simulink model "SwarmSystem"  (R2022b)
(part 2 of 4)

  Record : Record  RecordToWorkspace=on  FileSettingsInternal="{\"entries\":[{\"content\":{\"excelSettings\":{\"content\":{},\"type\":\"Streamout.ExcelSettings\"}},\"type\":\"Streamout.FileSettingStorage\",\"uuid\":\"ecd064a0-1818-44c3-a92e-bae1736691b7\"}],\"packageUris\":[\"http://schema.mathworks.com/mf0/streamout_blocks/R2020a\"],\"version\":\"1.0\"}"  SignalsInternal="{\"entries\":[{\"content\":{\"signals\":[{\"content\":{\"blockPath\":[\"SwarmSystem/Record\"],\"channel\":[],\"dimensions\":[54,1],\"domain\":\"SwarmSystem/Record\",\"hasChildren\":true,\"lineColor\":\"#fe330a\",\"plots\":[],\"port\":1,\"sid\":[\"\"],\"signalID\":5288,\"signalName\":\"z\"},\"type\":\"RecordBlkView.Signal\",\"uuid\":\"1048f33c-cd0c-4b1c-99d7-4ac97ea90ab0\"},{\"content\":{\"blockPath\":[\"SwarmSystem/Record\"],\"channel\":[1,1],\"dimensions\":[54,1],\"domain\":\"SwarmSystem/Record\",\"lineColor\":\"#7e2f8e\",\"parentID\":5288,\"plots\":[1],\"port\":1,\"sid\":[\"\"],\"signalID\":5289,\"signalName\":\"z\"},\"type\":\"RecordBlkView.Signal\",\"uuid\":\"d4620c93-bf21-47de-89ed-4dbaaf8b8520\"},{\"content\":{\"blockPath\":[\"SwarmSystem/Record\"],\"channel\":[],\"dimensions\":[36,1],\"domain\":\"SwarmSystem/Record\",\"hasChildren\":true,\"lineColor\":\"#0072bd\",\"plots\":[],\"port\":2,\"sid\":[\"\"],\"signalID\":5293,\"signalName\":\"z_d\"},\"type\":\"RecordBlkView.Signal\",\"uuid\":\"b35ab5d5-7ee7-45a1-a41b-38fccb067dc1\"},{\"content\":{\"blockPath\":[\"SwarmSystem/Record\"],\"channel\":[1,1],\"dimensions\":[36,1],\"domain\":\"SwarmSystem/Record\",\"lineColor\":\"#77ac30\",\"parentID\":5293,\"plots\":[1],\"port\":2,\"sid\":[\"\"],\"signalID\":5294,\"signalName\":\"z_d\"},\"type\":\"RecordBlkView.Signal\",\"uuid\":\"879ab91b-c74b-4204-85a0-6ebafe84b3f1\"},{\"content\":{\"blockPath\":[\"SwarmSystem/Record\"],\"channel\":[],\"dimensions\":[9,1],\"domain\":\"SwarmSystem/Record\",\"hasChildren\":true,\"lineColor\":\"#edb120\",\"plots\":[],\"port\":3,\"sid\":[\"\"],\"signalID\":5298,\"signalName\":\"Z_esp\"},\"type\":\"RecordBlkView.Signal\",\"uuid\":\"96b793c3-32b0-46bc-a925-f10905e3ac7d\"},{\"content\":{\"blockPath\":[\"SwarmSystem/Record\"],\"channel\":[1,1],\"dimensions\":[9,1],\"domain\":\"SwarmSystem/Record\",\"lineColor\":\"#64d413\",\"parentID\":5298,\"plots\":[1],\"port\":3,\"sid\":[\"\"],\"signalID\":5299,\"signalName\":\"Z_esp\"},\"type\":\"RecordBlkView.Signal\",\"uuid\":\"46fa4c9b-8c9c-4ead-9f2c-4953bb52642d\"},{\"content\":{\"blockPath\":[\"SwarmSystem/Record\"],\"channel\":[],\"dimensions\":[1],\"domain\":\"SwarmSystem/Record\",\"lineColor\":\"#ff6929\",\"plots\":[1],\"port\":4,\"sid\":[\"\"],\"signalID\":5303,\"signalName\":\"increment\"},\"type\":\"RecordBlkView.Signal\",\"uuid\":\"5359e2d5-ef0a-482c-b34d-73c89588b715\"},{\"content\":{\"blockPath\":[\"SwarmSystem/Record\"],\"channel\":[],\"dimensions\":[9,4],\"domain\":\"SwarmSystem/Record\",\"hasChildren\":true,\"lineColor\":\"#4dbeee\",\"plots\":[],\"port\":5,\"sid\":[\"\"],\"signalID\":5307,\"signalName\":\"bounds\"},\"type\":\"RecordBlkView.Signal\",\"uuid\":\"1b31fc5b-037d-49c7-bff4-18edc4567836\"},{\"content\":{\"blockPath\":[\"SwarmSystem/Record\"],\"channel\":[1,1],\"dimensions\":[9,4],\"domain\":\"SwarmSystem/Record\",\"lineColor\":\"#22b573\",\"parentID\":5307,\"plots\":[1],\"port\":5,\"sid\":[\"\"],\"signalID\":5308,\"signalName\":\"bounds\"},\"type\":\"RecordBlkView.Signal\",\"uuid\":\"eb4c524e-ff5c-4dd1-a222-fb6ffedcee01\"},{\"content\":{\"blockPath\":[\"SwarmSystem/Record\"],\"channel\":[],\"dimensions\":[1],\"domain\":\"SwarmSystem/Record\",\"lineColor\":\"#64d413\",\"plots\":[1],\"port\":6,\"sid\":[\"\"],\"signalID\":5312,\"signalName\":\"time\"},\"type\":\"RecordBlkView.Signal\",\"uuid\":\"72dfbc7d-692b-40af-bae7-eb77a350f7e6\"},{\"content\":{\"blockPath\":[\"SwarmSystem/Record\"],\"channel\":[],\"dimensions\":[9,27],\"domain\":\"SwarmSystem/Record\",\"hasChildren\":true,\"lineColor\":\"#ff6929\",\"plots\":[],\"port\":7,\"sid\":[\"\"],\"signalID\":5316,\"signalName\":\"raw\"},\"type\":\"RecordBlkView.Signal\",\"uuid\":\"f96d5ccb-5004-4439-9612-791f3ef51b61\"},{\"content\":{\"blockPath\":[\"SwarmSystem/Record\"],\"channel\":[1,1],\"dimensions\":[9,27],\"domain\":\"SwarmSystem/Record\",\"lineColor\":\"#edb120\",\"parentID\":5316,\"plots\":[1],\"port\":7,\"sid\":[\"\"],\"signalID\":5317,\"signalName\":\"raw\"},\"type\":\"RecordBlkView.Signal\",\"uuid\":\"bfe1e9cf-bb17-4b73-b5c0-09a8e8591fff\"},{\"content\":{\"blockPath\":[\"SwarmSystem/Record\"],\"channel\":[],\"dimensions\":[9,1],\"domain\":\"SwarmSystem/Record\",\"hasChildren\":true,\"lineColor\":\"#64d413\",\"plots\":[],\"port\":8,\"sid\":[\"\"],\"signalID\":5321,\"signalName\":\"sat_order\"},\"type\":\"RecordBlkView.Signal\",\"uuid\":\"3c0b71d5-5553-4668-91be-6a5fb8ab4b43\"},{\"content\":{\"blockPath\":[\"SwarmSystem/Record\"],\"channel\":[1,1],\"dimensions\":[9,1],\"domain\":\"SwarmSystem/Record\",\"lineColor\":\"#77ac30\",\"parentID\":5321,\"plots\":[1],\"port\":8,\"sid\":[\"\"],\"signalID\":5322,\"signalName\":\"sat_order\"},\"type\":\"RecordBlkView.Signal\",\"uuid\":\"ccf7dce6-4af8-4663-9d88-9176ee7af16e\"},{\"content\":{\"blockPath\":[\"SwarmSystem/Record\"],\"channel\":[],\"dimensions\":[9,9,3],\"domain\":\"SwarmSystem/Record\",\"hasChildren\":true,\"lineColor\":\"#fe330a\",\"plots\":[],\"port\":9,\"sid\":[\"\"],\"signalID\":5326,\"signalName\":\"packed_tw\"},\"type\":\"RecordBlkView.Signal\",\"uuid\":\"04cd0336-9984-42b6-950b-aadca579e03d\"},{\"content\":{\"blockPath\":[\"SwarmSystem/Record\"],\"channel\":[1,1,1],\"dimensions\":[9,9,3],\"domain\":\"SwarmSystem/Record\",\"lineColor\":\"#a2142f\",\"parentID\":5326,\"plots\":[1],\"port\":9,\"sid\":[\"\"],\"signalID\":5327,\"signalName\":\"packed_tw\"},\"type\":\"RecordBlkView.Signal\",\"uuid\":\"538a1e68-288b-4ad8-b1d1-6395bf7ee774\"},{\"content\":{\"blockPath\":[\"SwarmSystem/Record\"],\"channel\":[],\"dimensions\":[9,9,3,3],\"domain\":\"SwarmSystem/Record\",\"hasChildren\":true,\"lineColor\":\"#0072bd\",\"plots\":[],\"port\":10,\"sid\":[\"\"],\"signalID\":5331,\"signalName\":\"packed_intersections\"},\"type\":\"RecordBlkView.Signal\",\"uuid\":\"144e32b6-4e64-4aac-921a-80a3c9570e69\"},{\"content\":{\"blockPath\":[\"SwarmSystem/Record\"],\"channel\":[1,1,1,1],\"dimensions\":[9,9,3,3],\"domain\":\"SwarmSystem/Record\",\"lineColor\":\"#139fff\",\"parentID\":5331,\"plots\":[1],\"port\":10,\"sid\":[\"\"],\"signalID\":5332,\"signalName\":\"packed_intersections\"},\"type\":\"RecordBlkView.Signal\",\"uuid\":\"e33d14f4-2dcf-4038-900f-7b110429d0f7\"},{\"content\":{\"blockPath\":[\"SwarmSystem/Record\"],\"channel\":[2,1],\"dimensions\":[54,1],\"domain\":\"SwarmSystem/Record\",\"lineColor\":\"#64d413\",\"parentID\":5288,\"plots\":[1],\"port\":1,\"sid\":[\"\"],\"signalID\":5337,\"signalName\":\"z\"},\"type\":\"RecordBlkView.Signal\",\"uuid\":\"94ff7854-8769-4ec7-b8e0-c41f290a7d05\"},{\"content\":{\"blockPath\":[\"SwarmSystem/Record\"],\"channel\":[3,1],\"dimensions\":[54,1],\"domain\":\"SwarmSystem/Record\",\"lineColor\":\"#ff13a6\",\"parentID\":5288,\"plots\":[1],\"port\":1,\"sid\":[\"\"],\"signalID\":5338,\"signalName\":\"z\"},\"type\":\"RecordBlkView.Signal\",\"uuid\":\"55582deb-032f-45c7-978e-d388079c41d4\"},{\"content\":{\"blockPath\":[\"SwarmSystem/Record\"],\"channel\":[4,1],\"dimensions\":[54,1],\"domain\":\"SwarmSystem/Record\",\"lineColor\":\"#fe330a\",\"parentID\":5288,\"plots\":[1],\"port\":1,\"sid\":[\"\"],\"signalID\":5339,\"signalName\":\"z\"},\"type\":\"RecordBlkView.Signal\",\"uuid\":\"c5e6b669-41d4-4e1e-a17b-50be0138714a\"},{\"content\":{\"blockPath\":[\"SwarmSystem/Record\"],\"channel\":[5,1],\"dimensions\":[54,1],\"domain\":\"SwarmSystem/Record\",\"lineColor\":\"#22b573\",\"parentID\":5288,\"plots\":[],\"port\":1,\"sid\":[\"\"],\"signalID\":5340,\"signalName\":\"z\"},\"type\":\"RecordBlkView.Signal\",\"uuid\":\"b4ce17a2-064b-424c-b87d-5e710a343d57\"},{\"content\":{\"blockPath\":[\"SwarmSystem/Record\"],\"channel\":[6,1],\"dimensions\":[54,1],\"domain\":\"SwarmSystem/Record\",\"lineColor\":\"#0072bd\",\"parentID\":5288,\"plots\":[],\"port\":1,\"sid\":[\"\"],\"signalID\":5341,\"signalName\":\"z\"},\"type\":\"RecordBlkView.Signal\",\"uuid\":\"f998aeda-c207-47e4-835e-c5bd924f8b22\"},{\"content\":{\"blockPath\":[\"SwarmSystem/Record\"],\"channel\":[7,1],\"dimensions\":[54,1],\"domain\":\"SwarmSystem/Record\",\"lineColor\":\"#d95319\",\"parentID\":5288,\"plots\":[],\"port\":1,\"sid\":[\"\"],\"signalID\":5342,\"signalName\":\"z\"},\"type\":\"RecordBlkView.Signal\",\"uuid\":\"33bed8e9-bcc4-478e-8b0a-051153d0a6e0\"},{\"content\":{\"blockPath\":[\"SwarmSystem/Record\"],\"channel\":[8,1],\"dimensions\":[54,1],\"domain\":\"SwarmSystem/Record\",\"lineColor\":\"#edb120\",\"parentID\":5288,\"plots\":[],\"port\":1,\"sid\":[\"\"],\"signalID\":5343,\"signalName\":\"z\"},\"type\":\"RecordBlkView.Signal\",\"uuid\":\"23367080-42e0-4bda-822e-26e9880913c3\"},{\"content\":{\"blockPath\":[\"SwarmSystem/Record\"],\"channel\":[9,1],\"dimensions\":[54,1],\"domain\":\"SwarmSystem/Record\",\"lineColor\":\"#7e2f8e\",\"parentID\":5288,\"plots\":[],\"port\":1,\"sid\":[\"\"],\"signalID\":5344,\"signalName\":\"z\"},\"type\":\"RecordBlkView.Signal\",\"uuid\":\"666db174-2bf7-46d0-8a11-19612ed523fd\"},{\"content\":{\"blockPath\":[\"SwarmSystem/Record\"],\"channel\":[10,1],\"dimensions\":[54,1],\"domain\":\"SwarmSystem/Record\",\"lineColor\":\"#77ac30\",\"parentID\":5288,\"plots\":[],\"port\":1,\"sid\":[\"\"],\"signalID\":5345,\"signalName\":\"z\"},\"type\":\"RecordBlkView.Signal\",\"uuid\":\"d56b95aa-f617-4b7e-b38c-c508357e2a07\"},{\"content\":{\"blockPath\":[\"SwarmSystem/Record\"],\"channel\":[11,1],\"dimensions\":[54,1],\"domain\":\"SwarmSystem/Record\",\"lineColor\":\"#4dbeee\",\"parentID\":5288,\"plots\":[],\"port\":1,\"sid\":[\"\"],\"signalID\":5346,\"signalName\":\"z\"},\"type\":\"RecordBlkView.Signal\",\"uuid\":\"3c739fc7-8c37-4b5e-bb88-9d6524bd94ac\"},{\"content\":{\"blockPath\":[\"SwarmSystem/Record\"],\"channel\":[12,1],\"dimensions\":[54,1],\"domain\":\"SwarmSystem/Record\",\"lineColor\":\"#a2142f\",\"parentID\":5288,\"plots\":[],\"port\":1,\"sid\":[\"\"],\"signalID\":5347,\"signalName\":\"z\"},\"type\":\"RecordBlkView.Signal\",\"uuid\":\"2aa2a071-04ed-43fe-bed0-8f31fcee10da\"},{\"content\":{\"blockPath\":[\"SwarmSystem/Record\"],\"channel\":[13,1],\"dimensions\":[54,1],\"domain\":\"SwarmSystem/Record\",\"lineColor\":\"#139fff\",\"parentID\":5288,\"plots\":[],\"port\":1,\"sid\":[\"\"],\"signalID\":5348,\"signalName\":\"z\"},\"type\":\"RecordBlkView.Signal\",\"uuid\":\"af55a24b-ba08-4c59-88b6-de72df1b84e0\"},{\"content\":{\"blockPath\":[\"SwarmSystem/Record\"],\"channel\":[14,1],\"dimensions\":[54,1],\"domain\":\"SwarmSystem/Record\",\"lineColor\":\"#ff6929\",\"parentID\":5288,\"plots\":[],\"port\":1,\"sid\":[\"\"],\"signalID\":5349,\"signalName\":\"z\"},\"type\":\"RecordBlkView.Signal\",\"uuid\":\"1a6bf3ba-172b-41ef-a20a-2928397536b8\"},{\"content\":{\"blockPath\":[\"SwarmSystem/Record\"],\"channel\":[15,1],\"dimensions\":[54,1],\"domain\":\"SwarmSystem/Record\",\"lineColor\":\"#b746ff\",\"parentID\":5288,\"plots\":[],\"port\":1,\"sid\":[\"\"],\"signalID\":5350,\"signalName\":\"z\"},\"type\":\"RecordBlkView.Signal\",\"uuid\":\"cbf6ef62-eef2-4671-ba0b-33c28c49ded4\"},{\"content\":{\"blockPath\":[\"SwarmSystem/Record\"],\"channel\":[16,1],\"dimensions\":[54,1],\"domain\":\"SwarmSystem/Record\",\"lineColor\":\"#64d413\",\"parentID\":5288,\"plots\":[],\"port\":1,\"sid\":[\"\"],\"signalID\":5351,\"signalName\":\"z\"},\"type\":\"RecordBlkView.Signal\",\"uuid\":\"60424ef6-59ac-4762-8308-f2e8899aee2f\"},{\"content\":{\"blockPath\":[\"SwarmSystem/Record\"],\"channel\":[17,1],\"dimensions\":[54,1],\"domain\":\"SwarmSystem/Record\",\"lineColor\":\"#ff13a6\",\"parentID\":5288,\"plots\":[],\"port\":1,\"sid\":[\"\"],\"signalID\":5352,\"signalName\":\"z\"},\"type\":\"RecordBlkView.Signal\",\"uuid\":\"693ba6bc-14a8-4cd8-ab9b-fb1a45bae915\"},{\"content\":{\"blockPath\":[\"SwarmSystem/Record\"],\"channel\":[18,1],\"dimensions\":[54,1],\"domain\":\"SwarmSystem/Record\",\"lineColor\":\"#fe330a\",\"parentID\":5288,\"plots\":[],\"port\":1,\"sid\":[\"\"],\"signalID\":5353,\"signalName\":\"z\"},\"type\":\"RecordBlkView.Signal\",\"uuid\":\"85c5cfdb-b89a-4d6f-846d-6d1b25df3ce5\"},{\"content\":{\"blockPath\":[\"SwarmSystem/Record\"],\"channel\":[19,1],\"dimensions\":[54,1],\"domain\":\"SwarmSystem/Record\",\"lineColor\":\"#22b573\",\"parentID\":5288,\"plots\":[],\"port\":1,\"sid\":[\"\"],\"signalID\":5354,\"signalName\":\"z\"},\"type\":\"RecordBlkView.Signal\",\"uuid\":\"a606537b-4093-4b5b-8ba0-a895a02fc9ad\"},{\"content\":{\"blockPath\":[\"SwarmSystem/Record\"],\"channel\":[20,1],\"dimensions\":[54,1],\"domain\":\"SwarmSystem/Record\",\"lineColor\":\"#0072bd\",\"parentID\":5288,\"plots\":[],\"port\":1,\"sid\":[\"\"],\"signalID\":5355,\"signalName\":\"z\"},\"type\":\"RecordBlkView.Signal\",\"uuid\":\"d92b94f0-0096-476a-8397-e0938e33775d\"},{\"content\":{\"blockPath\":[\"SwarmSystem/Record\"],\"channel\":[21,1],\"dimensions\":[54,1],\"domain\":\"SwarmSystem/Record\",\"lineColor\":\"#d95319\",\"parentID\":5288,\"plots\":[],\"port\":1,\"sid\":[\"\"],\"signalID\":5356,\"signalName\":\"z\"},\"type\":\"RecordBlkView.Signal\",\"uuid\":\"53771d3f-3b29-417b-8dfe-8d61cc1d6a74\"},{\"content\":{\"blockPath\":[\"SwarmSystem/Record\"],\"channel\":[22,1],\"dimensions\":[54,1],\"domain\":\"SwarmSystem/Record\",\"lineColor\":\"#edb120\",\"parentID\":5288,\"plots\":[],\"port\":1,\"sid\":[\"\"],\"signalID\":5357,\"signalName\":\"z\"},\"type\":\"RecordBlkView.Signal\",\"uuid\":\"77a86afe-249a-40e4-933a-6b90270a3c5f\"},{\"content\":{\"blockPath\":[\"SwarmSystem/Record\"],\"channel\":[23,1],\"dimensions\":[54,1],\"domain\":\"SwarmSystem/Record\",\"lineColor\":\"#7e2f8e\",\"parentID\":5288,\"plots\":[],\"port\":1,\"sid\":[\"\"],\"signalID\":5358,\"signalName\":\"z\"},\"type\":\"RecordBlkView.Signal\",\"uuid\":\"71145ac7-7da5-4009-917a-f802b7d56a90\"},{\"content\":{\"blockPath\":[\"SwarmSystem/Record\"],\"channel\":[24,1],\"dimensions\":[54,1],\"domain\":\"SwarmSystem/Record\",\"lineColor\":\"#77ac30\",\"parentID\":5288,\"plots\":[],\"port\":1,\"sid\":[\"\"],\"signalID\":5359,\"signalName\":\"z\"},\"type\":\"RecordBlkView.Signal\",\"uuid\":\"a1777b40-0222-4109-b320-ffa96848db97\"},{\"content\":{\"blockPath\":[\"SwarmSystem/Record\"],\"channel\":[25,1],\"dimensions\":[54,1],\"domain\":\"SwarmSystem/Record\",\"lineColor\":\"#4dbeee\",\"parentID\":5288,\"plots\":[],\"port\":1,\"sid\":[\"\"],\"signalID\":5360,\"signalName\":\"z\"},\"type\":\"RecordBlkView.Signal\",\"uuid\":\"f0aa7a69-251b-47b1-b73c-85a4efe9d20c\"},{\"content\":{\"blockPath\":[\"SwarmSystem/Record\"],\"channel\":[26,1],\"dimensions\":[54,1],\"domain\":\"SwarmSystem/Record\",\"lineColor\":\"#a2142f\",\"parentID\":5288,\"plots\":[],\"port\":1,\"sid\":[\"\"],\"signalID\":5361,\"signalName\":\"z\"},\"type\":\"RecordBlkView.Signal\",\"uuid\":\"651f1bdc-b6dc-49af-bcc7-1437cdcaa17a\"},{\"content\":{\"blockPath\":[\"SwarmSystem/Record\"],\"channel\":[27,1],\"dimensions\":[54,1],\"domain\":\"SwarmSystem/Record\",\"lineColor\":\"#139fff\",\"parentID\":5288,\"plots\":[],\"port\":1,\"sid\":[\"\"],\"signalID\":5362,\"signalName\":\"z\"},\"type\":\"RecordBlkView.Signal\",\"uuid\":\"b7136c86-a499-4bc3-8659-50e8c5b58c3e\"},{\"content\":{\"blockPath\":[\"SwarmSystem/Record\"],\"channel\":[28,1],\"dimensions\":[54,1],\"domain\":\"SwarmSystem/Record\",\"lineColor\":\"#ff6929\",\"parentID\":5288,\"plots\":[],\"port\":1,\"sid\":[\"\"],\"signalID\":5363,\"signalName\":\"z\"},\"type\":\"RecordBlkView.Signal\",\"uuid\":\"39ed0c79-0ead-4119-98ea-487db81751da\"},{\"content\":{\"blockPath\":[\"SwarmSystem/Record\"],\"channel\":[29,1],\"dimensions\":[54,1],\"domain\":\"SwarmSystem/Record\",\"lineColor\":\"#b746ff\",\"parentID\":5288,\"plots\":[],\"port\":1,\"sid\":[\"\"],\"signalID\":5364,\"signalName\":\"z\"},\"type\":\"RecordBlkView.Signal\",\"uuid\":\"eab1f46b-145f-4fba-b506-cef354494f10\"},{\"content\":{\"blockPath\":[\"SwarmSystem/Record\"],\"channel\":[30,1],\"dimensions\":[54,1],\"domain\":\"SwarmSystem/Record\",\"lineColor\":\"#64d413\",\"parentID\":5288,\"plots\":[],\"port\":1,\"sid\":[\"\"],\"signalID\":5365,\"signalName\":\"z\"},\"type\":\"RecordBlkView.Signal\",\"uuid\":\"7bb013dd-5e1d-44ea-99f4-ae20af2f8ed1\"},{\"content\":{\"blockPath\":[\"SwarmSystem/Record\"],\"channel\":[31,1],\"dimensions\":[54,1],\"domain\":\"SwarmSystem/Record\",\"lineColor\":\"#ff13a6\",\"parentID\":5288,\"plots\":[],\"port\":1,\"sid\":[\"\"],\"signalID\":5366,\"signalName\":\"z\"},\"type\":\"RecordBlkView.Signal\",\"uuid\":\"bcc6f70b-8549-4e7b-8798-9fe58ee725e6\"},{\"content\":{\"blockPath\":[\"SwarmSystem/Record\"],\"channel\":[32,1],\"dimensions\":[54,1],\"domain\":\"SwarmSystem/Record\",\"lineColor\":\"#fe330a\",\"parentID\":5288,\"plots\":[],\"port\":1,\"sid\":[\"\"],\"signalID\":5367,\"signalName\":\"z\"},\"type\":\"RecordBlkView.Signal\",\"uuid\":\"1d770efc-4041-4ff2-a64a-e334b80ba3c3\"},{\"content\":{\"blockPath\":[\"SwarmSystem/Record\"],\"channel\":[33,1],\"dimensions\":[54,1],\"domain\":\"SwarmSystem/Record\",\"lineColor\":\"#22b573\",\"parentID\":5288,\"plots\":[],\"port\":1,\"sid\":[\"\"],\"signalID\":5368,\"signalName\":\"z\"},\"type\":\"RecordBlkView.Signal\",\"uuid\":\"4affd0bd-477a-4ba8-927f-f2cd7de50b25\"},{\"content\":{\"blockPath\":[\"SwarmSystem/Record\"],\"channel\":[34,1],\"dimensions\":[54,1],\"domain\":\"SwarmSystem/Record\",\"lineColor\":\"#0072bd\",\"parentID\":5288,\"plots\":[],\"port\":1,\"sid\":[\"\"],\"signalID\":5369,\"signalName\":\"z\"},\"type\":\"RecordBlkView.Signal\",\"uuid\":\"c22acc9d-ab4f-4cbd-ac54-90ec6f71b885\"},{\"content\":{\"blockPath\":[\"SwarmSystem/Record\"],\"channel\":[35,1],\"dimensions\":[54,1],\"domain\":\"SwarmSystem/Record\",\"lineColor\":\"#d95319\",\"parentID\":5288,\"plots\":[],\"port\":1,\"sid\":[\"\"],\"signalID\":5370,\"signalName\":\"z\"},\"type\":\"RecordBlkView.Signal\",\"uuid\":\"f21f0453-49be-4b57-8b6f-dc7b4bad43ed\"},{\"content\":{\"blockPath\":[\"SwarmSystem/Record\"],\"channel\":[36,1],\"dimensions\":[54,1],\"domain\":\"SwarmSystem/Record\",\"lineColor\":\"#edb120\",\"parentID\":5288,\"plots\":[],\"port\":1,\"sid\":[\"\"],\"signalID\":5371,\"signalName\":\"z\"},\"type\":\"RecordBlkView.Signal\",\"uuid\":\"ba2b707c-5274-442c-b398-eb6a9aecd37f\"},{\"content\":{\"blockPath\":[\"SwarmSystem/Record\"],\"channel\":[37,1],\"dimensions\":[54,1],\"domain\":\"SwarmSystem/Record\",\"lineColor\":\"#7e2f8e\",\"parentID\":5288,\"plots\":[],\"port\":1,\"sid\":[\"\"],\"signalID\":5372,\"signalName\":\"z\"},\"type\":\"RecordBlkView.Signal\",\"uuid\":\"831fb039-2951-49f2-8385-900d4bbd89fc\"},{\"content\":{\"blockPath\":[\"SwarmSystem/Record\"],\"channel\":[38,1],\"dimensions\":[54,1],\"domain\":\"SwarmSystem/Record\",\"lineColor\":\"#77ac30\",\"parentID\":5288,\"plots\":[],\"port\":1,\"sid\":[\"\"],\"signalID\":5373,\"signalName\":\"z\"},\"type\":\"RecordBlkView.Signal\",\"uuid\":\"90d9c7b8-1d8a-4815-aef9-0a30df0be531\"},{\"content\":{\"blockPath\":[\"SwarmSystem/Record\"],\"channel\":[39,1],\"dimensions\":[54,1],\"domain\":\"SwarmSystem/Record\",\"lineColor\":\"#4dbeee\",\"parentID\":5288,\"plots\":[],\"port\":1,\"sid\":[\"\"],\"signalID\":5374,\"signalName\":\"z\"},\"type\":\"RecordBlkView.Signal\",\"uuid\":\"9799df25-3ef0-4ed8-8f3d-b4132604c71d\"},{\"content\":{\"blockPath\":[\"SwarmSystem/Record\"],\"channel\":[40,1],\"dimensions\":[54,1],\"domain\":\"SwarmSystem/Record\",\"lineColor\":\"#a2142f\",\"parentID\":5288,\"plots\":[],\"port\":1,\"sid\":[\"\"],\"signalID\":5375,\"signalName\":\"z\"},\"type\":\"RecordBlkView.Signal\",\"uuid\":\"dec45052-4b04-4896-805d-0039b9c6ca05\"},{\"content\":{\"blockPath\":[\"SwarmSystem/Record\"],\"channel\":[41,1],\"dimensions\":[54,1],\"domain\":\"SwarmSystem/Record\",\"lineColor\":\"#139fff\",\"parentID\":5288,\"plots\":[],\"port\":1,\"sid\":[\"\"],\"signalID\":5376,\"signalName\":\"z\"},\"type\":\"RecordBlkView.Signal\",\"uuid\":\"b8df4f3a-df74-430c-8cdb-8f0728b2b91e\"},{\"content\":{\"blockPath\":[\"SwarmSystem/Record\"],\"channel\":[42,1],\"dimensions\":[54,1],\"domain\":\"SwarmSystem/Record\",\"lineColor\":\"#ff6929\",\"parentID\":5288,\"plots\":[],\"port\":1,\"sid\":[\"\"],\"signalID\":5377,\"signalName\":\"z\"},\"type\":\"RecordBlkView.Signal\",\"uuid\":\"39dc94a7-3cb9-4672-832e-c2db7ba2bcd7\"},{\"content\":{\"blockPath\":[\"SwarmSystem/Record\"],\"channel\":[43,1],\"dimensions\":[54,1],\"domain\":\"SwarmSystem/Record\",\"lineColor\":\"#b746ff\",\"parentID\":5288,\"plots\":[],\"port\":1,\"sid\":[\"\"],\"signalID\":5378,\"signalName\":\"z\"},\"type\":\"RecordBlkView.Signal\",\"uuid\":\"78f51d03-48e9-4910-84a7-c0792751e066\"},{\"content\":{\"blockPath\":[\"SwarmSystem/Record\"],\"channel\":[44,1],\"dimensions\":[54,1],\"domain\":\"SwarmSystem/Record\",\"lineColor\":\"#64d413\",\"parentID\":5288,\"plots\":[],\"port\":1,\"sid\":[\"\"],\"signalID\":5379,\"signalName\":\"z\"},\"type\":\"RecordBlkView.Signal\",\"uuid\":\"339c4194-65bc-4b35-aa4c-31d97d9926b8\"},{\"content\":{\"blockPath\":[\"SwarmSystem/Record\"],\"channel\":[45,1],\"dimensions\":[54,1],\"domain\":\"SwarmSystem/Record\",\"lineColor\":\"#ff13a6\",\"parentID\":5288,\"plots\":[],\"port\":1,\"sid\":[\"\"],\"signalID\":5380,\"signalName\":\"z\"},\"type\":\"RecordBlkView.Signal\",\"uuid\":\"af2a39ef-6094-4161-a88e-ca0071895a46\"},{\"content\":{\"blockPath\":[\"SwarmSystem/Record\"],\"channel\":[46,1],\"dimensions\":[54,1],\"domain\":\"SwarmSystem/Record\",\"lineColor\":\"#fe330a\",\"parentID\":5288,\"plots\":[],\"port\":1,\"sid\":[\"\"],\"signalID\":5381,\"signalName\":\"z\"},\"type\":\"RecordBlkView.Signal\",\"uuid\":\"ae8eab17-77c8-4c86-9f14-48d6648080e7\"},{\"content\":{\"blockPath\":[\"SwarmSystem/Record\"],\"channel\":[47,1],\"dimensions\":[54,1],\"domain\":\"SwarmSystem/Record\",\"lineColor\":\"#22b573\",\"parentID\":5288,\"plots\":[],\"port\":1,\"sid\":[\"\"],\"signalID\":5382,\"signalName\":\"z\"},\"type\":\"RecordBlkView.Signal\",\"uuid\":\"26dc57d1-732c-4d69-ae65-dc4e0eb2fd82\"},{\"content\":{\"blockPath\":[\"SwarmSystem/Record\"],\"channel\":[48,1],\"dimensions\":[54,1],\"domain\":\"SwarmSystem/Record\",\"lineColor\":\"#0072bd\",\"parentID\":5288,\"plots\":[],\"port\":1,\"sid\":[\"\"],\"signalID\":5383,\"signalName\":\"z\"},\"type\":\"RecordBlkView.Signal\",\"uuid\":\"04faca2b-564c-410a-a9d2-fe02c1e70823\"},{\"content\":{\"blockPath\":[\"SwarmSystem/Record\"],\"channel\":[49,1],\"dimensions\":[54,1],\"domain\":\"SwarmSystem/Record\",\"lineColor\":\"#d95319\",\"parentID\":5288,\"plots\":[],\"port\":1,\"sid\":[\"\"],\"signalID\":5384,\"signalName\":\"z\"},\"type\":\"RecordBlkView.Signal\",\"uuid\":\"83647c91-4303-4fda-9e2d-26a488f11dea\"},{\"content\":{\"blockPath\":[\"SwarmSystem/Record\"],\"channel\":[50,1],\"dimensions\":[54,1],\"domain\":\"SwarmSystem/Record\",\"lineColor\":\"#edb120\",\"parentID\":5288,\"plots\":[],\"port\":1,\"sid\":[\"\"],\"signalID\":5385,\"signalName\":\"z\"},\"type\":\"RecordBlkView.Signal\",\"uuid\":\"03f6a380-016e-4216-9a48-1af47f7e0bd3\"},{\"content\":{\"blockPath\":[\"SwarmSystem/Record\"],\"channel\":[51,1],\"dimensions\":[54,1],\"domain\":\"SwarmSystem/Record\",\"lineColor\":\"#7e2f8e\",\"parentID\":5288,\"plots\":[],\"port\":1,\"sid\":[\"\"],\"signalID\":5386,\"signalName\":\"z\"},\"type\":\"RecordBlkView.Signal\",\"uuid\":\"d152e4f7-7824-4489-ac59-58450394e9b8\"},{\"content\":{\"blockPath\":[\"SwarmSystem/Record\"],\"channel\":[52,1],\"dimensions\":[54,1],\"domain\":\"SwarmSystem/Record\",\"lineColor\":\"#77ac30\",\"parentID\":5288,\"plots\":[],\"port\":1,\"sid\":[\"\"],\"signalID\":5387,\"signalName\":\"z\"},\"type\":\"RecordBlkView.Signal\",\"uuid\":\"05a6ea49-2243-4c44-9877-3d753f1c4ee4\"},{\"content\":{\"blockPath\":[\"SwarmSystem/Record\"],\"channel\":[53,1],\"dimensions\":[54,1],\"domain\":\"SwarmSystem/Record\",\"lineColor\":\"#4dbeee\",\"parentID\":5288,\"plots\":[],\"port\":1,\"sid\":[\"\"],\"signalID\":5388,\"signalName\":\"z\"},\"type\":\"RecordBlkView.Signal\",\"uuid\":\"1bfb2284-3345-4984-9abd-f75713d5b4e1\"},{\"content\":{\"blockPath\":[\"SwarmSystem/Record\"],\"channel\":[54,1],\"dimensions\":[54,1],\"domain\":\"SwarmSystem/Record\",\"lineColor\":\"#a2142f\",\"parentID\":5288,\"plots\":[],\"port\":1,\"sid\":[\"\"],\"signalID\":5389,\"signalName\":\"z\"},\"type\":\"RecordBlkView.Signal\",\"uuid\":\"7bf6cb09-48fa-4d7c-a526-9989ac41e1ab\"},{\"content\":{\"blockPath\":[\"SwarmSystem/Record\"],\"channel\":[2,1],\"dimensions\":[36,1],\"domain\":\"SwarmSystem/Record\",\"lineColor\":\"#64d413\",\"parentID\":5293,\"plots\":[1],\"port\":2,\"sid\":[\"\"],\"signalID\":5390,\"signalName\":\"z_d\"},\"type\":\"RecordBlkView.Signal\",\"uuid\":\"e6ffad00-47e6-44c5-9608-ae31daac614c\"},{\"content\":{\"blockPath\":[\"SwarmSystem/Record\"],\"channel\":[3,1],\"dimensions\":[36,1],\"domain\":\"SwarmSystem/Record\",\"lineColor\":\"#ff13a6\",\"parentID\":5293,\"plots\":[1],\"port\":2,\"sid\":[\"\"],\"signalID\":5391,\"signalName\":\"z_d\"},\"type\":\"RecordBlkView.Signal\",\"uuid\":\"44ba9ae9-0245-4a66-8daf-a3dadca5a04f\"},{\"content\":{\"blockPath\":[\"SwarmSystem/Record\"],\"channel\":[4,1],\"dimensions\":[36,1],\"domain\":\"SwarmSystem/Record\",\"lineColor\":\"#fe330a\",\"parentID\":5293,\"plots\":[1],\"port\":2,\"sid\":[\"\"],\"signalID\":5392,\"signalName\":\"z_d\"},\"type\":\"RecordBlkView.Signal\",\"uuid\":\"36089385-170c-4820-aa71-50234e608897\"},{\"content\":{\"blockPath\":[\"SwarmSystem/Record\"],\"channel\":[5,1],\"dimensions\":[36,1],\"domain\":\"SwarmSystem/Record\",\"lineColor\":\"#22b573\",\"parentID\":5293,\"plots\":[],\"port\":2,\"sid\":[\"\"],\"signalID\":5393,\"signalName\":\"z_d\"},\"type\":\"RecordBlkView.Signal\",\"uuid\":\"d7fedbb7-f7eb-4e94-b28f-c4b8c60d7dde\"},{\"content\":{\"blockPath\":[\"SwarmSystem/Record\"],\"channel\":[6,1],\"dimensions\":[36,1],\"domain\":\"SwarmSystem/Record\",\"lineColor\":\"#0072bd\",\"parentID\":5293,\"plots\":[],\"port\":2,\"sid\":[\"\"],\"signalID\":5394,\"signalName\":\"z_d\"},\"type\":\"RecordBlkView.Signal\",\"uuid\":\"83c7dab3-b63b-4400-b522-774f61500074\"},{\"content\":{\"blockPath\":[\"SwarmSystem/Record\"],\"channel\":[7,1],\"dimensions\":[36,1],\"domain\":\"SwarmSystem/Record\",\"lineColor\":\"#d95319\",\"parentID\":5293,\"plots\":[],\"port\":2,\"sid\":[\"\"],\"signalID\":5395,\"signalName\":\"z_d\"},\"type\":\"RecordBlkView.Signal\",\"uuid\":\"d16d4b52-3523-4664-831c-1d07c082ddf3\"},{\"content\":{\"blockPath\":[\"SwarmSystem/Record\"],\"channel\":[8,1],\"dimensions\":[36,1],\"domain\":\"SwarmSystem/Record\",\"lineColor\":\"#edb120\",\"parentID\":5293,\"plots\":[],\"port\":2,\"sid\":[\"\"],\"signalID\":5396,\"signalName\":\"z_d\"},\"type\":\"RecordBlkView.Signal\",\"uuid\":\"f9657ccd-e1e0-48dc-b8c4-e91d91aa60c7\"},{\"content\":{\"blockPath\":[\"SwarmSystem/Record\"],\"channel\":[9,1],\"dimensions\":[36,1],\"domain\":\"SwarmSystem/Record\",\"lineColor\":\"#7e2f8e\",\"parentID\":5293,\"plots\":[],\"port\":2,\"sid\":[\"\"],\"signalID\":5397,\"signalName\":\"z_d\"},\"type\":\"RecordBlkView.Signal\",\"uuid\":\"9ed915ae-2923-4b80-b19a-c18d6e896bd9\"},{\"content\":{\"blockPath\":[\"SwarmSystem/Record\"],\"channel\":[10,1],\"dimensions\":[36,1],\"domain\":\"SwarmSystem/Record\",\"lineColor\":\"#77ac30\",\"parentID\":5293,\"plots\":[],\"port\":2,\"sid\":[\"\"],\"signalID\":5398,\"signalName\":\"z_d\"},\"type\":\"RecordBlkView.Signal\",\"uuid\":\"19270124-259f-424a-a751-ea4a90353119\"},{\"content\":{\"blockPath\":[\"SwarmSystem/Record\"],\"channel\":[11,1],\"dimensions\":[36,1],\"domain\":\"SwarmSystem/Record\",\"lineColor\":\"#4dbeee\",\"parentID\":5293,\"plots\":[],\"port\":2,\"sid\":[\"\"],\"signalID\":5399,\"signalName\":\"z_d\"},\"type\":\"RecordBlkView.Signal\",\"uuid\":\"b17ccb88-70cf-418e-97ce-fdbbb2bad34c\"},{\"content\":{\"blockPath\":[\"SwarmSystem/Record\"],\"channel\":[12,1],\"dimensions\":[36,1],\"domain\":\"SwarmSystem/Record\",\"lineColor\":\"#a2142f\",\"parentID\":5293,\"plots\":[],\"port\":2,\"sid\":[\"\"],\"signalID\":5400,\"signalName\":\"z_d\"},\"type\":\"RecordBlkView.Signal\",\"uuid\":\"3c690c17-7384-4003-bf98-5619cc2d0882\"},{\"content\":{\"blockPath\":[\"SwarmSystem/Record\"],\"channel\":[13,1],\"dimensions\":[36,1],\"domain\":\"SwarmSystem/Record\",\"lineColor\":\"#139fff\",\"parentID\":5293,\"plots\":[],\"port\":2,\"sid\":[\"\"],\"signalID\":5401,\"signalName\":\"z_d\"},\"type\":\"RecordBlkView.Signal\",\"uuid\":\"436eb858-1c14-4db8-ada7-78a4ed3c5d13\"},{\"content\":{\"blockPath\":[\"SwarmSystem/Record\"],\"channel\":[14,1],\"dimensions\":[36,1],\"domain\":\"SwarmSystem/Record\",\"lineColor\":\"#ff6929\",\"parentID\":5293,\"plots\":[],\"port\":2,\"sid\":[\"\"],\"signalID\":5402,\"signalName\":\"z_d\"},\"type\":\"RecordBlkView.Signal\",\"uuid\":\"1fd58fa3-57d9-4772-a499-d0164f4918e9\"},{\"content\":{\"blockPath\":[\"SwarmSystem/Record\"],\"channel\":[15,1],\"dimensions\":[36,1],\"domain\":\"SwarmSystem/Record\",\"lineColor\":\"#b746ff\",\"parentID\":5293,\"plots\":[],\"port\":2,\"sid\":[\"\"],\"signalID\":5403,\"signalName\":\"z_d\"},\"type\":\"RecordBlkView.Signal\",\"uuid\":\"5e1a1b0e-a1eb-4a75-b12e-39a1195df81e\"},{\"content\":{\"blockPath\":[\"SwarmSystem/Record\"],\"channel\":[16,1],\"dimensions\":[36,1],\"domain\":\"SwarmSystem/Record\",\"lineColor\":\"#64d413\",\"parentID\":5293,\"plots\":[],\"port\":2,\"sid\":[\"\"],\"signalID\":5404,\"signalName\":\"z_d\"},\"type\":\"RecordBlkView.Signal\",\"uuid\":\"459590a6-1d58-4b97-8a13-dc290a6d4f8f\"},{\"content\":{\"blockPath\":[\"SwarmSystem/Record\"],\"channel\":[17,1],\"dimensions\":[36,1],\"domain\":\"SwarmSystem/Record\",\"lineColor\":\"#ff13a6\",\"parentID\":5293,\"plots\":[],\"port\":2,\"sid\":[\"\"],\"signalID\":5405,\"signalName\":\"z_d\"},\"type\":\"RecordBlkView.Signal\",\"uuid\":\"39256010-ca08-42e4-87c0-75cd97dcafbb\"},{\"content\":{\"blockPath\":[\"SwarmSystem/Record\"],\"channel\":[18,1],\"dimensions\":[36,1],\"domain\":\"SwarmSystem/Record\",\"lineColor\":\"#fe330a\",\"parentID\":5293,\"plots\":[],\"port\":2,\"sid\":[\"\"],\"signalID\":5406,\"signalName\":\"z_d\"},\"type\":\"RecordBlkView.Signal\",\"uuid\":\"ad86186a-5725-473b-a994-36fc7556a4eb\"},{\"content\":{\"blockPath\":[\"SwarmSystem/Record\"],\"channel\":[19,1],\"dimensions\":[36,1],\"domain\":\"SwarmSystem/Record\",\"lineColor\":\"#22b573\",\"parentID\":5293,\"plots\":[],\"port\":2,\"sid\":[\"\"],\"signalID\":5407,\"signalName\":\"z_d\"},\"type\":\"RecordBlkView.Signal\",\"uuid\":\"e64d3326-0bd0-4518-acf5-f3e472a7f7d2\"},{\"content\":{\"blockPath\":[\"SwarmSystem/Record\"],\"channel\":[20,1],\"dimensions\":[36,1],\"domain\":\"SwarmSystem/Record\",\"lineColor\":\"#0072bd\",\"parentID\":5293,\"plots\":[],\"port\":2,\"sid\":[\"\"],\"signalID\":5408,\"signalName\":\"z_d\"},\"type\":\"RecordBlkView.Signal\",\"uuid\":\"8b6c7e5d-7e13-4168-a4ee-1e5bd70a8f9f\"},{\"content\":{\"blockPath\":[\"SwarmSystem/Record\"],\"channel\":[21,1],\"dimensions\":[36,1],\"domain\":\"SwarmSystem/Record\",\"lineColor\":\"#d95319\",\"parentID\":5293,\"plots\":[],\"port\":2,\"sid\":[\"\"],\"signalID\":5409,\"signalName\":\"z_d\"},\"type\":\"RecordBlkView.Signal\",\"uuid\":\"da157f65-0df1-40e4-853f-1ac8138e1ae8\"},{\"content\":{\"blockPath\":[\"SwarmSystem/Record\"],\"channel\":[22,1],\"dimensions\":[36,1],\"domain\":\"SwarmSystem/Record\",\"lineColor\":\"#edb120\",\"parentID\":5293,\"plots\":[],\"port\":2,\"sid\":[\"\"],\"signalID\":5410,\"signalName\":\"z_d\"},\"type\":\"RecordBlkView.Signal\",\"uuid\":\"7220b0fb-8f77-48fe-a277-d5335d62cbdb\"},{\"content\":{\"blockPath\":[\"SwarmSystem/Record\"],\"channel\":[23,1],\"dimensions\":[36,1],\"domain\":\"SwarmSystem/Record\",\"lineColor\":\"#7e2f8e\",\"parentID\":5293,\"plots\":[],\"port\":2,\"sid\":[\"\"],\"signalID\":5411,\"signalName\":\"z_d\"},\"type\":\"RecordBlkView.Signal\",\"uuid\":\"5ad9214f-8711-4b7b-95d8-f6bd4679f385\"},{\"content\":{\"blockPath\":[\"SwarmSystem/Record\"],\"channel\":[24,1],\"dimensions\":[36,1],\"domain\":\"SwarmSystem/Record\",\"lineColor\":\"#77ac30\",\"parentID\":5293,\"plots\":[],\"port\":2,\"sid\":[\"\"],\"signalID\":5412,\"signalName\":\"z_d\"},\"type\":\"RecordBlkView.Signal\",\"uuid\":\"842212fc-6798-4f6c-a317-dee861ff2de8\"},{\"content\":{\"blockPath\":[\"SwarmSystem/Record\"],\"channel\":[25,1],\"dimensions\":[36,1],\"domain\":\"SwarmSystem/Record\",\"lineColor\":\"#4dbeee\",\"parentID\":5293,\"plots\":[],\"port\":2,\"sid\":[\"\"],\"signalID\":5413,\"signalName\":\"z_d\"},\"type\":\"RecordBlkView.Signal\",\"uuid\":\"3777c87a-4847-4f7e-a14c-31597a5c92c3\"},{\"content\":{\"blockPath\":[\"SwarmSystem/Record\"],\"channel\":[26,1],\"dimensions\":[36,1],\"domain\":\"SwarmSystem/Record\",\"lineColor\":\"#a2142f\",\"parentID\":5293,\"plots\":[],\"port\":2,\"sid\":[\"\"],\"signalID\":5414,\"signalName\":\"z_d\"},\"type\":\"RecordBlkView.Signal\",\"uuid\":\"7b149055-4c6b-4942-841e-572c487a8602\"},{\"content\":{\"blockPath\":[\"SwarmSystem/Record\"],\"channel\":[27,1],\"dimensions\":[36,1],\"domain\":\"SwarmSystem/Record\",\"lineColor\":\"#139fff\",\"parentID\":5293,\"plots\":[],\"port\":2,\"sid\":[\"\"],\"signalID\":5415,\"signalName\":\"z_d\"},\"type\":\"RecordBlkView.Signal\",\"uuid\":\"7e88c991-8eb0-4f52-9f61-7f872eb0643a\"},{\"content\":{\"blockPath\":[\"SwarmSystem/Record\"],\"channel\":[28,1],\"dimensions\":[36,1],\"domain\":\"SwarmSystem/Record\",\"lineColor\":\"#ff6929\",\"parentID\":5293,\"plots\":[],\"port\":2,\"sid\":[\"\"],\"signalID\":5416,\"signalName\":\"z_d\"},\"type\":\"RecordBlkView.Signal\",\"uuid\":\"2586847c-614d-447c-933c-274f485a1234\"},{\"content\":{\"blockPath\":[\"SwarmSystem/Record\"],\"channel\":[29,1],\"dimensions\":[36,1],\"domain\":\"SwarmSystem/Record\",\"lineColor\":\"#b746ff\",\"parentID\":5293,\"plots\":[],\"port\":2,\"sid\":[\"\"],\"signalID\":5417,\"signalName\":\"z_d\"},\"type\":\"RecordBlkView.Signal\",\"uuid\":\"4c61c48c-9707-4733-a8b0-73d5f49e8c48\"},{\"content\":{\"blockPath\":[\"SwarmSystem/Record\"],\"channel\":[30,1],\"dimensions\":[36,1],\"domain\":\"SwarmSystem/Record\",\"lineColor\":\"#64d413\",\"parentID\":5293,\"plots\":[],\"port\":2,\"sid\":[\"\"],\"signalID\":5418,\"signalName\":\"z_d\"},\"type\":\"RecordBlkView.Signal\",\"uuid\":\"f990fc59-8c50-4aa4-8cb1-7d556b47f12d\"},{\"content\":{\"blockPath\":[\"SwarmSystem/Record\"],\"channel\":[31,1],\"dimensions\":[36,1],\"domain\":\"SwarmSystem/Record\",\"lineColor\":\"#ff13a6\",\"parentID\":5293,\"plots\":[],\"port\":2,\"sid\":[\"\"],\"signalID\":5419,\"signalName\":\"z_d\"},\"type\":\"RecordBlkView.Signal\",\"uuid\":\"5f0dc818-7e48-461e-9198-0196acb0a9e2\"},{\"content\":{\"blockPath\":[\"SwarmSystem/Record\"],\"channel\":[32,1],\"dimensions\":[36,1],\"domain\":\"SwarmSystem/Record\",\"lineColor\":\"#fe330a\",\"parentID\":5293,\"plots\":[],\"port\":2,\"sid\":[\"\"],\"signalID\":5420,\"signalName\":\"z_d\"},\"type\":\"RecordBlkView.Signal\",\"uuid\":\"559fa93c-660d-4f4c-a164-18850e5b654a\"},{\"content\":{\"blockPath\":[\"SwarmSystem/Record\"],\"channel\":[33,1],\"dimensions\":[36,1],\"domain\":\"SwarmSystem/Record\",\"lineColor\":\"#22b573\",\"parentID\":5293,\"plots\":[],\"port\":2,\"sid\":[\"\"],\"signalID\":5421,\"signalName\":\"z_d\"},\"type\":\"RecordBlkView.Signal\",\"uuid\":\"aa3ca54a-f3fd-459f-afac-2a946a987f71\"},{\"content\":{\"blockPath\":[\"SwarmSystem/Record\"],\"channel\":[34,1],\"dimensions\":[36,1],\"domain\":\"SwarmSystem/Record\",\"lineColor\":\"#0072bd\",\"parentID\":5293,\"plots\":[],\"port\":2,\"sid\":[\"\"],\"signalID\":5422,\"signalName\":\"z_d\"},\"type\":\"RecordBlkView.Signal\",\"uuid\":\"8789ec61-cb83-42ac-902e-46e394537929\"},{\"content\":{\"blockPath\":[\"SwarmSystem/Record\"],\"channel\":[35,1],\"dimensions\":[36,1],\"domain\":\"SwarmSystem/Record\",\"lineColor\":\"#d95319\",\"parentID\":5293,\"plots\":[],\"port\":2,\"sid\":[\"\"],\"signalID\":5423,\"signalName\":\"z_d\"},\"type\":\"RecordBlkView.Signal\",\"uuid\":\"d855b270-3395-477d-a828-70e3bf4540aa\"},{\"content\":{\"blockPath\":[\"SwarmSystem/Record\"],\"channel\":[36,1],\"dimensions\":[36,1],\"domain\":\"SwarmSystem/Record\",\"lineColor\":\"#edb120\",\"parentID\":5293,\"plots\":[],\"port\":2,\"sid\":[\"\"],\"signalID\":5424,\"signalName\":\"z_d\"},\"type\":\"RecordBlkView.Signal\",\"uuid\":\"1808bf7e-7209-4d8b-bd54-e26db35cae74\"},{\"content\":{\"blockPath\":[\"SwarmSystem/Record\"],\"channel\":[2,1],\"dimensions\":[9,1],\"domain\":\"SwarmSystem/Record\",\"lineColor\":\"#b746ff\",\"parentID\":5298,\"plots\":[1],\"port\":3,\"sid\":[\"\"],\"signalID\":5425,\"signalName\":\"Z_esp\"},\"type\":\"RecordBlkView.Signal\",\"uuid\":\"18199f45-8004-4c58-a216-311efe8f1625\"},{\"content\":{\"blockPath\":[\"SwarmSystem/Record\"],\"channel\":[3,1],\"dimensions\":[9,1],\"domain\":\"SwarmSystem/Record\",\"lineColor\":\"#64d413\",\"parentID\":5298,\"plots\":[1],\"port\":3,\"sid\":[\"\"],\"signalID\":5426,\"signalName\":\"Z_esp\"},\"type\":\"RecordBlkView.Signal\",\"uuid\":\"db8fe98c-f2e4-442a-bc0e-7d3f97b53b9d\"},{\"content\":{\"blockPath\":[\"SwarmSystem/Record\"],\"channel\":[4,1],\"dimensions\":[9,1],\"domain\":\"SwarmSystem/Record\",\"lineColor\":\"#ff13a6\",\"parentID\":5298,\"plots\":[1],\"port\":3,\"sid\":[\"\"],\"signalID\":5427,\"signalName\":\"Z_esp\"},\"type\":\"RecordBlkView.Signal\",\"uuid\":\"9e4af2a5-3fa3-4881-8051-5e64c53ef745\"},{\"content\":{\"blockPath\":[\"SwarmSystem/Record\"],\"channel\":[5,1],\"dimensions\":[9,1],\"domain\":\"SwarmSystem/Record\",\"lineColor\":\"#fe330a\",\"parentID\":5298,\"plots\":[],\"port\":3,\"sid\":[\"\"],\"signalID\":5428,\"signalName\":\"Z_esp\"},\"type\":\"RecordBlkView.Signal\",\"uuid\":\"168ea0a2-e9ea-45e0-828b-1c992beb1d4b\"},{\"content\":{\"blockPath\":[\"SwarmSystem/Record\"],\"channel\":[6,1],\"dimensions\":[9,1],\"domain\":\"SwarmSystem/Record\",\"lineColor\":\"#22b573\",\"parentID\":5298,\"plots\":[],\"port\":3,\"sid\":[\"\"],\"signalID\":5429,\"signalName\":\"Z_esp\"},\"type\":\"RecordBlkView.Signal\",\"uuid\":\"95c494ce-366f-4dc5-8c8f-ed7ba7180eaf\"},{\"content\":{\"blockPath\":[\"SwarmSystem/Record\"],\"channel\":[7,1],\"dimensions\":[9,1],\"domain\":\"SwarmSystem/Record\",\"lineColor\":\"#0072bd\",\"parentID\":5298,\"plots\":[],\"port\":3,\"sid\":[\"\"],\"signalID\":5430,\"signalName\":\"Z_esp\"},\"type\":\"RecordBlkView.Signal\",\"uuid\":\"4d057111-4cea-4b96-9cb6-6430df8d72f0\"},{\"content\":{\"blockPath\":[\"SwarmSystem/Record\"],\"channel\":[8,1],\"dimensions\":[9,1],\"domain\":\"SwarmSystem/Record\",\"lineColor\":\"#d95319\",\"parentID\":5298,\"plots\":[],\"port\":3,\"sid\":[\"\"],\"signalID\":5431,\"signalName\":\"Z_esp\"},\"type\":\"RecordBlkView.Signal\",\"uuid\":\"df7e5dad-1f79-48f9-bf09-243d1f37aaf2\"},{\"content\":{\"blockPath\":[\"SwarmSystem/Record\"],\"channel\":[9,1],\"dimensions\":[9,1],\"domain\":\"SwarmSystem/Record\",\"lineColor\":\"#edb120\",\"parentID\":5298,\"plots\":[],\"port\":3,\"sid\":[\"\"],\"signalID\":5432,\"signalName\":\"Z_esp\"},\"type\":\"RecordBlkView.Signal\",\"uuid\":\"ca5538ee-6fc4-487a-b491-57dcd6f519e2\"},{\"content\":{\"blockPath\":[\"SwarmSystem/Record\"],\"channel\":[2,1],\"dimensions\":[9,4],\"domain\":\"SwarmSystem/Record\",\"lineColor\":\"#7e2f8e\",\"parentID\":5307,\"plots\":[1],\"port\":5,\"sid\":[\"\"],\"signalID\":5433,\"signalName\":\"bounds\"},\"type\":\"RecordBlkView.Signal\",\"uuid\":\"125f905b-501e-48a9-8957-05c43fcc3ba8\"},{\"content\":{\"blockPath\":[\"SwarmSystem/Record\"],\"channel\":[3,1],\"dimensions\":[9,4],\"domain\":\"SwarmSystem/Record\",\"lineColor\":\"#77ac30\",\"parentID\":5307,\"plots\":[1],\"port\":5,\"sid\":[\"\"],\"signalID\":5434,\"signalName\":\"bounds\"},\"type\":\"RecordBlkView.Signal\",\"uuid\":\"f516a14e-ac79-4100-bc21-44e65bbf6ade\"},{\"content\":{\"blockPath\":[\"SwarmSystem/Record\"],\"channel\":[4,1],\"dimensions\":[9,4],\"domain\":\"SwarmSystem/Record\",\"lineColor\":\"#4dbeee\",\"parentID\":5307,\"plots\":[1],\"port\":5,\"sid\":[\"\"],\"signalID\":5435,\"signalName\":\"bounds\"},\"type\":\"RecordBlkView.Signal\",\"uuid\":\"63176c5b-0ec0-4659-83b2-9c5b85541d97\"},{\"content\":{\"blockPath\":[\"SwarmSystem/Record\"],\"channel\":[5,1],\"dimensions\":[9,4],\"domain\":\"SwarmSystem/Record\",\"lineColor\":\"#a2142f\",\"parentID\":5307,\"plots\":[],\"port\":5,\"sid\":[\"\"],\"signalID\":5436,\"signalName\":\"bounds\"},\"type\":\"RecordBlkView.Signal\",\"uuid\":\"13022ac8-d0ce-43bd-8f5f-8be306c911e4\"},{\"content\":{\"blockPath\":[\"SwarmSystem/Record\"],\"channel\":[6,1],\"dimensions\":[9,4],\"domain\":\"SwarmSystem/Record\",\"lineColor\":\"#139fff\",\"parentID\":5307,\"plots\":[],\"port\":5,\"sid\":[\"\"],\"signalID\":5437,\"signalName\":\"bounds\"},\"type\":\"RecordBlkView.Signal\",\"uuid\":\"f73451aa-44cf-4581-9b6c-62a7e5a8527b\"},{\"content\":{\"blockPath\":[\"SwarmSystem/Record\"],\"channel\":[7,1],\"dimensions\":[9,4],\"domain\":\"SwarmSystem/Record\",\"lineColor\":\"#ff6929\",\"parentID\":5307,\"plots\":[],\"port\":5,\"sid\":[\"\"],\"signalID\":5438,\"signalName\":\"bounds\"},\"type\":\"RecordBlkView.Signal\",\"uuid\":\"d7a4bb58-77e8-48e9-8ec5-7c22dac4d9b9\"},{\"content\":{\"blockPath\":[\"SwarmSystem/Record\"],\"channel\":[8,1],\"dimensions\":[9,4],\"domain\":\"SwarmSystem/Record\",\"lineColor\":\"#b746ff\",\"parentID\":5307,\"plots\":[],\"port\":5,\"sid\":[\"\"],\"signalID\":5439,\"signalName\":\"bounds\"},\"type\":\"RecordBlkView.Signal\",\"uuid\":\"1e295cc8-670c-4f3c-bb50-da02e2d7ac70\"},{\"content\":{\"blockPath\":[\"SwarmSystem/Record\"],\"channel\":[9,1],\"dimensions\":[9,4],\"domain\":\"SwarmSystem/Record\",\"lineColor\":\"#64d413\",\"parentID\":5307,\"plots\":[],\"port\":5,\"sid\":[\"\"],\"signalID\":5440,\"signalName\":\"bounds\"},\"type\":\"RecordBlkView.Signal\",\"uuid\":\"485bb85b-3d89-4afc-9d02-7c08bc441512\"},{\"content\":{\"blockPath\":[\"SwarmSystem/Record\"],\"channel\":[1,2],\"dimensions\":[9,4],\"domain\":\"SwarmSystem/Record\",\"lineColor\":\"#ff13a6\",\"parentID\":5307,\"plots\":[],\"port\":5,\"sid\":[\"\"],\"signalID\":5441,\"signalName\":\"bounds\"},\"type\":\"RecordBlkView.Signal\",\"uuid\":\"cc2d4fdd-0103-4754-bdc4-849d74d63b0b\"},{\"content\":{\"blockPath\":[\"SwarmSystem/Record\"],\"channel\":[2,2],\"dimensions\":[9,4],\"domain\":\"SwarmSystem/Record\",\"lineColor\":\"#fe330a\",\"parentID\":5307,\"plots\":[],\"port\":5,\"sid\":[\"\"],\"signalID\":5442,\"signalName\":\"bounds\"},\"type\":\"RecordBlkView.Signal\",\"uuid\":\"0d65b822-d0fe-4ece-bbe3-7fc27c7789ec\"},{\"content\":{\"blockPath\":[\"SwarmSystem/Record\"],\"channel\":[3,2],\"dimensions\":[9,4],\"domain\":\"SwarmSystem/Record\",\"lineColor\":\"#22b573\",\"parentID\":5307,\"plots\":[],\"port\":5,\"sid\":[\"\"],\"signalID\":5443,\"signalName\":\"bounds\"},\"type\":\"RecordBlkView.Signal\",\"uuid\":\"5e42c46e-15ba-4487-a1a3-bf693d4e7caf\"},{\"content\":{\"blockPath\":[\"SwarmSystem/Record\"],\"channel\":[4,2],\"dimensions\":[9,4],\"domain\":\"SwarmSystem/Record\",\"lineColor\":\"#0072bd\",\"parentID\":5307,\"plots\":[],\"port\":5,\"sid\":[\"\"],\"signalID\":5444,\"signalName\":\"bounds\"},\"type\":\"RecordBlkView.Signal\",\"uuid\":\"6308b5c8-544e-4c8f-97f8-b4ccea8d23bc\"},{\"content\":{\"blockPath\":[\"SwarmSystem/Record\"],\"channel\":[5,2],\"dimensions\":[9,4],\"domain\":\"SwarmSystem/Record\",\"lineColor\":\"#d95319\",\"parentID\":5307,\"plots\":[],\"port\":5,\"sid\":[\"\"],\"signalID\":5445,\"signalName\":\"bounds\"},\"type\":\"RecordBlkView.Signal\",\"uuid\":\"649c3cd1-ff45-49cc-bf70-dce125ebbe61\"},{\"content\":{\"blockPath\":[\"SwarmSystem/Record\"],\"channel\":[6,2],\"dimensions\":[9,4],\"domain\":\"SwarmSystem/Record\",\"lineColor\":\"#edb120\",\"parentID\":5307,\"plots\":[],\"port\":5,\"sid\":[\"\"],\"signalID\":5446,\"signalName\":\"bounds\"},\"type\":\"RecordBlkView.Signal\",\"uuid\":\"973347cf-3ed4-4338-b02e-04b230b051e5\"},{\"content\":{\"blockPath\":[\"SwarmSystem/Record\"],\"channel\":[7,2],\"dimensions\":[9,4],\"domain\":\"SwarmSystem/Record\",\"lineColor\":\"#7e2f8e\",\"parentID\":5307,\"plots\":[],\"port\":5,\"sid\":[\"\"],\"signalID\":5447,\"signalName\":\"bounds\"},\"type\":\"RecordBlkView.Signal\",\"uuid\":\"7c6e30ea-61f1-4712-8ee8-76944592dbb4\"},{\"content\":{\"blockPath\":[\"SwarmSystem/Record\"],\"channel\":[8,2],\"dimensions\":[9,4],\"domain\":\"SwarmSystem/Record\",\"lineColor\":\"#77ac30\",\"parentID\":5307,\"plots\":[],\"port\":5,\"sid\":[\"\"],\"signalID\":5448,\"signalName\":\"bounds\"},\"type\":\"RecordBlkView.Signal\",\"uuid\":\"5afe3431-5563-4496-afb8-558e515896e6\"},{\"content\":{\"blockPath\":[\"SwarmSystem/Record\"],\"channel\":[9,2],\"dimensions\":[9,4],\"domain\":\"SwarmSystem/Record\",\"lineColor\":\"#4dbeee\",\"parentID\":5307,\"plots\":[],\"port\":5,\"sid\":[\"\"],\"signalID\":5449,\"signalName\":\"bounds\"},\"type\":\"RecordBlkView.Signal\",\"uuid\":\"695c100c-c8ed-4702-8f5d-2ffa71f0bece\"},{\"content\":{\"blockPath\":[\"SwarmSystem/Record\"],\"channel\":[1,3],\"dimensions\":[9,4],\"domain\":\"SwarmSystem/Record\",\"lineColor\":\"#a2142f\",\"parentID\":5307,\"plots\":[],\"port\":5,\"sid\":[\"\"],\"signalID\":5450,\"signalName\":\"bounds\"},\"type\":\"RecordBlkView.Signal\",\"uuid\":\"3f3bcd4a-d33f-4986-a0e4-f7f2ef915f6f\"},{\"content\":{\"blockPath\":[\"SwarmSystem/Record\"],\"channel\":[2,3],\"dimensions\":[9,4],\"domain\":\"SwarmSystem/Record\",\"lineColor\":\"#139fff\",\"parentID\":5307,\"plots\":[],\"port\":5,\"sid\":[\"\"],\"signalID\":5451,\"signalName\":\"bounds\"},\"type\":\"RecordBlkView.Signal\",\"uuid\":\"7867e7f6-0a8a-481f-b9f0-c9a116904b88\"},{\"content\":{\"blockPath\":[\"SwarmSystem/Record\"],\"channel\":[3,3],\"dimensions\":[9,4],\"domain\":\"SwarmSystem/Record\",\"lineColor\":\"#ff6929\",\"parentID\":5307,\"plots\":[],\"port\":5,\"sid\":[\"\"],\"signalID\":5452,\"signalName\":\"bounds\"},\"type\":\"RecordBlkView.Signal\",\"uuid\":\"1b9bd8dd-52b3-4184-b5bc-8f9686ec0241\"},{\"content\":{\"blockPath\":[\"SwarmSystem/Record\"],\"channel\":[4,3],\"dimensions\":[9,4],\"domain\":\"SwarmSystem/Record\",\"lineColor\":\"#b746ff\",\"parentID\":5307,\"plots\":[],\"port\":5,\"sid\":[\"\"],\"signalID\":5453,\"signalName\":\"bounds\"},\"type\":\"RecordBlkView.Signal\",\"uuid\":\"7893f70f-bc4d-454e-8afd-2867695fab9d\"},{\"content\":{\"blockPath\":[\"SwarmSystem/Record\"],\"channel\":[5,3],\"dimensions\":[9,4],\"domain\":\"SwarmSystem/Record\",\"lineColor\":\"#64d413\",\"parentID\":5307,\"plots\":[],\"port\":5,\"sid\":[\"\"],\"signalID\":5454,\"signalName\":\"bounds\"},\"type\":\"RecordBlkView.Signal\",\"uuid\":\"2c5ed339-b145-45a1-93da-cf48d75b49a8\"},{\"content\":{\"blockPath\":[\"SwarmSystem/Record\"],\"channel\":[6,3],\"dimensions\":[9,4],\"domain\":\"SwarmSystem/Record\",\"lineColor\":\"#ff13a6\",\"parentID\":5307,\"plots\":[],\"port\":5,\"sid\":[\"\"],\"signalID\":5455,\"signalName\":\"bounds\"},\"type\":\"RecordBlkView.Signal\",\"uuid\":\"09baf8ce-ccbf-44f7-817e-97d9b71431cd\"},{\"content\":{\"blockPath\":[\"SwarmSystem/Record\"],\"channel\":[7,3],\"dimensions\":[9,4],\"domain\":\"SwarmSystem/Record\",\"lineColor\":\"#fe330a\",\"parentID\":5307,\"plots\":[],\"port\":5,\"sid\":[\"\"],\"signalID\":5456,\"signalName\":\"bounds\"},\"type\":\"RecordBlkView.Signal\",\"uuid\":\"1891fa1e-9334-4e0e-b44a-74733c6a6662\"},{\"content\":{\"blockPath\":[\"SwarmSystem/Record\"],\"channel\":[8,3],\"dimensions\":[9,4],\"domain\":\"SwarmSystem/Record\",\"lineColor\":\"#22b573\",\"parentID\":5307,\"plots\":[],\"port\":5,\"sid\":[\"\"],\"signalID\":5457,\"signalName\":\"bounds\"},\"type\":\"RecordBlkView.Signal\",\"uuid\":\"efc0f182-cd3f-4258-9184-83edcec5bbae\"},{\"content\":{\"blockPath\":[\"SwarmSystem/Record\"],\"channel\":[9,3],\"dimensions\":[9,4],\"domain\":\"SwarmSystem/Record\",\"lineColor\":\"#0072bd\",\"parentID\":5307,\"plots\":[],\"port\":5,\"sid\":[\"\"],\"signalID\":5458,\"signalName\":\"bounds\"},\"type\":\"RecordBlkView.Signal\",\"uuid\":\"169f818e-1f0e-479a-83f7-70b4bcf25223\"},{\"content\":{\"blockPath\":[\"SwarmSystem/Record\"],\"channel\":[1,4],\"dimensions\":[9,4],\"domain\":\"SwarmSystem/Record\",\"lineColor\":\"#d95319\",\"parentID\":5307,\"plots\":[],\"port\":5,\"sid\":[\"\"],\"signalID\":5459,\"signalName\":\"bounds\"},\"type\":\"RecordBlkView.Signal\",\"uuid\":\"f37abeeb-2e55-4caa-b65c-e6e9b1123847\"},{\"content\":{\"blockPath\":[\"SwarmSystem/Record\"],\"channel\":[2,4],\"dimensions\":[9,4],\"domain\":\"SwarmSystem/Record\",\"lineColor\":\"#edb120\",\"parentID\":5307,\"plots\":[],\"port\":5,\"sid\":[\"\"],\"signalID\":5460,\"signalName\":\"bounds\"},\"type\":\"RecordBlkView.Signal\",\"uuid\":\"6616e42a-d444-4778-a974-d6cb74468ff8\"},{\"content\":{\"blockPath\":[\"SwarmSystem/Record\"],\"channel\":[3,4],\"dimensions\":[9,4],\"domain\":\"SwarmSystem/Record\",\"lineColor\":\"#7e2f8e\",\"parentID\":5307,\"plots\":[],\"port\":5,\"sid\":[\"\"],\"signalID\":5461,\"signalName\":\"bounds\"},\"type\":\"RecordBlkView.Signal\",\"uuid\":\"5735d483-26a8-4e2c-90a6-38f9ae2cc8a8\"},{\"content\":{\"blockPath\":[\"SwarmSystem/Record\"],\"channel\":[4,4],\"dimensions\":[9,4],\"domain\":\"SwarmSystem/Record\",\"lineColor\":\"#77ac30\",\"parentID\":5307,\"plots\":[],\"port\":5,\"sid\":[\"\"],\"signalID\":5462,\"signalName\":\"bounds\"},\"type\":\"RecordBlkView.Signal\",\"uuid\":\"5d65a8b1-4389-4d31-9d81-badae035207b\"},{\"content\":{\"blockPath\":[\"SwarmSystem/Record\"],\"channel\":[5,4],\"dimensions\":[9,4],\"domain\":\"SwarmSystem/Record\",\"lineColor\":\"#4dbeee\",\"parentID\":5307,\"plots\":[],\"port\":5,\"sid\":[\"\"],\"signalID\":5463,\"signalName\":\"bounds\"},\"type\":\"RecordBlkView.Signal\",\"uuid\":\"88f341b4-a7bf-40c7-9be6-138126c8dce8\"},{\"content\":{\"blockPath\":[\"SwarmSystem/Record\"],\"channel\":[6,4],\"dimensions\":[9,4],\"domain\":\"SwarmSystem/Record\",\"lineColor\":\"#a2142f\",\"parentID\":5307,\"plots\":[],\"port\":5,\"sid\":[\"\"],\"signalID\":5464,\"signalName\":\"bounds\"},\"type\":\"RecordBlkView.Signal\",\"uuid\":\"9a701720-d2bf-4152-9b7f-1f7c856be2ed\"},{\"content\":{\"blockPath\":[\"SwarmSystem/Record\"],\"channel\":[7,4],\"dimensions\":[9,4],\"domain\":\"SwarmSystem/Record\",\"lineColor\":\"#139fff\",\"parentID\":5307,\"plots\":[],\"port\":5,\"sid\":[\"\"],\"signalID\":5465,\"signalName\":\"bounds\"},\"type\":\"RecordBlkView.Signal\",\"uuid\":\"2ee111bc-1ea0-4da4-9391-bd825f7ddcd7\"},{\"content\":{\"blockPath\":[\"SwarmSystem/Record\"],\"channel\":[8,4],\"dimensions\":[9,4],\"domain\":\"SwarmSystem/Record\",\"lineColor\":\"#ff6929\",\"parentID\":5307,\"plots\":[],\"port\":5,\"sid\":[\"\"],\"signalID\":5466,\"signalName\":\"bounds\"},\"type\":\"RecordBlkView.Signal\",\"uuid\":\"b93ff484-75e9-43d5-a090-7d3595ab4b79\"},{\"content\":{\"blockPath\":[\"SwarmSystem/Record\"],\"channel\":[9,4],\"dimensions\":[9,4],\"domain\":\"SwarmSystem/Record\",\"lineColor\":\"#b746ff\",\"parentID\":5307,\"plots\":[],\"port\":5,\"sid\":[\"\"],\"signalID\":5467,\"signalName\":\"bounds\"},\"type\":\"RecordBlkView.Signal\",\"uuid\":\"6ef4f7c0-2752-4fa1-a232-3d715221ffa2\"},{\"content\":{\"blockPath\":[\"SwarmSystem/Record\"],\"channel\":[2,1],\"dimensions\":[9,27],\"domain\":\"SwarmSystem/Record\",\"lineColor\":\"#64d413\",\"parentID\":5316,\"plots\":[1],\"port\":7,\"sid\":[\"\"],\"signalID\":5468,\"signalName\":\"raw\"},\"type\":\"RecordBlkView.Signal\",\"uuid\":\"d1c9b1c5-7922-4d35-9452-702d8af0ce12\"},{\"content\":{\"blockPath\":[\"SwarmSystem/Record\"],\"channel\":[3,1],\"dimensions\":[9,27],\"domain\":\"SwarmSystem/Record\",\"lineColor\":\"#ff13a6\",\"parentID\":5316,\"plots\":[1],\"port\":7,\"sid\":[\"\"],\"signalID\":5469,\"signalName\":\"raw\"},\"type\":\"RecordBlkView.Signal\",\"uuid\":\"cf3c0ccf-8cea-4fe4-8ffb-d5a13b982587\"},{\"content\":{\"blockPath\":[\"SwarmSystem/Record\"],\"channel\":[4,1],\"dimensions\":[9,27],\"domain\":\"SwarmSystem/Record\",\"lineColor\":\"#fe330a\",\"parentID\":5316,\"plots\":[1],\"port\":7,\"sid\":[\"\"],\"signalID\":5470,\"signalName\":\"raw\"},\"type\":\"RecordBlkView.Signal\",\"uuid\":\"95cac84b-7395-48ae-b8ab-1cb012228271\"},{\"content\":{\"blockPath\":[\"SwarmSystem/Record\"],\"channel\":[5,1],\"dimensions\":[9,27],\"domain\":\"SwarmSystem/Record\",\"lineColor\":\"#22b573\",\"parentID\":5316,\"plots\":[],\"port\":7,\"sid\":[\"\"],\"signalID\":5471,\"signalName\":\"raw\"},\"type\":\"RecordBlkView.Signal\",\"uuid\":\"24cd417c-ffe8-49b7-bf3a-8db87fe0e1cd\"},{\"content\":{\"blockPath\":[\"SwarmSystem/Record\"],\"channel\":[6,1],\"dimensions\":[9,27],\"domain\":\"SwarmSystem/Record\",\"lineColor\":\"#0072bd\",\"parentID\":5316,\"plots\":[],\"port\":7,\"sid\":[\"\"],\"signalID\":5472,\"signalName\":\"raw\"},\"type\":\"RecordBlkView.Signal\",\"uuid\":\"750def36-1cbb-4a04-b67f-ed672ce36f64\"},{\"content\":{\"blockPath\":[\"SwarmSystem/Record\"],\"channel\":[7,1],\"dimensions\":[9,27],\"domain\":\"SwarmSystem/Record\",\"lineColor\":\"#d95319\",\"parentID\":5316,\"plots\":[],\"port\":7,\"sid\":[\"\"],\"signalID\":5473,\"signalName\":\"raw\"},\"type\":\"RecordBlkView.Signal\",\"uuid\":\"072ce3e4-5565-495a-a291-f88ff924f5db\"},{\"content\":{\"blockPath\":[\"SwarmSystem/Record\"],\"channel\":[8,1],\"dimensions\":[9,27],\"domain\":\"SwarmSystem/Record\",\"lineColor\":\"#edb120\",\"parentID\":5316,\"plots\":[],\"port\":7,\"sid\":[\"\"],\"signalID\":5474,\"signalName\":\"raw\"},\"type\":\"RecordBlkView.Signal\",\"uuid\":\"d1d4c37c-1c56-4b81-9548-e63a4155ef2d\"},{\"content\":{\"blockPath\":[\"SwarmSystem/Record\"],\"channel\":[9,1],\"dimensions\":[9,27],\"domain\":\"SwarmSystem/Record\",\"lineColor\":\"#7e2f8e\",\"parentID\":5316,\"plots\":[],\"port\":7,\"sid\":[\"\"],\"signalID\":5475,\"signalName\":\"raw\"},\"type\":\"RecordBlkView.Signal\",\"uuid\":\"e5f1a0d9-b19a-42fb-ae1c-0ba4167ec223\"},{\"content\":{\"blockPath\":[\"SwarmSystem/Record\"],\"channel\":[1,2],\"dimensions\":[9,27],\"domain\":\"SwarmSystem/Record\",\"lineColor\":\"#77ac30\",\"parentID\":5316,\"plots\":[],\"port\":7,\"sid\":[\"\"],\"signalID\":5476,\"signalName\":\"raw\"},\"type\":\"RecordBlkView.Signal\",\"uuid\":\"8c5746fd-c460-49ad-b658-95073cb1f887\"},{\"content\":{\"blockPath\":[\"SwarmSystem/Record\"],\"channel\":[2,2],\"dimensions\":[9,27],\"domain\":\"SwarmSystem/Record\",\"lineColor\":\"#4dbeee\",\"parentID\":5316,\"plots\":[],\"port\":7,\"sid\":[\"\"],\"signalID\":5477,\"signalName\":\"raw\"},\"type\":\"RecordBlkView.Signal\",\"uuid\":\"fdb3c17c-be5d-40d1-be3a-6f4964b9f9e0\"},{\"content\":{\"blockPath\":[\"SwarmSystem/Record\"],\"channel\":[3,2],\"dimensions\":[9,27],\"domain\":\"SwarmSystem/Record\",\"lineColor\":\"#a2142f\",\"parentID\":5316,\"plots\":[],\"port\":7,\"sid\":[\"\"],\"signalID\":5478,\"signalName\":\"raw\"},\"type\":\"RecordBlkView.Signal\",\"uuid\":\"478dc21b-69e0-4be2-a0bb-3f29da1dacb8\"},{\"content\":{\"blockPath\":[\"SwarmSystem/Record\"],\"channel\":[4,2],\"dimensions\":[9,27],\"domain\":\"SwarmSystem/Record\",\"lineColor\":\"#139fff\",\"parentID\":5316,\"plots\":[],\"port\":7,\"sid\":[\"\"],\"signalID\":5479,\"signalName\":\"raw\"},\"type\":\"RecordBlkView.Signal\",\"uuid\":\"7997d4af-5b53-472e-900c-d64bec7012b9\"},{\"content\":{\"blockPath\":[\"SwarmSystem/Record\"],\"channel\":[5,2],\"dimensions\":[9,27],\"domain\":\"SwarmSystem/Record\",\"lineColor\":\"#ff6929\",\"parentID\":5316,\"plots\":[],\"port\":7,\"sid\":[\"\"],\"signalID\":5480,\"signalName\":\"raw\"},\"type\":\"RecordBlkView.Signal\",\"uuid\":\"41f6fbba-b91b-4400-ac3e-b2452eec2a63\"},{\"content\":{\"blockPath\":[\"SwarmSystem/Record\"],\"channel\":[6,2],\"dimensions\":[9,27],\"domain\":\"SwarmSystem/Record\",\"lineColor\":\"#b746ff\",\"parentID\":5316,\"plots\":[],\"port\":7,\"sid\":[\"\"],\"signalID\":5481,\"signalName\":\"raw\"},\"type\":\"RecordBlkView.Signal\",\"uuid\":\"a353d73c-5066-44fe-902a-82d37eea937f\"},{\"content\":{\"blockPath\":[\"SwarmSystem/Record\"],\"channel\":[7,2],\"dimensions\":[9,27],\"domain\":\"SwarmSystem/Record\",\"lineColor\":\"#64d413\",\"parentID\":5316,\"plots\":[],\"port\":7,\"sid\":[\"\"],\"signalID\":5482,\"signalName\":\"raw\"},\"type\":\"RecordBlkView.Signal\",\"uuid\":\"1ae862ca-7f25-4124-a9d3-587c34788160\"},{\"content\":{\"blockPath\":[\"SwarmSystem/Record\"],\"channel\":[8,2],\"dimensions\":[9,27],\"domain\":\"SwarmSystem/Record\",\"lineColor\":\"#ff13a6\",\"parentID\":5316,\"plots\":[],\"port\":7,\"sid\":[\"\"],\"signalID\":5483,\"signalName\":\"raw\"},\"type\":\"RecordBlkView.Signal\",\"uuid\":\"4cf9419c-80bd-4a76-a7ba-0fff32797268\"},{\"content\":{\"blockPath\":[\"SwarmSystem/Record\"],\"channel\":[9,2],\"dimensions\":[9,27],\"domain\":\"SwarmSystem/Record\",\"lineColor\":\"#fe330a\",\"parentID\":5316,\"plots\":[],\"port\":7,\"sid\":[\"\"],\"signalID\":5484,\"signalName\":\"raw\"},\"type\":\"RecordBlkView.Signal\",\"uuid\":\"5b3fab0e-ed23-4323-b880-e13279e71542\"},{\"content\":{\"blockPath\":[\"SwarmSystem/Record\"],\"channel\":[1,3],\"dimensions\":[9,27],\"domain\":\"SwarmSystem/Record\",\"lineColor\":\"#22b573\",\"parentID\":5316,\"plots\":[],\"port\":7,\"sid\":[\"\"],\"signalID\":5485,\"signalName\":\"raw\"},\"type\":\"RecordBlkView.Signal\",\"uuid\":\"22b98f87-9098-424e-89f9-e08a8f6092bb\"},{\"content\":{\"blockPath\":[\"SwarmSystem/Record\"],\"channel\":[2,3],\"dimensions\":[9,27],\"domain\":\"SwarmSystem/Record\",\"lineColor\":\"#0072bd\",\"parentID\":5316,\"plots\":[],\"port\":7,\"sid\":[\"\"],\"signalID\":5486,\"signalName\":\"raw\"},\"type\":\"RecordBlkView.Signal\",\"uuid\":\"59a9cb4c-b18a-4901-8d96-4cecda1c620e\"},{\"content\":{\"blockPath\":[\"SwarmSystem/Record\"],\"channel\":[3,3],\"dimensions\":[9,27],\"domain\":\"SwarmSystem/Record\",\"lineColor\":\"#d95319\",\"parentID\":5316,\"plots\":[],\"port\":7,\"sid\":[\"\"],\"signalID\":5487,\"signalName\":\"raw\"},\"type\":\"RecordBlkView.Signal\",\"uuid\":\"5e56a434-df78-4f98-bf27-aae9f08481ce\"},{\"content\":{\"blockPath\":[\"SwarmSystem/Record\"],\"channel\":[4,3],\"dimensions\":[9,27],\"domain\":\"SwarmSystem/Record\",\"lineColor\":\"#edb120\",\"parentID\":5316,\"plots\":[],\"port\":7,\"sid\":[\"\"],\"signalID\":5488,\"signalName\":\"raw\"},\"type\":\"RecordBlkView.Signal\",\"uuid\":\"954eb90a-1d2a-4c59-a74b-bd1342a1462d\"},{\"content\":{\"blockPath\":[\"SwarmSystem/Record\"],\"channel\":[5,3],\"dimensions\":[9,27],\"domain\":\"SwarmSystem/Record\",\"lineColor\":\"#7e2f8e\",\"parentID\":5316,\"plots\":[],\"port\":7,\"sid\":[\"\"],\"signalID\":5489,\"signalName\":\"raw\"},\"type\":\"RecordBlkView.Signal\",\"uuid\":\"db6e5093-5b99-4f4b-876f-81bc033ecbdc\"},{\"content\":{\"blockPath\":[\"SwarmSystem/Record\"],\"channel\":[6,3],\"dimensions\":[9,27],\"domain\":\"SwarmSystem/Record\",\"lineColor\":\"#77ac30\",\"parentID\":5316,\"plots\":[],\"port\":7,\"sid\":[\"\"],\"signalID\":5490,\"signalName\":\"raw\"},\"type\":\"RecordBlkView.Signal\",\"uuid\":\"eaf97de0-9854-45d6-a4d2-ddf92054e610\"},{\"content\":{\"blockPath\":[\"SwarmSystem/Record\"],\"channel\":[7,3],\"dimensions\":[9,27],\"domain\":\"SwarmSystem/Record\",\"lineColor\":\"#4dbeee\",\"parentID\":5316,\"plots\":[],\"port\":7,\"sid\":[\"\"],\"signalID\":5491,\"signalName\":\"raw\"},\"type\":\"RecordBlkView.Signal\",\"uuid\":\"45dcd67b-5ac5-43c6-a7b2-bfefaa8394e8\"},{\"content\":{\"blockPath\":[\"SwarmSystem/Record\"],\"channel\":[8,3],\"dimensions\":[9,27],\"domain\":\"SwarmSystem/Record\",\"lineColor\":\"#a2142f\",\"parentID\":5316,\"plots\":[],\"port\":7,\"sid\":[\"\"],\"signalID\":5492,\"signalName\":\"raw\"},\"type\":\"RecordBlkView.Signal\",\"uuid\":\"3a7ecf5d-a00f-440a-8978-6bc018acf980\"},{\"content\":{\"blockPath\":[\"SwarmSystem/Record\"],\"channel\":[9,3],\"dimensions\":[9,27],\"domain\":\"SwarmSystem/Record\",\"lineColor\":\"#139fff\",\"parentID\":5316,\"plots\":[],\"port\":7,\"sid\":[\"\"],\"signalID\":5493,\"signalName\":\"raw\"},\"type\":\"RecordBlkView.Signal\",\"uuid\":\"68a9e476-bf12-4ee3-b553-29dc50b59baf\"},{\"content\":{\"blockPath\":[\"SwarmSystem/Record\"],\"channel\":[1,4],\"dimensions\":[9,27],\"domain\":\"SwarmSystem/Record\",\"lineColor\":\"#ff6929\",\"parentID\":5316,\"plots\":[],\"port\":7,\"sid\":[\"\"],\"signalID\":5494,\"signalName\":\"raw\"},\"type\":\"RecordBlkView.Signal\",\"uuid\":\"3ae2635d-c000-49f2-b215-84937ffba5b0\"},{\"content\":{\"blockPath\":[\"SwarmSystem/Record\"],\"channel\":[2,4],\"dimensions\":[9,27],\"domain\":\"SwarmSystem/Record\",\"lineColor\":\"#b746ff\",\"parentID\":5316,\"plots\":[],\"port\":7,\"sid\":[\"\"],\"signalID\":5495,\"signalName\":\"raw\"},\"type\":\"RecordBlkView.Signal\",\"uuid\":\"1e2e37f6-f75f-4803-bd4f-89f457ee23ca\"},{\"content\":{\"blockPath\":[\"SwarmSystem/Record\"],\"channel\":[3,4],\"dimensions\":[9,27],\"domain\":\"SwarmSystem/Record\",\"lineColor\":\"#64d413\",\"parentID\":5316,\"plots\":[],\"port\":7,\"sid\":[\"\"],\"signalID\":5496,\"signalName\":\"raw\"},\"type\":\"RecordBlkView.Signal\",\"uuid\":\"7ef28c59-3235-470e-b972-6242da7d1d94\"},{\"content\":{\"blockPath\":[\"SwarmSystem/Record\"],\"channel\":[4,4],\"dimensions\":[9,27],\"domain\":\"SwarmSystem/Record\",\"lineColor\":\"#ff13a6\",\"parentID\":5316,\"plots\":[],\"port\":7,\"sid\":[\"\"],\"signalID\":5497,\"signalName\":\"raw\"},\"type\":\"RecordBlkView.Signal\",\"uuid\":\"1374445a-d0ff-4837-afe3-fb864b3f58be\"},{\"content\":{\"blockPath\":[\"SwarmSystem/Record\"],\"channel\":[5,4],\"dimensions\":[9,27],\"domain\":\"SwarmSystem/Record\",\"lineColor\":\"#fe330a\",\"parentID\":5316,\"plots\":[],\"port\":7,\"sid\":[\"\"],\"signalID\":5498,\"signalName\":\"raw\"},\"type\":\"RecordBlkView.Signal\",\"uuid\":\"66698a10-a466-45ce-ac3d-a9e8f67bb917\"},{\"content\":{\"blockPath\":[\"SwarmSystem/Record\"],\"channel\":[6,4],\"dimensions\":[9,27],\"domain\":\"SwarmSystem/Record\",\"lineColor\":\"#22b573\",\"parentID\":5316,\"plots\":[],\"port\":7,\"sid\":[\"\"],\"signalID\":5499,\"signalName\":\"raw\"},\"type\":\"RecordBlkView.Signal\",\"uuid\":\"b12b2d19-0ef0-47e4-a85f-1a450cd376aa\"},{\"content\":{\"blockPath\":[\"SwarmSystem/Record\"],\"channel\":[7,4],\"dimensions\":[9,27],\"domain\":\"SwarmSystem/Record\",\"lineColor\":\"#0072bd\",\"parentID\":5316,\"plots\":[],\"port\":7,\"sid\":[\"\"],\"signalID\":5500,\"signalName\":\"raw\"},\"type\":\"RecordBlkView.Signal\",\"uuid\":\"86574093-a69f-492d-852b-c398914a8912\"},{\"content\":{\"blockPath\":[\"SwarmSystem/Record\"],\"channel\":[8,4],\"dimensions\":[9,27],\"domain\":\"SwarmSystem/Record\",\"lineColor\":\"#d95319\",\"parentID\":5316,\"plots\":[],\"port\":7,\"sid\":[\"\"],\"signalID\":5501,\"signalName\":\"raw\"},\"type\":\"RecordBlkView.Signal\",\"uuid\":\"bfe3ad1f-0cf9-4e61-b65c-47e35e5eaf44\"},{\"content\":{\"blockPath\":[\"SwarmSystem/Record\"],\"channel\":[9,4],\"dimensions\":[9,27],\"domain\":\"SwarmSystem/Record\",\"lineColor\":\"#edb120\",\"parentID\":5316,\"plots\":[],\"port\":7,\"sid\":[\"\"],\"signalID\":5502,\"signalName\":\"raw\"},\"type\":\"RecordBlkView.Signal\",\"uuid\":\"49ff5a2a-b464-424c-8b4c-dda1d2553f7f\"},{\"content\":{\"blockPath\":[\"SwarmSystem/Record\"],\"channel\":[1,5],\"dimensions\":[9,27],\"domain\":\"SwarmSystem/Record\",\"lineColor\":\"#7e2f8e\",\"parentID\":5316,\"plots\":[],\"port\":7,\"sid\":[\"\"],\"signalID\":5503,\"signalName\":\"raw\"},\"type\":\"RecordBlkView.Signal\",\"uuid\":\"c4e99f48-844a-4de6-a09a-4f2fdf903c7e\"},{\"content\":{\"blockPath\":[\"SwarmSystem/Record\"],\"channel\":[2,5],\"dimensions\":[9,27],\"domain\":\"SwarmSystem/Record\",\"lineColor\":\"#77ac30\",\"parentID\":5316,\"plots\":[],\"port\":7,\"sid\":[\"\"],\"signalID\":5504,\"signalName\":\"raw\"},\"type\":\"RecordBlkView.Signal\",\"uuid\":\"e55cbbbb-5087-44cf-8a1e-8fc42acdf4e7\"},{\"content\":{\"blockPath\":[\"SwarmSystem/Record\"],\"channel\":[3,5],\"dimensions\":[9,27],\"domain\":\"SwarmSystem/Record\",\"lineColor\":\"#4dbeee\",\"parentID\":5316,\"plots\":[],\"port\":7,\"sid\":[\"\"],\"signalID\":5505,\"signalName\":\"raw\"},\"type\":\"RecordBlkView.Signal\",\"uuid\":\"2e8674d0-dfdb-4356-b367-2b6ecc9d32c9\"},{\"content\":{\"blockPath\":[\"SwarmSystem/Record\"],\"channel\":[4,5],\"dimensions\":[9,27],\"domain\":\"SwarmSystem/Record\",\"lineColor\":\"#a2142f\",\"parentID\":5316,\"plots\":[],\"port\":7,\"sid\":[\"\"],\"signalID\":5506,\"signalName\":\"raw\"},\"type\":\"RecordBlkView.Signal\",\"uuid\":\"d587078d-6982-45ff-85dd-83f0900e5da3\"},{\"content\":{\"blockPath\":[\"SwarmSystem/Record\"],\"channel\":[5,5],\"dimensions\":[9,27],\"domain\":\"SwarmSystem/Record\",\"lineColor\":\"#139fff\",\"parentID\":5316,\"plots\":[],\"port\":7,\"sid\":[\"\"],\"signalID\":5507,\"signalName\":\"raw\"},\"type\":\"RecordBlkView.Signal\",\"uuid\":\"35a6dd89-c1a0-46bd-8a30-b5a473f5a4d5\"},{\"content\":{\"blockPath\":[\"SwarmSystem/Record\"],\"channel\":[6,5],\"dimensions\":[9,27],\"domain\":\"SwarmSystem/Record\",\"lineColor\":\"#ff6929\",\"parentID\":5316,\"plots\":[],\"port\":7,\"sid\":[\"\"],\"signalID\":5508,\"signalName\":\"raw\"},\"type\":\"RecordBlkView.Signal\",\"uuid\":\"e2b28e5e-e07e-4b7e-bc2d-a1b5c1b6f299\"},{\"content\":{\"blockPath\":[\"SwarmSystem/Record\"],\"channel\":[7,5],\"dimensions\":[9,27],\"domain\":\"SwarmSystem/Record\",\"lineColor\":\"#b746ff\",\"parentID\":5316,\"plots\":[],\"port\":7,\"sid\":[\"\"],\"signalID\":5509,\"signalName\":\"raw\"},\"type\":\"RecordBlkView.Signal\",\"uuid\":\"4899b3d7-90d7-43eb-9d6b-e511eb3875e5\"},{\"content\":{\"blockPath\":[\"SwarmSystem/Record\"],\"channel\":[8,5],\"dimensions\":[9,27],\"domain\":\"SwarmSystem/Record\",\"lineColor\":\"#64d413\",\"parentID\":5316,\"plots\":[],\"port\":7,\"sid\":[\"\"],\"signalID\":5510,\"signalName\":\"raw\"},\"type\":\"RecordBlkView.Signal\",\"uuid\":\"14cc3bec-c18c-4723-95c6-bead96d635db\"},{\"content\":{\"blockPath\":[\"SwarmSystem/Record\"],\"channel\":[9,5],\"dimensions\":[9,27],\"domain\":\"SwarmSystem/Record\",\"lineColor\":\"#ff13a6\",\"parentID\":5316,\"plots\":[],\"port\":7,\"sid\":[\"\"],\"signalID\":5511,\"signalName\":\"raw\"},\"type\":\"RecordBlkView.Signal\",\"uuid\":\"6607904d-228c-4d63-94fd-b557e0d00352\"},{\"content\":{\"blockPath\":[\"SwarmSystem/Record\"],\"channel\":[1,6],\"dimensions\":[9,27],\"domain\":\"SwarmSystem/Record\",\"lineColor\":\"#fe330a\",\"parentID\":5316,\"plots\":[],\"port\":7,\"sid\":[\"\"],\"signalID\":5512,\"signalName\":\"raw\"},\"type\":\"RecordBlkView.Signal\",\"uuid\":\"76ba8069-469c-4d84-a53b-85b15d2290dc\"},{\"content\":{\"blockPath\":[\"SwarmSystem/Record\"],\"channel\":[2,6],\"dimensions\":[9,27],\"domain\":\"SwarmSystem/Record\",\"lineColor\":\"#22b573\",\"parentID\":5316,\"plots\":[],\"port\":7,\"sid\":[\"\"],\"signalID\":5513,\"signalName\":\"raw\"},\"type\":\"RecordBlkView.Signal\",\"uuid\":\"2eabb93f-2174-4b85-96fc-7f6049e728d8\"},{\"content\":{\"blockPath\":[\"SwarmSystem/Record\"],\"channel\":[3,6],\"dimensions\":[9,27],\"domain\":\"SwarmSystem/Record\",\"lineColor\":\"#0072bd\",\"parentID\":5316,\"plots\":[],\"port\":7,\"sid\":[\"\"],\"signalID\":5514,\"signalName\":\"raw\"},\"type\":\"RecordBlkView.Signal\",\"uuid\":\"fa99d4c5-8246-49dd-b61b-e9ecdfe78192\"},{\"content\":{\"blockPath\":[\"SwarmSystem/Record\"],\"channel\":[4,6],\"dimensions\":[9,27],\"domain\":\"SwarmSystem/Record\",\"lineColor\":\"#d95319\",\"parentID\":5316,\"plots\":[],\"port\":7,\"sid\":[\"\"],\"signalID\":5515,\"signalName\":\"raw\"},\"type\":\"RecordBlkView.Signal\",\"uuid\":\"0bff6b16-f240-4fda-a3ca-899ca77fade6\"},{\"content\":{\"blockPath\":[\"SwarmSystem/Record\"],\"channel\":[5,6],\"dimensions\":[9,27],\"domain\":\"SwarmSystem/Record\",\"lineColor\":\"#edb120\",\"parentID\":5316,\"plots\":[],\"port\":7,\"sid\":[\"\"],\"signalID\":5516,\"signalName\":\"raw\"},\"type\":\"RecordBlkView.Signal\",\"uuid\":\"68e95b06-18c5-4e77-802a-7b979f1e5687\"},{\"content\":{\"blockPath\":[\"SwarmSystem/Record\"],\"channel\":[6,6],\"dimensions\":[9,27],\"domain\":\"SwarmSystem/Record\",\"lineColor\":\"#7e2f8e\",\"parentID\":5316,\"plots\":[],\"port\":7,\"sid\":[\"\"],\"signalID\":5517,\"signalName\":\"raw\"},\"type\":\"RecordBlkView.Signal\",\"uuid\":\"299b51d2-86e7-477b-8e35-adbc460f3d98\"},{\"content\":{\"blockPath\":[\"SwarmSystem/Record\"],\"channel\":[7,6],\"dimensions\":[9,27],\"domain\":\"SwarmSystem/Record\",\"lineColor\":\"#77ac30\",\"parentID\":5316,\"plots\":[],\"port\":7,\"sid\":[\"\"],\"signalID\":5518,\"signalName\":\"raw\"},\"type\":\"RecordBlkView.Signal\",\"uuid\":\"98a9fa35-4e3c-41c2-bf80-ffa430665349\"},{\"content\":{\"blockPath\":[\"SwarmSystem/Record\"],\"channel\":[8,6],\"dimensions\":[9,27],\"domain\":\"SwarmSystem/Record\",\"lineColor\":\"#4dbeee\",\"parentID\":5316,\"plots\":[],\"port\":7,\"sid\":[\"\"],\"signalID\":5519,\"signalName\":\"raw\"},\"type\":\"RecordBlkView.Signal\",\"uuid\":\"421b7ad7-9cc8-42e1-af3b-08cc6d5b188b\"},{\"content\":{\"blockPath\":[\"SwarmSystem/Record\"],\"channel\":[9,6],\"dimensions\":[9,27],\"domain\":\"SwarmSystem/Record\",\"lineColor\":\"#a2142f\",\"parentID\":5316,\"plots\":[],\"port\":7,\"sid\":[\"\"],\"signalID\":5520,\"signalName\":\"raw\"},\"type\":\"RecordBlkView.Signal\",\"uuid\":\"6c71df4f-7705-4433-a89e-d8879423f877\"},{\"content\":{\"blockPath\":[\"SwarmSystem/Record\"],\"channel\":[1,7],\"dimensions\":[9,27],\"domain\":\"SwarmSystem/Record\",\"lineColor\":\"#139fff\",\"parentID\":5316,\"plots\":[],\"port\":7,\"sid\":[\"\"],\"signalID\":5521,\"signalName\":\"raw\"},\"type\":\"RecordBlkView.Signal\",\"uuid\":\"9bd770ed-3a7d-4204-aad1-05cbf77dcb30\"},{\"content\":{\"blockPath\":[\"SwarmSystem/Record\"],\"channel\":[2,7],\"dimensions\":[9,27],\"domain\":\"SwarmSystem/Record\",\"lineColor\":\"#ff6929\",\"parentID\":5316,\"plots\":[],\"port\":7,\"sid\":[\"\"],\"signalID\":5522,\"signalName\":\"raw\"},\"type\":\"RecordBlkView.Signal\",\"uuid\":\"add3ab97-8ccd-46ea-be65-4daee102c008\"},{\"content\":{\"blockPath\":[\"SwarmSystem/Record\"],\"channel\":[3,7],\"dimensions\":[9,27],\"domain\":\"SwarmSystem/Record\",\"lineColor\":\"#b746ff\",\"parentID\":5316,\"plots\":[],\"port\":7,\"sid\":[\"\"],\"signalID\":5523,\"signalName\":\"raw\"},\"type\":\"RecordBlkView.Signal\",\"uuid\":\"b7f43a9e-c021-416b-8b11-9a18f1a5af3e\"},{\"content\":{\"blockPath\":[\"SwarmSystem/Record\"],\"channel\":[4,7],\"dimensions\":[9,27],\"domain\":\"SwarmSystem/Record\",\"lineColor\":\"#64d413\",\"parentID\":5316,\"plots\":[],\"port\":7,\"sid\":[\"\"],\"signalID\":5524,\"signalName\":\"raw\"},\"type\":\"RecordBlkView.Signal\",\"uuid\":\"7aa53a23-600e-44aa-a60b-d51f0f3de553\"},{\"content\":{\"blockPath\":[\"SwarmSystem/Record\"],\"channel\":[5,7],\"dimensions\":[9,27],\"domain\":\"SwarmSystem/Record\",\"lineColor\":\"#ff13a6\",\"parentID\":5316,\"plots\":[],\"port\":7,\"sid\":[\"\"],\"signalID\":5525,\"signalName\":\"raw\"},\"type\":\"RecordBlkView.Signal\",\"uuid\":\"46ee6250-64a8-4720-991f-9eefb7af237e\"},{\"content\":{\"blockPath\":[\"SwarmSystem/Record\"],\"channel\":[6,7],\"dimensions\":[9,27],\"domain\":\"SwarmSystem/Record\",\"lineColor\":\"#fe330a\",\"parentID\":5316,\"plots\":[],\"port\":7,\"sid\":[\"\"],\"signalID\":5526,\"signalName\":\"raw\"},\"type\":\"RecordBlkView.Signal\",\"uuid\":\"79c2bad5-ed86-4fd6-b616-68276c55598d\"},{\"content\":{\"blockPath\":[\"SwarmSystem/Record\"],\"channel\":[7,7],\"dimensions\":[9,27],\"domain\":\"SwarmSystem/Record\",\"lineColor\":\"#22b573\",\"parentID\":5316,\"plots\":[],\"port\":7,\"sid\":[\"\"],\"signalID\":5527,\"signalName\":\"raw\"},\"type\":\"RecordBlkView.Signal\",\"uuid\":\"0499331f-228d-48fd-a7e7-74a95ebfaaa8\"},{\"content\":{\"blockPath\":[\"SwarmSystem/Record\"],\"channel\":[8,7],\"dimensions\":[9,27],\"domain\":\"SwarmSystem/Record\",\"lineColor\":\"#0072bd\",\"parentID\":5316,\"plots\":[],\"port\":7,\"sid\":[\"\"],\"signalID\":5528,\"signalName\":\"raw\"},\"type\":\"RecordBlkView.Signal\",\"uuid\":\"2235e54c-3be9-4c7d-a2f3-ac43d79ed07f\"},{\"content\":{\"blockPath\":[\"SwarmSystem/Record\"],\"channel\":[9,7],\"dimensions\":[9,27],\"domain\":\"SwarmSystem/Record\",\"lineColor\":\"#d95319\",\"parentID\":5316,\"plots\":[],\"port\":7,\"sid\":[\"\"],\"signalID\":5529,\"signalName\":\"raw\"},\"type\":\"RecordBlkView.Signal\",\"uuid\":\"03d9bcec-1ca3-47f1-b86b-bf0718195bfa\"},{\"content\":{\"blockPath\":[\"SwarmSystem/Record\"],\"channel\":[1,8],\"dimensions\":[9,27],\"domain\":\"SwarmSystem/Record\",\"lineColor\":\"#edb120\",\"parentID\":5316,\"plots\":[],\"port\":7,\"sid\":[\"\"],\"signalID\":5530,\"signalName\":\"raw\"},\"type\":\"RecordBlkView.Signal\",\"uuid\":\"06482c7f-50d5-4c8d-9bc0-ee9d17eb0368\"},{\"content\":{\"blockPath\":[\"SwarmSystem/Record\"],\"channel\":[2,8],\"dimensions\":[9,27],\"domain\":\"SwarmSystem/Record\",\"lineColor\":\"#7e2f8e\",\"parentID\":5316,\"plots\":[],\"port\":7,\"sid\":[\"\"],\"signalID\":5531,\"signalName\":\"raw\"},\"type\":\"RecordBlkView.Signal\",\"uuid\":\"5b019024-86d6-4d79-aaf7-bf4e68172aae\"},{\"content\":{\"blockPath\":[\"SwarmSystem/Record\"],\"channel\":[3,8],\"dimensions\":[9,27],\"domain\":\"SwarmSystem/Record\",\"lineColor\":\"#77ac30\",\"parentID\":5316,\"plots\":[],\"port\":7,\"sid\":[\"\"],\"signalID\":5532,\"signalName\":\"raw\"},\"type\":\"RecordBlkView.Signal\",\"uuid\":\"aadc48c8-d9c7-4673-86cc-a7f04b5cd082\"},{\"content\":{\"blockPath\":[\"SwarmSystem/Record\"],\"channel\":[4,8],\"dimensions\":[9,27],\"domain\":\"SwarmSystem/Record\",\"lineColor\":\"#4dbeee\",\"parentID\":5316,\"plots\":[],\"port\":7,\"sid\":[\"\"],\"signalID\":5533,\"signalName\":\"raw\"},\"type\":\"RecordBlkView.Signal\",\"uuid\":\"cd598d13-2a83-4480-9704-b26cc7e0d2a1\"},{\"content\":{\"blockPath\":[\"SwarmSystem/Record\"],\"channel\":[5,8],\"dimensions\":[9,27],\"domain\":\"SwarmSystem/Record\",\"lineColor\":\"#a2142f\",\"parentID\":5316,\"plots\":[],\"port\":7,\"sid\":[\"\"],\"signalID\":5534,\"signalName\":\"raw\"},\"type\":\"RecordBlkView.Signal\",\"uuid\":\"10f9658f-02d8-4905-9fa8-a54cd1563c50\"},{\"content\":{\"blockPath\":[\"SwarmSystem/Record\"],\"channel\":[6,8],\"dimensions\":[9,27],\"domain\":\"SwarmSystem/Record\",\"lineColor\":\"#139fff\",\"parentID\":5316,\"plots\":[],\"port\":7,\"sid\":[\"\"],\"signalID\":5535,\"signalName\":\"raw\"},\"type\":\"RecordBlkView.Signal\",\"uuid\":\"d3efb2e0-3c23-43a6-b45b-07446e0576d1\"},{\"content\":{\"blockPath\":[\"SwarmSystem/Record\"],\"channel\":[7,8],\"dimensions\":[9,27],\"domain\":\"SwarmSystem/Record\",\"lineColor\":\"#ff6929\",\"parentID\":5316,\"plots\":[],\"port\":7,\"sid\":[\"\"],\"signalID\":5536,\"signalName\":\"raw\"},\"type\":\"RecordBlkView.Signal\",\"uuid\":\"a0d9abcf-2f90-43f6-911c-64f1df9ac7dc\"},{\"content\":{\"blockPath\":[\"SwarmSystem/Record\"],\"channel\":[8,8],\"dimensions\":[9,27],\"domain\":\"SwarmSystem/Record\",\"lineColor\":\"#b746ff\",\"parentID\":5316,\"plots\":[],\"port\":7,\"sid\":[\"\"],\"signalID\":5537,\"signalName\":\"raw\"},\"type\":\"RecordBlkView.Signal\",\"uuid\":\"a40d90ce-eb51-4ac3-aa0a-c310564568ec\"},{\"content\":{\"blockPath\":[\"SwarmSystem/Record\"],\"channel\":[9,8],\"dimensions\":[9,27],\"domain\":\"SwarmSystem/Record\",\"lineColor\":\"#64d413\",\"parentID\":5316,\"plots\":[],\"port\":7,\"sid\":[\"\"],\"signalID\":5538,\"signalName\":\"raw\"},\"type\":\"RecordBlkView.Signal\",\"uuid\":\"6a990075-55e8-47d8-aee4-15e89ac8f887\"},{\"content\":{\"blockPath\":[\"SwarmSystem/Record\"],\"channel\":[1,9],\"dimensions\":[9,27],\"domain\":\"SwarmSystem/Record\",\"lineColor\":\"#ff13a6\",\"parentID\":5316,\"plots\":[],\"port\":7,\"sid\":[\"\"],\"signalID\":5539,\"signalName\":\"raw\"},\"type\":\"RecordBlkView.Signal\",\"uuid\":\"22cec1ac-bce0-4b7e-a8c0-a0aed959ceff\"},{\"content\":{\"blockPath\":[\"SwarmSystem/Record\"],\"channel\":[2,9],\"dimensions\":[9,27],\"domain\":\"SwarmSystem/Record\",\"lineColor\":\"#fe330a\",\"parentID\":5316,\"plots\":[],\"port\":7,\"sid\":[\"\"],\"signalID\":5540,\"signalName\":\"raw\"},\"type\":\"RecordBlkView.Signal\",\"uuid\":\"e417e0e4-1fed-4789-ab20-7da79675e49a\"},{\"content\":{\"blockPath\":[\"SwarmSystem/Record\"],\"channel\":[3,9],\"dimensions\":[9,27],\"domain\":\"SwarmSystem/Record\",\"lineColor\":\"#22b573\",\"parentID\":5316,\"plots\":[],\"port\":7,\"sid\":[\"\"],\"signalID\":5541,\"signalName\":\"raw\"},\"type\":\"RecordBlkView.Signal\",\"uuid\":\"89d98183-7782-453f-8871-819b686a0901\"},{\"content\":{\"blockPath\":[\"SwarmSystem/Record\"],\"channel\":[4,9],\"dimensions\":[9,27],\"domain\":\"SwarmSystem/Record\",\"lineColor\":\"#0072bd\",\"parentID\":5316,\"plots\":[],\"port\":7,\"sid\":[\"\"],\"signalID\":5542,\"signalName\":\"raw\"},\"type\":\"RecordBlkView.Signal\",\"uuid\":\"f8ddc551-f89f-4747-a117-0997fc6a317d\"},{\"content\":{\"blockPath\":[\"SwarmSystem/Record\"],\"channel\":[5,9],\"dimensions\":[9,27],\"domain\":\"SwarmSystem/Record\",\"lineColor\":\"#d95319\",\"parentID\":5316,\"plots\":[],\"port\":7,\"sid\":[\"\"],\"signalID\":5543,\"signalName\":\"raw\"},\"type\":\"RecordBlkView.Signal\",\"uuid\":\"3409709d-45bc-44ac-a7de-9358d64c27ca\"},{\"content\":{\"blockPath\":[\"SwarmSystem/Record\"],\"channel\":[6,9],\"dimensions\":[9,27],\"domain\":\"SwarmSystem/Record\",\"lineColor\":\"#edb120\",\"parentID\":5316,\"plots\":[],\"port\":7,\"sid\":[\"\"],\"signalID\":5544,\"signalName\":\"raw\"},\"type\":\"RecordBlkView.Signal\",\"uuid\":\"169c522f-6c75-4951-a5b6-b2ceac4f4aa5\"},{\"content\":{\"blockPath\":[\"SwarmSystem/Record\"],\"channel\":[7,9],\"dimensions\":[9,27],\"domain\":\"SwarmSystem/Record\",\"lineColor\":\"#7e2f8e\",\"parentID\":5316,\"plots\":[],\"port\":7,\"sid\":[\"\"],\"signalID\":5545,\"signalName\":\"raw\"},\"type\":\"RecordBlkView.Signal\",\"uuid\":\"1ea1ae06-5872-47a9-83b3-e05434b37856\"},{\"content\":{\"blockPath\":[\"SwarmSystem/Record\"],\"channel\":[8,9],\"dimensions\":[9,27],\"domain\":\"SwarmSystem/Record\",\"lineColor\":\"#77ac30\",\"parentID\":5316,\"plots\":[],\"port\":7,\"sid\":[\"\"],\"signalID\":5546,\"signalName\":\"raw\"},\"type\":\"RecordBlkView.Signal\",\"uuid\":\"9684a897-03e0-40da-9561-169d80368d0f\"},{\"content\":{\"blockPath\":[\"SwarmSystem/Record\"],\"channel\":[9,9],\"dimensions\":[9,27],\"domain\":\"SwarmSystem/Record\",\"lineColor\":\"#4dbeee\",\"parentID\":5316,\"plots\":[],\"port\":7,\"sid\":[\"\"],\"signalID\":5547,\"signalName\":\"raw\"},\"type\":\"RecordBlkView.Signal\",\"uuid\":\"3de90d31-2143-49b5-80b8-7c19b96c8177\"},{\"content\":{\"blockPath\":[\"SwarmSystem/Record\"],\"channel\":[1,10],\"dimensions\":[9,27],\"domain\":\"SwarmSystem/Record\",\"lineColor\":\"#a2142f\",\"parentID\":5316,\"plots\":[],\"port\":7,\"sid\":[\"\"],\"signalID\":5548,\"signalName\":\"raw\"},\"type\":\"RecordBlkView.Signal\",\"uuid\":\"d36105b2-d2ed-4e6e-be61-af0490851e88\"},{\"content\":{\"blockPath\":[\"SwarmSystem/Record\"],\"channel\":[2,10],\"dimensions\":[9,27],\"domain\":\"SwarmSystem/Record\",\"lineColor\":\"#139fff\",\"parentID\":5316,\"plots\":[],\"port\":7,\"sid\":[\"\"],\"signalID\":5549,\"signalName\":\"raw\"},\"type\":\"RecordBlkView.Signal\",\"uuid\":\"c90fd717-51fe-4147-bb54-96b328f0786d\"},{\"content\":{\"blockPath\":[\"SwarmSystem/Record\"],\"channel\":[3,10],\"dimensions\":[9,27],\"domain\":\"SwarmSystem/Record\",\"lineColor\":\"#ff6929\",\"parentID\":5316,\"plots\":[],\"port\":7,\"sid\":[\"\"],\"signalID\":5550,\"signalName\":\"raw\"},\"type\":\"RecordBlkView.Signal\",\"uuid\":\"71731f92-f311-4476-9352-dd4f9d451cda\"},{\"content\":{\"blockPath\":[\"SwarmSystem/Record\"],\"channel\":[4,10],\"dimensions\":[9,27],\"domain\":\"SwarmSystem/Record\",\"lineColor\":\"#b746ff\",\"parentID\":5316,\"plots\":[],\"port\":7,\"sid\":[\"\"],\"signalID\":5551,\"signalName\":\"raw\"},\"type\":\"RecordBlkView.Signal\",\"uuid\":\"f9c3afdb-70d2-4862-97eb-2d33c6e105b8\"},{\"content\":{\"blockPath\":[\"SwarmSystem/Record\"],\"channel\":[5,10],\"dimensions\":[9,27],\"domain\":\"SwarmSystem/Record\",\"lineColor\":\"#64d413\",\"parentID\":5316,\"plots\":[],\"port\":7,\"sid\":[\"\"],\"signalID\":5552,\"signalName\":\"raw\"},\"type\":\"RecordBlkView.Signal\",\"uuid\":\"b000d934-7917-46d4-9d70-84d1a97cc474\"},{\"content\":{\"blockPath\":[\"SwarmSystem/Record\"],\"channel\":[6,10],\"dimensions\":[9,27],\"domain\":\"SwarmSystem/Record\",\"lineColor\":\"#ff13a6\",\"parentID\":5316,\"plots\":[],\"port\":7,\"sid\":[\"\"],\"signalID\":5553,\"signalName\":\"raw\"},\"type\":\"RecordBlkView.Signal\",\"uuid\":\"9e3b5b98-9728-434d-a131-e2e2c851f1e4\"},{\"content\":{\"blockPath\":[\"SwarmSystem/Record\"],\"channel\":[7,10],\"dimensions\":[9,27],\"domain\":\"SwarmSystem/Record\",\"lineColor\":\"#fe330a\",\"parentID\":5316,\"plots\":[],\"port\":7,\"sid\":[\"\"],\"signalID\":5554,\"signalName\":\"raw\"},\"type\":\"RecordBlkView.Signal\",\"uuid\":\"2bceaf45-fa7e-46a8-89ea-0611ae6650be\"},{\"content\":{\"blockPath\":[\"SwarmSystem/Record\"],\"channel\":[8,10],\"dimensions\":[9,27],\"domain\":\"SwarmSystem/Record\",\"lineColor\":\"#22b573\",\"parentID\":5316,\"plots\":[],\"port\":7,\"sid\":[\"\"],\"signalID\":5555,\"signalName\":\"raw\"},\"type\":\"RecordBlkView.Signal\",\"uuid\":\"001c71a9-e88c-42bb-ba19-f7159d77e092\"},{\"content\":{\"blockPath\":[\"SwarmSystem/Record\"],\"channel\":[9,10],\"dimensions\":[9,27],\"domain\":\"SwarmSystem/Record\",\"lineColor\":\"#0072bd\",\"parentID\":5316,\"plots\":[],\"port\":7,\"sid\":[\"\"],\"signalID\":5556,\"signalName\":\"raw\"},\"type\":\"RecordBlkView.Signal\",\"uuid\":\"b66e9432-acdc-473c-9c8e-80669475e704\"},{\"content\":{\"blockPath\":[\"SwarmSystem/Record\"],\"channel\":[1,11],\"dimensions\":[9,27],\"domain\":\"SwarmSystem/Record\",\"lineColor\":\"#d95319\",\"parentID\":5316,\"plots\":[],\"port\":7,\"sid\":[\"\"],\"signalID\":5557,\"signalName\":\"raw\"},\"type\":\"RecordBlkView.Signal\",\"uuid\":\"9ec7974c-8c20-49aa-a1ca-079cee69de7c\"},{\"content\":{\"blockPath\":[\"SwarmSystem/Record\"],\"channel\":[2,11],\"dimensions\":[9,27],\"domain\":\"SwarmSystem/Record\",\"lineColor\":\"#edb120\",\"parentID\":5316,\"plots\":[],\"port\":7,\"sid\":[\"\"],\"signalID\":5558,\"signalName\":\"raw\"},\"type\":\"RecordBlkView.Signal\",\"uuid\":\"365d55d2-0649-478a-a343-5e828d14b696\"},{\"content\":{\"blockPath\":[\"SwarmSystem/Record\"],\"channel\":[3,11],\"dimensions\":[9,27],\"domain\":\"SwarmSystem/Record\",\"lineColor\":\"#7e2f8e\",\"parentID\":5316,\"plots\":[],\"port\":7,\"sid\":[\"\"],\"signalID\":5559,\"signalName\":\"raw\"},\"type\":\"RecordBlkView.Signal\",\"uuid\":\"1b94dff5-6997-47c4-bc94-3814f48c95fd\"},{\"content\":{\"blockPath\":[\"SwarmSystem/Record\"],\"channel\":[4,11],\"dimensions\":[9,27],\"domain\":\"SwarmSystem/Record\",\"lineColor\":\"#77ac30\",\"parentID\":5316,\"plots\":[],\"port\":7,\"sid\":[\"\"],\"signalID\":5560,\"signalName\":\"raw\"},\"type\":\"RecordBlkView.Signal\",\"uuid\":\"499cb207-773a-4356-af04-8f0c6822b2c0\"},{\"content\":{\"blockPath\":[\"SwarmSystem/Record\"],\"channel\":[5,11],\"dimensions\":[9,27],\"domain\":\"SwarmSystem/Record\",\"lineColor\":\"#4dbeee\",\"parentID\":5316,\"plots\":[],\"port\":7,\"sid\":[\"\"],\"signalID\":5561,\"signalName\":\"raw\"},\"type\":\"RecordBlkView.Signal\",\"uuid\":\"ceba3028-4bbc-44a4-91cf-3c15cede040d\"},{\"content\":{\"blockPath\":[\"SwarmSystem/Record\"],\"channel\":[6,11],\"dimensions\":[9,27],\"domain\":\"SwarmSystem/Record\",\"lineColor\":\"#a2142f\",\"parentID\":5316,\"plots\":[],\"port\":7,\"sid\":[\"\"],\"signalID\":5562,\"signalName\":\"raw\"},\"type\":\"RecordBlkView.Signal\",\"uuid\":\"b6732157-c6e2-4beb-863d-9fd1e7d4004e\"},{\"content\":{\"blockPath\":[\"SwarmSystem/Record\"],\"channel\":[7,11],\"dimensions\":[9,27],\"domain\":\"SwarmSystem/Record\",\"lineColor\":\"#139fff\",\"parentID\":5316,\"plots\":[],\"port\":7,\"sid\":[\"\"],\"signalID\":5563,\"signalName\":\"raw\"},\"type\":\"RecordBlkView.Signal\",\"uuid\":\"ec285d31-3e97-4f86-b957-90f6b82d260a\"},{\"content\":{\"blockPath\":[\"SwarmSystem/Record\"],\"channel\":[8,11],\"dimensions\":[9,27],\"domain\":\"SwarmSystem/Record\",\"lineColor\":\"#ff6929\",\"parentID\":5316,\"plots\":[],\"port\":7,\"sid\":[\"\"],\"signalID\":5564,\"signalName\":\"raw\"},\"type\":\"RecordBlkView.Signal\",\"uuid\":\"e686b741-1b14-47cb-aed2-e5a0cb797b6c\"},{\"content\":{\"blockPath\":[\"SwarmSystem/Record\"],\"channel\":[9,11],\"dimensions\":[9,27],\"domain\":\"SwarmSystem/Record\",\"lineColor\":\"#b746ff\",\"parentID\":5316,\"plots\":[],\"port\":7,\"sid\":[\"\"],\"signalID\":5565,\"signalName\":\"raw\"},\"type\":\"RecordBlkView.Signal\",\"uuid\":\"4c55bb36-f9b9-4d11-895d-8bfc17cf8189\"},{\"content\":{\"blockPath\":[\"SwarmSystem/Record\"],\"channel\":[1,12],\"dimensions\":[9,27],\"domain\":\"SwarmSystem/Record\",\"lineColor\":\"#64d413\",\"parentID\":5316,\"plots\":[],\"port\":7,\"sid\":[\"\"],\"signalID\":5566,\"signalName\":\"raw\"},\"type\":\"RecordBlkView.Signal\",\"uuid\":\"05ae6a31-08eb-4761-a420-ce6a1379057e\"},{\"content\":{\"blockPath\":[\"SwarmSystem/Record\"],\"channel\":[2,12],\"dimensions\":[9,27],\"domain\":\"SwarmSystem/Record\",\"lineColor\":\"#ff13a6\",\"parentID\":5316,\"plots\":[],\"port\":7,\"sid\":[\"\"],\"signalID\":5567,\"signalName\":\"raw\"},\"type\":\"RecordBlkView.Signal\",\"uuid\":\"28795891-c715-42bb-ae67-94445fdfe550\"},{\"content\":{\"blockPath\":[\"SwarmSystem/Record\"],\"channel\":[3,12],\"dimensions\":[9,27],\"domain\":\"SwarmSystem/Record\",\"lineColor\":\"#fe330a\",\"parentID\":5316,\"plots\":[],\"port\":7,\"sid\":[\"\"],\"signalID\":5568,\"signalName\":\"raw\"},\"type\":\"RecordBlkView.Signal\",\"uuid\":\"b5925154-90b5-4a91-b9b0-539055901367\"},{\"content\":{\"blockPath\":[\"SwarmSystem/Record\"],\"channel\":[4,12],\"dimensions\":[9,27],\"domain\":\"SwarmSystem/Record\",\"lineColor\":\"#22b573\",\"parentID\":5316,\"plots\":[],\"port\":7,\"sid\":[\"\"],\"signalID\":5569,\"signalName\":\"raw\"},\"type\":\"RecordBlkView.Signal\",\"uuid\":\"fcc62b7d-207e-4522-836b-eda9656ed690\"},{\"content\":{\"blockPath\":[\"SwarmSystem/Record\"],\"channel\":[5,12],\"dimensions\":[9,27],\"domain\":\"SwarmSystem/Record\",\"lineColor\":\"#0072bd\",\"parentID\":5316,\"plots\":[],\"port\":7,\"sid\":[\"\"],\"signalID\":5570,\"signalName\":\"raw\"},\"type\":\"RecordBlkView.Signal\",\"uuid\":\"e67bf605-f5ce-4282-b2f5-3a7c0180ba41\"},{\"content\":{\"blockPath\":[\"SwarmSystem/Record\"],\"channel\":[6,12],\"dimensions\":[9,27],\"domain\":\"SwarmSystem/Record\",\"lineColor\":\"#d95319\",\"parentID\":5316,\"plots\":[],\"port\":7,\"sid\":[\"\"],\"signalID\":5571,\"signalName\":\"raw\"},\"type\":\"RecordBlkView.Signal\",\"uuid\":\"71e42676-af3c-4b89-aba3-29b6b1ed9e01\"},{\"content\":{\"blockPath\":[\"SwarmSystem/Record\"],\"channel\":[7,12],\"dimensions\":[9,27],\"domain\":\"SwarmSystem/Record\",\"lineColor\":\"#edb120\",\"parentID\":5316,\"plots\":[],\"port\":7,\"sid\":[\"\"],\"signalID\":5572,\"signalName\":\"raw\"},\"type\":\"RecordBlkView.Signal\",\"uuid\":\"6963ecde-a100-48f1-98ae-28697ca8a4e9\"},{\"content\":{\"blockPath\":[\"SwarmSystem/Record\"],\"channel\":[8,12],\"dimensions\":[9,27],\"domain\":\"SwarmSystem/Record\",\"lineColor\":\"#7e2f8e\",\"parentID\":5316,\"plots\":[],\"port\":7,\"sid\":[\"\"],\"signalID\":5573,\"signalName\":\"raw\"},\"type\":\"RecordBlkView.Signal\",\"uuid\":\"16735379-5f1c-4614-bf1f-ddbde991eddd\"},{\"content\":{\"blockPath\":[\"SwarmSystem/Record\"],\"channel\":[9,12],\"dimensions\":[9,27],\"domain\":\"SwarmSystem/Record\",\"lineColor\":\"#77ac30\",\"parentID\":5316,\"plots\":[],\"port\":7,\"sid\":[\"\"],\"signalID\":5574,\"signalName\":\"raw\"},\"type\":\"RecordBlkView.Signal\",\"uuid\":\"1f5b8a6c-71a8-4e9a-bb95-cff4b8120fa9\"},{\"content\":{\"blockPath\":[\"SwarmSystem/Record\"],\"channel\":[1,13],\"dimensions\":[9,27],\"domain\":\"SwarmSystem/Record\",\"lineColor\":\"#4dbeee\",\"parentID\":5316,\"plots\":[],\"port\":7,\"sid\":[\"\"],\"signalID\":5575,\"signalName\":\"raw\"},\"type\":\"RecordBlkView.Signal\",\"uuid\":\"6c85d983-be47-467c-aefa-06e91522f6e0\"},{\"content\":{\"blockPath\":[\"SwarmSystem/Record\"],\"channel\":[2,13],\"dimensions\":[9,27],\"domain\":\"SwarmSystem/Record\",\"lineColor\":\"#a2142f\",\"parentID\":5316,\"plots\":[],\"port\":7,\"sid\":[\"\"],\"signalID\":5576,\"signalName\":\"raw\"},\"type\":\"RecordBlkView.Signal\",\"uuid\":\"d8667a35-cfe5-45f4-8730-1b76484eab0e\"},{\"content\":{\"blockPath\":[\"SwarmSystem/Record\"],\"channel\":[3,13],\"dimensions\":[9,27],\"domain\":\"SwarmSystem/Record\",\"lineColor\":\"#139fff\",\"parentID\":5316,\"plots\":[],\"port\":7,\"sid\":[\"\"],\"signalID\":5577,\"signalName\":\"raw\"},\"type\":\"RecordBlkView.Signal\",\"uuid\":\"aa8482a0-68d2-43dd-a7e2-b9ed22876dda\"},{\"content\":{\"blockPath\":[\"SwarmSystem/Record\"],\"channel\":[4,13],\"dimensions\":[9,27],\"domain\":\"SwarmSystem/Record\",\"lineColor\":\"#ff6929\",\"parentID\":5316,\"plots\":[],\"port\":7,\"sid\":[\"\"],\"signalID\":5578,\"signalName\":\"raw\"},\"type\":\"RecordBlkView.Signal\",\"uuid\":\"3c98bfae-dafc-44ee-8c7e-24e7e23093b4\"},{\"content\":{\"blockPath\":[\"SwarmSystem/Record\"],\"channel\":[5,13],\"dimensions\":[9,27],\"domain\":\"SwarmSystem/Record\",\"lineColor\":\"#b746ff\",\"parentID\":5316,\"plots\":[],\"port\":7,\"sid\":[\"\"],\"signalID\":5579,\"signalName\":\"raw\"},\"type\":\"RecordBlkView.Signal\",\"uuid\":\"7b968108-28eb-4218-98c8-d4e13b243a87\"},{\"content\":{\"blockPath\":[\"SwarmSystem/Record\"],\"channel\":[6,13],\"dimensions\":[9,27],\"domain\":\"SwarmSystem/Record\",\"lineColor\":\"#64d413\",\"parentID\":5316,\"plots\":[],\"port\":7,\"sid\":[\"\"],\"signalID\":5580,\"signalName\":\"raw\"},\"type\":\"RecordBlkView.Signal\",\"uuid\":\"ad1640ad-9da6-4bc8-8ba3-a016d59dc118\"},{\"content\":{\"blockPath\":[\"SwarmSystem/Record\"],\"channel\":[7,13],\"dimensions\":[9,27],\"domain\":\"SwarmSystem/Record\",\"lineColor\":\"#ff13a6\",\"parentID\":5316,\"plots\":[],\"port\":7,\"sid\":[\"\"],\"signalID\":5581,\"signalName\":\"raw\"},\"type\":\"RecordBlkView.Signal\",\"uuid\":\"eafd2cfb-b353-4f4f-a33d-0baa2c22dad5\"},{\"content\":{\"blockPath\":[\"SwarmSystem/Record\"],\"channel\":[8,13],\"dimensions\":[9,27],\"domain\":\"SwarmSystem/Record\",\"lineColor\":\"#fe330a\",\"parentID\":5316,\"plots\":[],\"port\":7,\"sid\":[\"\"],\"signalID\":5582,\"signalName\":\"raw\"},\"type\":\"RecordBlkView.Signal\",\"uuid\":\"9a87e9ec-6917-464c-bd47-401894a84609\"},{\"content\":{\"blockPath\":[\"SwarmSystem/Record\"],\"channel\":[9,13],\"dimensions\":[9,27],\"domain\":\"SwarmSystem/Record\",\"lineColor\":\"#22b573\",\"parentID\":5316,\"plots\":[],\"port\":7,\"sid\":[\"\"],\"signalID\":5583,\"signalName\":\"raw\"},\"type\":\"RecordBlkView.Signal\",\"uuid\":\"08cf5298-0a9e-4411-9603-aac32d16ac36\"},{\"content\":{\"blockPath\":[\"SwarmSystem/Record\"],\"channel\":[1,14],\"dimensions\":[9,27],\"domain\":\"SwarmSystem/Record\",\"lineColor\":\"#0072bd\",\"parentID\":5316,\"plots\":[],\"port\":7,\"sid\":[\"\"],\"signalID\":5584,\"signalName\":\"raw\"},\"type\":\"RecordBlkView.Signal\",\"uuid\":\"c0267805-3f1d-43ec-9ab1-576638ceaf48\"},{\"content\":{\"blockPath\":[\"SwarmSystem/Record\"],\"channel\":[2,14],\"dimensions\":[9,27],\"domain\":\"SwarmSystem/Record\",\"lineColor\":\"#d95319\",\"parentID\":5316,\"plots\":[],\"port\":7,\"sid\":[\"\"],\"signalID\":5585,\"signalName\":\"raw\"},\"type\":\"RecordBlkView.Signal\",\"uuid\":\"63668c38-523c-4e3d-8e6f-c0424a46ce72\"},{\"content\":{\"blockPath\":[\"SwarmSystem/Record\"],\"channel\":[3,14],\"dimensions\":[9,27],\"domain\":\"SwarmSystem/Record\",\"lineColor\":\"#edb120\",\"parentID\":5316,\"plots\":[],\"port\":7,\"sid\":[\"\"],\"signalID\":5586,\"signalName\":\"raw\"},\"type\":\"RecordBlkView.Signal\",\"uuid\":\"ef272bca-bcdc-40f0-9775-5bd16c5f065d\"},{\"content\":{\"blockPath\":[\"SwarmSystem/Record\"],\"channel\":[4,14],\"dimensions\":[9,27],\"domain\":\"SwarmSystem/Record\",\"lineColor\":\"#7e2f8e\",\"parentID\":5316,\"plots\":[],\"port\":7,\"sid\":[\"\"],\"signalID\":5587,\"signalName\":\"raw\"},\"type\":\"RecordBlkView.Signal\",\"uuid\":\"f1fe109f-29fc-4298-9b7d-0c09133c5553\"},{\"content\":{\"blockPath\":[\"SwarmSystem/Record\"],\"channel\":[5,14],\"dimensions\":[9,27],\"domain\":\"SwarmSystem/Record\",\"lineColor\":\"#77ac30\",\"parentID\":5316,\"plots\":[],\"port\":7,\"sid\":[\"\"],\"signalID\":5588,\"signalName\":\"raw\"},\"type\":\"RecordBlkView.Signal\",\"uuid\":\"bbb4b293-7588-479f-bfc1-64e4ce4ce0a7\"},{\"content\":{\"blockPath\":[\"SwarmSystem/Record\"],\"channel\":[6,14],\"dimensions\":[9,27],\"domain\":\"SwarmSystem/Record\",\"lineColor\":\"#4dbeee\",\"parentID\":5316,\"plots\":[],\"port\":7,\"sid\":[\"\"],\"signalID\":5589,\"signalName\":\"raw\"},\"type\":\"RecordBlkView.Signal\",\"uuid\":\"05c1b184-cf08-4c21-9978-0a484b2adf83\"},{\"content\":{\"blockPath\":[\"SwarmSystem/Record\"],\"channel\":[7,14],\"dimensions\":[9,27],\"domain\":\"SwarmSystem/Record\",\"lineColor\":\"#a2142f\",\"parentID\":5316,\"plots\":[],\"port\":7,\"sid\":[\"\"],\"signalID\":5590,\"signalName\":\"raw\"},\"type\":\"RecordBlkView.Signal\",\"uuid\":\"1aa166b7-daf6-4552-b3a8-fd8f12012642\"},{\"content\":{\"blockPath\":[\"SwarmSystem/Record\"],\"channel\":[8,14],\"dimensions\":[9,27],\"domain\":\"SwarmSystem/Record\",\"lineColor\":\"#139fff\",\"parentID\":5316,\"plots\":[],\"port\":7,\"sid\":[\"\"],\"signalID\":5591,\"signalName\":\"raw\"},\"type\":\"RecordBlkView.Signal\",\"uuid\":\"9f3a5371-d06e-46a8-b7ef-df2591f3f1d6\"},{\"content\":{\"blockPath\":[\"SwarmSystem/Record\"],\"channel\":[9,14],\"dimensions\":[9,27],\"domain\":\"SwarmSystem/Record\",\"lineColor\":\"#ff6929\",\"parentID\":5316,\"plots\":[],\"port\":7,\"sid\":[\"\"],\"signalID\":5592,\"signalName\":\"raw\"},\"type\":\"RecordBlkView.Signal\",\"uuid\":\"ea31c90c-935f-4d17-8e18-f346e31c315a\"},{\"content\":{\"blockPath\":[\"SwarmSystem/Record\"],\"channel\":[1,15],\"dimensions\":[9,27],\"domain\":\"SwarmSystem/Record\",\"lineColor\":\"#b746ff\",\"parentID\":5316,\"plots\":[],\"port\":7,\"sid\":[\"\"],\"signalID\":5593,\"signalName\":\"raw\"},\"type\":\"RecordBlkView.Signal\",\"uuid\":\"f3e2360d-18c9-4f72-bcbc-9075b655a046\"},{\"content\":{\"blockPath\":[\"SwarmSystem/Record\"],\"channel\":[2,15],\"dimensions\":[9,27],\"domain\":\"SwarmSystem/Record\",\"lineColor\":\"#64d413\",\"parentID\":5316,\"plots\":[],\"port\":7,\"sid\":[\"\"],\"signalID\":5594,\"signalName\":\"raw\"},\"type\":\"RecordBlkView.Signal\",\"uuid\":\"a4629307-606b-4c40-bd43-6e02a4ac3a26\"},{\"content\":{\"blockPath\":[\"SwarmSystem/Record\"],\"channel\":[3,15],\"dimensions\":[9,27],\"domain\":\"SwarmSystem/Record\",\"lineColor\":\"#ff13a6\",\"parentID\":5316,\"plots\":[],\"port\":7,\"sid\":[\"\"],\"signalID\":5595,\"signalName\":\"raw\"},\"type\":\"RecordBlkView.Signal\",\"uuid\":\"9a75a9bb-d4de-41c3-b59b-e63a040539f7\"},{\"content\":{\"blockPath\":[\"SwarmSystem/Record\"],\"channel\":[4,15],\"dimensions\":[9,27],\"domain\":\"SwarmSystem/Record\",\"lineColor\":\"#fe330a\",\"parentID\":5316,\"plots\":[],\"port\":7,\"sid\":[\"\"],\"signalID\":5596,\"signalName\":\"raw\"},\"type\":\"RecordBlkView.Signal\",\"uuid\":\"45b09e79-91f9-490e-94e5-c2a2449bc145\"},{\"content\":{\"blockPath\":[\"SwarmSystem/Record\"],\"channel\":[5,15],\"dimensions\":[9,27],\"domain\":\"SwarmSystem/Record\",\"lineColor\":\"#22b573\",\"parentID\":5316,\"plots\":[],\"port\":7,\"sid\":[\"\"],\"signalID\":5597,\"signalName\":\"raw\"},\"type\":\"RecordBlkView.Signal\",\"uuid\":\"0f87d2c0-ffa5-4e34-b3eb-9d71ce394912\"},{\"content\":{\"blockPath\":[\"SwarmSystem/Record\"],\"channel\":[6,15],\"dimensions\":[9,27],\"domain\":\"SwarmSystem/Record\",\"lineColor\":\"#0072bd\",\"parentID\":5316,\"plots\":[],\"port\":7,\"sid\":[\"\"],\"signalID\":5598,\"signalName\":\"raw\"},\"type\":\"RecordBlkView.Signal\",\"uuid\":\"05d18bb0-4349-497c-85e9-5fb8f5536843\"},{\"content\":{\"blockPath\":[\"SwarmSystem/Record\"],\"channel\":[7,15],\"dimensions\":[9,27],\"domain\":\"SwarmSystem/Record\",\"lineColor\":\"#d95319\",\"parentID\":5316,\"plots\":[],\"port\":7,\"sid\":[\"\"],\"signalID\":5599,\"signalName\":\"raw\"},\"type\":\"RecordBlkView.Signal\",\"uuid\":\"fa55df60-9290-4d42-93e4-1b2c6604b61d\"},{\"content\":{\"blockPath\":[\"SwarmSystem/Record\"],\"channel\":[8,15],\"dimensions\":[9,27],\"domain\":\"SwarmSystem/Record\",\"lineColor\":\"#edb120\",\"parentID\":5316,\"plots\":[],\"port\":7,\"sid\":[\"\"],\"signalID\":5600,\"signalName\":\"raw\"},\"type\":\"RecordBlkView.Signal\",\"uuid\":\"b6af0fcc-8794-4b65-abc9-14affa23310e\"},{\"content\":{\"blockPath\":[\"SwarmSystem/Record\"],\"channel\":[9,15],\"dimensions\":[9,27],\"domain\":\"SwarmSystem/Record\",\"lineColor\":\"#7e2f8e\",\"parentID\":5316,\"plots\":[],\"port\":7,\"sid\":[\"\"],\"signalID\":5601,\"signalName\":\"raw\"},\"type\":\"RecordBlkView.Signal\",\"uuid\":\"db6e9af7-c59f-4280-9d4e-59763401e897\"},{\"content\":{\"blockPath\":[\"SwarmSystem/Record\"],\"channel\":[1,16],\"dimensions\":[9,27],\"domain\":\"SwarmSystem/Record\",\"lineColor\":\"#77ac30\",\"parentID\":5316,\"plots\":[],\"port\":7,\"sid\":[\"\"],\"signalID\":5602,\"signalName\":\"raw\"},\"type\":\"RecordBlkView.Signal\",\"uuid\":\"b585394f-4abd-4c45-bf87-79a60d829825\"},{\"content\":{\"blockPath\":[\"SwarmSystem/Record\"],\"channel\":[2,16],\"dimensions\":[9,27],\"domain\":\"SwarmSystem/Record\",\"lineColor\":\"#4dbeee\",\"parentID\":5316,\"plots\":[],\"port\":7,\"sid\":[\"\"],\"signalID\":5603,\"signalName\":\"raw\"},\"type\":\"RecordBlkView.Signal\",\"uuid\":\"307bc659-74bf-4a2c-a0cd-67c788e55746\"},{\"content\":{\"blockPath\":[\"SwarmSystem/Record\"],\"channel\":[3,16],\"dimensions\":[9,27],\"domain\":\"SwarmSystem/Record\",\"lineColor\":\"#a2142f\",\"parentID\":5316,\"plots\":[],\"port\":7,\"sid\":[\"\"],\"signalID\":5604,\"signalName\":\"raw\"},\"type\":\"RecordBlkView.Signal\",\"uuid\":\"e4bf23c5-165e-4933-8520-efc6952592ee\"},{\"content\":{\"blockPath\":[\"SwarmSystem/Record\"],\"channel\":[4,16],\"dimensions\":[9,27],\"domain\":\"SwarmSystem/Record\",\"lineColor\":\"#139fff\",\"parentID\":5316,\"plots\":[],\"port\":7,\"sid\":[\"\"],\"signalID\":5605,\"signalName\":\"raw\"},\"type\":\"RecordBlkView.Signal\",\"uuid\":\"a4cc7b6c-3aef-42a2-8aa8-cf5a65bc81ae\"},{\"content\":{\"blockPath\":[\"SwarmSystem/Record\"],\"channel\":[5,16],\"dimensions\":[9,27],\"domain\":\"SwarmSystem/Record\",\"lineColor\":\"#ff6929\",\"parentID\":5316,\"plots\":[],\"port\":7,\"sid\":[\"\"],\"signalID\":5606,\"signalName\":\"raw\"},\"type\":\"RecordBlkView.Signal\",\"uuid\":\"463e8f61-0929-48a9-801f-0af90c388d3f\"},{\"content\":{\"blockPath\":[\"SwarmSystem/Record\"],\"channel\":[6,16],\"dimensions\":[9,27],\"domain\":\"SwarmSystem/Record\",\"lineColor\":\"#b746ff\",\"parentID\":5316,\"plots\":[],\"port\":7,\"sid\":[\"\"],\"signalID\":5607,\"signalName\":\"raw\"},\"type\":\"RecordBlkView.Signal\",\"uuid\":\"28c844b4-55a5-4bb0-a88c-802cb8074dfa\"},{\"content\":{\"blockPath\":[\"SwarmSystem/Record\"],\"channel\":[7,16],\"dimensions\":[9,27],\"domain\":\"SwarmSystem/Record\",\"lineColor\":\"#64d413\",\"parentID\":5316,\"plots\":[],\"port\":7,\"sid\":[\"\"],\"signalID\":5608,\"signalName\":\"raw\"},\"type\":\"RecordBlkView.Signal\",\"uuid\":\"6b336b20-5a33-41c9-9afd-c252cc97ca49\"},{\"content\":{\"blockPath\":[\"SwarmSystem/Record\"],\"channel\":[8,16],\"dimensions\":[9,27],\"domain\":\"SwarmSystem/Record\",\"lineColor\":\"#ff13a6\",\"parentID\":5316,\"plots\":[],\"port\":7,\"sid\":[\"\"],\"signalID\":5609,\"signalName\":\"raw\"},\"type\":\"RecordBlkView.Signal\",\"uuid\":\"911905b1-a8cd-4411-a92c-c8e49ec9956a\"},{\"content\":{\"blockPath\":[\"SwarmSystem/Record\"],\"channel\":[9,16],\"dimensions\":[9,27],\"domain\":\"SwarmSystem/Record\",\"lineColor\":\"#fe330a\",\"parentID\":5316,\"plots\":[],\"port\":7,\"sid\":[\"\"],\"signalID\":5610,\"signalName\":\"raw\"},\"type\":\"RecordBlkView.Signal\",\"uuid\":\"0009f29a-0cff-4748-99a2-27187899272f\"},{\"content\":{\"blockPath\":[\"SwarmSystem/Record\"],\"channel\":[1,17],\"dimensions\":[9,27],\"domain\":\"SwarmSystem/Record\",\"lineColor\":\"#22b573\",\"parentID\":5316,\"plots\":[],\"port\":7,\"sid\":[\"\"],\"signalID\":5611,\"signalName\":\"raw\"},\"type\":\"RecordBlkView.Signal\",\"uuid\":\"b5782b49-30b7-466a-bbd7-d763651607b9\"},{\"content\":{\"blockPath\":[\"SwarmSystem/Record\"],\"channel\":[2,17],\"dimensions\":[9,27],\"domain\":\"SwarmSystem/Record\",\"lineColor\":\"#0072bd\",\"parentID\":5316,\"plots\":[],\"port\":7,\"sid\":[\"\"],\"signalID\":5612,\"signalName\":\"raw\"},\"type\":\"RecordBlkView.Signal\",\"uuid\":\"56d55026-da2c-4abd-bc32-53cefb5fdc93\"},{\"content\":{\"blockPath\":[\"SwarmSystem/Record\"],\"channel\":[3,17],\"dimensions\":[9,27],\"domain\":\"SwarmSystem/Record\",\"lineColor\":\"#d95319\",\"parentID\":5316,\"plots\":[],\"port\":7,\"sid\":[\"\"],\"signalID\":5613,\"signalName\":\"raw\"},\"type\":\"RecordBlkView.Signal\",\"uuid\":\"198e10b0-a88e-4825-8413-4119f4e04308\"},{\"content\":{\"blockPath\":[\"SwarmSystem/Record\"],\"channel\":[4,17],\"dimensions\":[9,27],\"domain\":\"SwarmSystem/Record\",\"lineColor\":\"#edb120\",\"parentID\":5316,\"plots\":[],\"port\":7,\"sid\":[\"\"],\"signalID\":5614,\"signalName\":\"raw\"},\"type\":\"RecordBlkView.Signal\",\"uuid\":\"54d94818-9455-42a6-ba9b-53c81636eb18\"},{\"content\":{\"blockPath\":[\"SwarmSystem/Record\"],\"channel\":[5,17],\"dimensions\":[9,27],\"domain\":\"SwarmSystem/Record\",\"lineColor\":\"#7e2f8e\",\"parentID\":5316,\"plots\":[],\"port\":7,\"sid\":[\"\"],\"signalID\":5615,\"signalName\":\"raw\"},\"type\":\"RecordBlkView.Signal\",\"uuid\":\"ae48902f-250c-4e78-9866-83dd850afa10\"},{\"content\":{\"blockPath\":[\"SwarmSystem/Record\"],\"channel\":[6,17],\"dimensions\":[9,27],\"domain\":\"SwarmSystem/Record\",\"lineColor\":\"#77ac30\",\"parentID\":5316,\"plots\":[],\"port\":7,\"sid\":[\"\"],\"signalID\":5616,\"signalName\":\"raw\"},\"type\":\"RecordBlkView.Signal\",\"uuid\":\"96041d6f-22f2-459d-8ab0-f53695935723\"},{\"content\":{\"blockPath\":[\"SwarmSystem/Record\"],\"channel\":[7,17],\"dimensions\":[9,27],\"domain\":\"SwarmSystem/Record\",\"lineColor\":\"#4dbeee\",\"parentID\":5316,\"plots\":[],\"port\":7,\"sid\":[\"\"],\"signalID\":5617,\"signalName\":\"raw\"},\"type\":\"RecordBlkView.Signal\",\"uuid\":\"d3a2d438-3e90-439c-b394-463614fc5840\"},{\"content\":{\"blockPath\":[\"SwarmSystem/Record\"],\"channel\":[8,17],\"dimensions\":[9,27],\"domain\":\"SwarmSystem/Record\",\"lineColor\":\"#a2142f\",\"parentID\":5316,\"plots\":[],\"port\":7,\"sid\":[\"\"],\"signalID\":5618,\"signalName\":\"raw\"},\"type\":\"RecordBlkView.Signal\",\"uuid\":\"a7aca5a9-28a4-464f-b9f8-ae813f16efbe\"},{\"content\":{\"blockPath\":[\"SwarmSystem/Record\"],\"channel\":[9,17],\"dimensions\":[9,27],\"domain\":\"SwarmSystem/Record\",\"lineColor\":\"#139fff\",\"parentID\":5316,\"plots\":[],\"port\":7,\"sid\":[\"\"],\"signalID\":5619,\"signalName\":\"raw\"},\"type\":\"RecordBlkView.Signal\",\"uuid\":\"0e10734b-8b74-414a-8955-cfbb619e052c\"},{\"content\":{\"blockPath\":[\"SwarmSystem/Record\"],\"channel\":[1,18],\"dimensions\":[9,27],\"domain\":\"SwarmSystem/Record\",\"lineColor\":\"#ff6929\",\"parentID\":5316,\"plots\":[],\"port\":7,\"sid\":[\"\"],\"signalID\":5620,\"signalName\":\"raw\"},\"type\":\"RecordBlkView.Signal\",\"uuid\":\"f7ee97f4-24cb-45e0-934d-1c0bcfe4683b\"},{\"content\":{\"blockPath\":[\"SwarmSystem/Record\"],\"channel\":[2,18],\"dimensions\":[9,27],\"domain\":\"SwarmSystem/Record\",\"lineColor\":\"#b746ff\",\"parentID\":5316,\"plots\":[],\"port\":7,\"sid\":[\"\"],\"signalID\":5621,\"signalName\":\"raw\"},\"type\":\"RecordBlkView.Signal\",\"uuid\":\"86cc05c9-c44f-4b83-b6d1-878feadececa\"},{\"content\":{\"blockPath\":[\"SwarmSystem/Record\"],\"channel\":[3,18],\"dimensions\":[9,27],\"domain\":\"SwarmSystem/Record\",\"lineColor\":\"#64d413\",\"parentID\":5316,\"plots\":[],\"port\":7,\"sid\":[\"\"],\"signalID\":5622,\"signalName\":\"raw\"},\"type\":\"RecordBlkView.Signal\",\"uuid\":\"beebaf7a-c589-47c5-81e0-54fc9e9f0222\"},{\"content\":{\"blockPath\":[\"SwarmSystem/Record\"],\"channel\":[4,18],\"dimensions\":[9,27],\"domain\":\"SwarmSystem/Record\",\"lineColor\":\"#ff13a6\",\"parentID\":5316,\"plots\":[],\"port\":7,\"sid\":[\"\"],\"signalID\":5623,\"signalName\":\"raw\"},\"type\":\"RecordBlkView.Signal\",\"uuid\":\"5d2ece67-f197-40c9-8457-4e7187bdf865\"},{\"content\":{\"blockPath\":[\"SwarmSystem/Record\"],\"channel\":[5,18],\"dimensions\":[9,27],\"domain\":\"SwarmSystem/Record\",\"lineColor\":\"#fe330a\",\"parentID\":5316,\"plots\":[],\"port\":7,\"sid\":[\"\"],\"signalID\":5624,\"signalName\":\"raw\"},\"type\":\"RecordBlkView.Signal\",\"uuid\":\"97c9a15f-9c3c-4ff8-8c11-05dc024ec362\"},{\"content\":{\"blockPath\":[\"SwarmSystem/Record\"],\"channel\":[6,18],\"dimensions\":[9,27],\"domain\":\"SwarmSystem/Record\",\"lineColor\":\"#22b573\",\"parentID\":5316,\"plots\":[],\"port\":7,\"sid\":[\"\"],\"signalID\":5625,\"signalName\":\"raw\"},\"type\":\"RecordBlkView.Signal\",\"uuid\":\"f86da993-11de-42e3-ac1e-34ae9e56c9c0\"},{\"content\":{\"blockPath\":[\"SwarmSystem/Record\"],\"channel\":[7,18],\"dimensions\":[9,27],\"domain\":\"SwarmSystem/Record\",\"lineColor\":\"#0072bd\",\"parentID\":5316,\"plots\":[],\"port\":7,\"sid\":[\"\"],\"signalID\":5626,\"signalName\":\"raw\"},\"type\":\"RecordBlkView.Signal\",\"uuid\":\"e3e13aa5-7bd2-435c-978a-a73e46b487fa\"},{\"content\":{\"blockPath\":[\"SwarmSystem/Record\"],\"channel\":[8,18],\"dimensions\":[9,27],\"domain\":\"SwarmSystem/Record\",\"lineColor\":\"#d95319\",\"parentID\":5316,\"plots\":[],\"port\":7,\"sid\":[\"\"],\"signalID\":5627,\"signalName\":\"raw\"},\"type\":\"RecordBlkView.Signal\",\"uuid\":\"c4966d50-459b-4b3d-ae88-7a869fd0597a\"},{\"content\":{\"blockPath\":[\"SwarmSystem/Record\"],\"channel\":[9,18],\"dimensions\":[9,27],\"domain\":\"SwarmSystem/Record\",\"lineColor\":\"#edb120\",\"parentID\":5316,\"plots\":[],\"port\":7,\"sid\":[\"\"],\"signalID\":5628,\"signalName\":\"raw\"},\"type\":\"RecordBlkView.Signal\",\"uuid\":\"9d4104bd-3bd4-47b6-8f73-549feaf31aa3\"},{\"content\":{\"blockPath\":[\"SwarmSystem/Record\"],\"channel\":[1,19],\"dimensions\":[9,27],\"domain\":\"SwarmSystem/Record\",\"lineColor\":\"#7e2f8e\",\"parentID\":5316,\"plots\":[],\"port\":7,\"sid\":[\"\"],\"signalID\":5629,\"signalName\":\"raw\"},\"type\":\"RecordBlkView.Signal\",\"uuid\":\"e291cb05-d8be-4e96-98bc-4b97df6d9a77\"},{\"content\":{\"blockPath\":[\"SwarmSystem/Record\"],\"channel\":[2,19],\"dimensions\":[9,27],\"domain\":\"SwarmSystem/Record\",\"lineColor\":\"#77ac30\",\"parentID\":5316,\"plots\":[],\"port\":7,\"sid\":[\"\"],\"signalID\":5630,\"signalName\":\"raw\"},\"type\":\"RecordBlkView.Signal\",\"uuid\":\"592f892b-f362-452e-ac6e-417141da3f08\"},{\"content\":{\"blockPath\":[\"SwarmSystem/Record\"],\"channel\":[3,19],\"dimensions\":[9,27],\"domain\":\"SwarmSystem/Record\",\"lineColor\":\"#4dbeee\",\"parentID\":5316,\"plots\":[],\"port\":7,\"sid\":[\"\"],\"signalID\":5631,\"signalName\":\"raw\"},\"type\":\"RecordBlkView.Signal\",\"uuid\":\"89c54a47-2a90-4b37-90f1-ef7347283f5d\"},{\"content\":{\"blockPath\":[\"SwarmSystem/Record\"],\"channel\":[4,19],\"dimensions\":[9,27],\"domain\":\"SwarmSystem/Record\",\"lineColor\":\"#a2142f\",\"parentID\":5316,\"plots\":[],\"port\":7,\"sid\":[\"\"],\"signalID\":5632,\"signalName\":\"raw\"},\"type\":\"RecordBlkView.Signal\",\"uuid\":\"07d5533a-efc1-4f6e-a0d9-75d3d719cb39\"},{\"content\":{\"blockPath\":[\"SwarmSystem/Record\"],\"channel\":[5,19],\"dimensions\":[9,27],\"domain\":\"SwarmSystem/Record\",\"lineColor\":\"#139fff\",\"parentID\":5316,\"plots\":[],\"port\":7,\"sid\":[\"\"],\"signalID\":5633,\"signalName\":\"raw\"},\"type\":\"RecordBlkView.Signal\",\"uuid\":\"ccf434ca-0b43-4468-bf9a-5cf2671c2bdd\"},{\"content\":{\"blockPath\":[\"SwarmSystem/Record\"],\"channel\":[6,19],\"dimensions\":[9,27],\"domain\":\"SwarmSystem/Record\",\"lineColor\":\"#ff6929\",\"parentID\":5316,\"plots\":[],\"port\":7,\"sid\":[\"\"],\"signalID\":5634,\"signalName\":\"raw\"},\"type\":\"RecordBlkView.Signal\",\"uuid\":\"affec9b3-00fa-45f4-ad91-2e285c1f7c0e\"},{\"content\":{\"blockPath\":[\"SwarmSystem/Record\"],\"channel\":[7,19],\"dimensions\":[9,27],\"domain\":\"SwarmSystem/Record\",\"lineColor\":\"#b746ff\",\"parentID\":5316,\"plots\":[],\"port\":7,\"sid\":[\"\"],\"signalID\":5635,\"signalName\":\"raw\"},\"type\":\"RecordBlkView.Signal\",\"uuid\":\"0ed12bb4-a425-4c77-b1b2-a781e9786e33\"},{\"content\":{\"blockPath\":[\"SwarmSystem/Record\"],\"channel\":[8,19],\"dimensions\":[9,27],\"domain\":\"SwarmSystem/Record\",\"lineColor\":\"#64d413\",\"parentID\":5316,\"plots\":[],\"port\":7,\"sid\":[\"\"],\"signalID\":5636,\"signalName\":\"raw\"},\"type\":\"RecordBlkView.Signal\",\"uuid\":\"3e8b7b71-af3f-4c2c-bbf0-12b12377d3ac\"},{\"content\":{\"blockPath\":[\"SwarmSystem/Record\"],\"channel\":[9,19],\"dimensions\":[9,27],\"domain\":\"SwarmSystem/Record\",\"lineColor\":\"#ff13a6\",\"parentID\":5316,\"plots\":[],\"port\":7,\"sid\":[\"\"],\"signalID\":5637,\"signalName\":\"raw\"},\"type\":\"RecordBlkView.Signal\",\"uuid\":\"79e78254-ba45-4ea3-ad86-d2bb1ed71b09\"},{\"content\":{\"blockPath\":[\"SwarmSystem/Record\"],\"channel\":[1,20],\"dimensions\":[9,27],\"domain\":\"SwarmSystem/Record\",\"lineColor\":\"#fe330a\",\"parentID\":5316,\"plots\":[],\"port\":7,\"sid\":[\"\"],\"signalID\":5638,\"signalName\":\"raw\"},\"type\":\"RecordBlkView.Signal\",\"uuid\":\"28c0c523-99a3-4fbb-a9ad-4d346fc3ff0f\"},{\"content\":{\"blockPath\":[\"SwarmSystem/Record\"],\"channel\":[2,20],\"dimensions\":[9,27],\"domain\":\"SwarmSystem/Record\",\"lineColor\":\"#22b573\",\"parentID\":5316,\"plots\":[],\"port\":7,\"sid\":[\"\"],\"signalID\":5639,\"signalName\":\"raw\"},\"type\":\"RecordBlkView.Signal\",\"uuid\":\"a893b4fc-7a11-4a52-a7e6-223670679234\"},{\"content\":{\"blockPath\":[\"SwarmSystem/Record\"],\"channel\":[3,20],\"dimensions\":[9,27],\"domain\":\"SwarmSystem/Record\",\"lineColor\":\"#0072bd\",\"parentID\":5316,\"plots\":[],\"port\":7,\"sid\":[\"\"],\"signalID\":5640,\"signalName\":\"raw\"},\"type\":\"RecordBlkView.Signal\",\"uuid\":\"60b57615-7048-4f74-a570-8a956d845762\"},{\"content\":{\"blockPath\":[\"SwarmSystem/Record\"],\"channel\":[4,20],\"dimensions\":[9,27],\"domain\":\"SwarmSystem/Record\",\"lineColor\":\"#d95319\",\"parentID\":5316,\"plots\":[],\"port\":7,\"sid\":[\"\"],\"signalID\":5641,\"signalName\":\"raw\"},\"type\":\"RecordBlkView.Signal\",\"uuid\":\"ff5bdf49-9631-4fbc-848f-19c9160a2563\"},{\"content\":{\"blockPath\":[\"SwarmSystem/Record\"],\"channel\":[5,20],\"dimensions\":[9,27],\"domain\":\"SwarmSystem/Record\",\"lineColor\":\"#edb120\",\"parentID\":5316,\"plots\":[],\"port\":7,\"sid\":[\"\"],\"signalID\":5642,\"signalName\":\"raw\"},\"type\":\"RecordBlkView.Signal\",\"uuid\":\"26cad920-e0cb-438f-9afc-0ee86f735b8d\"},{\"content\":{\"blockPath\":[\"SwarmSystem/Record\"],\"channel\":[6,20],\"dimensions\":[9,27],\"domain\":\"SwarmSystem/Record\",\"lineColor\":\"#7e2f8e\",\"parentID\":5316,\"plots\":[],\"port\":7,\"sid\":[\"\"],\"signalID\":5643,\"signalName\":\"raw\"},\"type\":\"RecordBlkView.Signal\",\"uuid\":\"0eca7955-1271-49f2-8775-62632f3c1ee6\"},{\"content\":{\"blockPath\":[\"SwarmSystem/Record\"],\"channel\":[7,20],\"dimensions\":[9,27],\"domain\":\"SwarmSystem/Record\",\"lineColor\":\"#77ac30\",\"parentID\":5316,\"plots\":[],\"port\":7,\"sid\":[\"\"],\"signalID\":5644,\"signalName\":\"raw\"},\"type\":\"RecordBlkView.Signal\",\"uuid\":\"fe82f1e4-1537-4bb2-bb95-8c222c7b32c0\"},{\"content\":{\"blockPath\":[\"SwarmSystem/Record\"],\"channel\":[8,20],\"dimensions\":[9,27],\"domain\":\"SwarmSystem/Record\",\"lineColor\":\"#4dbeee\",\"parentID\":5316,\"plots\":[],\"port\":7,\"sid\":[\"\"],\"signalID\":5645,\"signalName\":\"raw\"},\"type\":\"RecordBlkView.Signal\",\"uuid\":\"6bdbd769-b40e-42b3-b39e-2886e15c7950\"},{\"content\":{\"blockPath\":[\"SwarmSystem/Record\"],\"channel\":[9,20],\"dimensions\":[9,27],\"domain\":\"SwarmSystem/Record\",\"lineColor\":\"#a2142f\",\"parentID\":5316,\"plots\":[],\"port\":7,\"sid\":[\"\"],\"signalID\":5646,\"signalName\":\"raw\"},\"type\":\"RecordBlkView.Signal\",\"uuid\":\"341adb04-30f1-4f74-897b-76798c7b310d\"},{\"content\":{\"blockPath\":[\"SwarmSystem/Record\"],\"channel\":[1,21],\"dimensions\":[9,27],\"domain\":\"SwarmSystem/Record\",\"lineColor\":\"#139fff\",\"parentID\":5316,\"plots\":[],\"port\":7,\"sid\":[\"\"],\"signalID\":5647,\"signalName\":\"raw\"},\"type\":\"RecordBlkView.Signal\",\"uuid\":\"6086de28-7ec7-4169-a36d-f3cd63bf4443\"},{\"content\":{\"blockPath\":[\"SwarmSystem/Record\"],\"channel\":[2,21],\"dimensions\":[9,27],\"domain\":\"SwarmSystem/Record\",\"lineColor\":\"#ff6929\",\"parentID\":5316,\"plots\":[],\"port\":7,\"sid\":[\"\"],\"signalID\":5648,\"signalName\":\"raw\"},\"type\":\"RecordBlkView.Signal\",\"uuid\":\"f6d1f03e-f904-4d10-9641-98c9ecae4867\"},{\"content\":{\"blockPath\":[\"SwarmSystem/Record\"],\"channel\":[3,21],\"dimensions\":[9,27],\"domain\":\"SwarmSystem/Record\",\"lineColor\":\"#b746ff\",\"parentID\":5316,\"plots\":[],\"port\":7,\"sid\":[\"\"],\"signalID\":5649,\"signalName\":\"raw\"},\"type\":\"RecordBlkView.Signal\",\"uuid\":\"25aeb26e-c025-4f78-8835-71ce4bd315e1\"},{\"content\":{\"blockPath\":[\"SwarmSystem/Record\"],\"channel\":[4,21],\"dimensions\":[9,27],\"domain\":\"SwarmSystem/Record\",\"lineColor\":\"#64d413\",\"parentID\":5316,\"plots\":[],\"port\":7,\"sid\":[\"\"],\"signalID\":5650,\"signalName\":\"raw\"},\"type\":\"RecordBlkView.Signal\",\"uuid\":\"b54b279b-2082-4554-a448-1f7e5bb02ca7\"},{\"content\":{\"blockPath\":[\"SwarmSystem/Record\"],\"channel\":[5,21],\"dimensions\":[9,27],\"domain\":\"SwarmSystem/Record\",\"lineColor\":\"#ff13a6\",\"parentID\":5316,\"plots\":[],\"port\":7,\"sid\":[\"\"],\"signalID\":5651,\"signalName\":\"raw\"},\"type\":\"RecordBlkView.Signal\",\"uuid\":\"8ba7a6dc-18c2-45ea-b211-2afcfe833c6c\"},{\"content\":{\"blockPath\":[\"SwarmSystem/Record\"],\"channel\":[6,21],\"dimensions\":[9,27],\"domain\":\"SwarmSystem/Record\",\"lineColor\":\"#fe330a\",\"parentID\":5316,\"plots\":[],\"port\":7,\"sid\":[\"\"],\"signalID\":5652,\"signalName\":\"raw\"},\"type\":\"RecordBlkView.Signal\",\"uuid\":\"b48604f6-c19d-4336-aa8c-bce8314a2e69\"},{\"content\":{\"blockPath\":[\"SwarmSystem/Record\"],\"channel\":[7,21],\"dimensions\":[9,27],\"domain\":\"SwarmSystem/Record\",\"lineColor\":\"#22b573\",\"parentID\":5316,\"plots\":[],\"port\":7,\"sid\":[\"\"],\"signalID\":5653,\"signalName\":\"raw\"},\"type\":\"RecordBlkView.Signal\",\"uuid\":\"0fa70ce8-184d-429a-8288-f352c5f8be00\"},{\"content\":{\"blockPath\":[\"SwarmSystem/Record\"],\"channel\":[8,21],\"dimensions\":[9,27],\"domain\":\"SwarmSystem/Record\",\"lineColor\":\"#0072bd\",\"parentID\":5316,\"plots\":[],\"port\":7,\"sid\":[\"\"],\"signalID\":5654,\"signalName\":\"raw\"},\"type\":\"RecordBlkView.Signal\",\"uuid\":\"bdbcc92b-eb88-47ea-a959-8cf99dda9c34\"},{\"content\":{\"blockPath\":[\"SwarmSystem/Record\"],\"channel\":[9,21],\"dimensions\":[9,27],\"domain\":\"SwarmSystem/Record\",\"lineColor\":\"#d95319\",\"parentID\":5316,\"plots\":[],\"port\":7,\"sid\":[\"\"],\"signalID\":5655,\"signalName\":\"raw\"},\"type\":\"RecordBlkView.Signal\",\"uuid\":\"7490b10d-95cc-45f7-a5a9-c4bbda7eca7b\"},{\"content\":{\"blockPath\":[\"SwarmSystem/Record\"],\"channel\":[1,22],\"dimensions\":[9,27],\"domain\":\"SwarmSystem/Record\",\"lineColor\":\"#edb120\",\"parentID\":5316,\"plots\":[],\"port\":7,\"sid\":[\"\"],\"signalID\":5656,\"signalName\":\"raw\"},\"type\":\"RecordBlkView.Signal\",\"uuid\":\"47fb374e-6782-45e2-ba6e-2f01ec3edc7f\"},{\"content\":{\"blockPath\":[\"SwarmSystem/Record\"],\"channel\":[2,22],\"dimensions\":[9,27],\"domain\":\"SwarmSystem/Record\",\"lineColor\":\"#7e2f8e\",\"parentID\":5316,\"plots\":[],\"port\":7,\"sid\":[\"\"],\"signalID\":5657,\"signalName\":\"raw\"},\"type\":\"RecordBlkView.Signal\",\"uuid\":\"873d6ba7-e651-4635-b545-06fc123de1b1\"},{\"content\":{\"blockPath\":[\"SwarmSystem/Record\"],\"channel\":[3,22],\"dimensions\":[9,27],\"domain\":\"SwarmSystem/Record\",\"lineColor\":\"#77ac30\",\"parentID\":5316,\"plots\":[],\"port\":7,\"sid\":[\"\"],\"signalID\":5658,\"signalName\":\"raw\"},\"type\":\"RecordBlkView.Signal\",\"uuid\":\"4043965e-c9db-4e63-91b6-4cecc652f90c\"},{\"content\":{\"blockPath\":[\"SwarmSystem/Record\"],\"channel\":[4,22],\"dimensions\":[9,27],\"domain\":\"SwarmSystem/Record\",\"lineColor\":\"#4dbeee\",\"parentID\":5316,\"plots\":[],\"port\":7,\"sid\":[\"\"],\"signalID\":5659,\"signalName\":\"raw\"},\"type\":\"RecordBlkView.Signal\",\"uuid\":\"c8b2940d-728c-4fa3-b81d-4419092c2111\"},{\"content\":{\"blockPath\":[\"SwarmSystem/Record\"],\"channel\":[5,22],\"dimensions\":[9,27],\"domain\":\"SwarmSystem/Record\",\"lineColor\":\"#a2142f\",\"parentID\":5316,\"plots\":[],\"port\":7,\"sid\":[\"\"],\"signalID\":5660,\"signalName\":\"raw\"},\"type\":\"RecordBlkView.Signal\",\"uuid\":\"2a08b9f9-3d55-45fb-aadb-ac85bd1e5114\"},{\"content\":{\"blockPath\":[\"SwarmSystem/Record\"],\"channel\":[6,22],\"dimensions\":[9,27],\"domain\":\"SwarmSystem/Record\",\"lineColor\":\"#139fff\",\"parentID\":5316,\"plots\":[],\"port\":7,\"sid\":[\"\"],\"signalID\":5661,\"signalName\":\"raw\"},\"type\":\"RecordBlkView.Signal\",\"uuid\":\"8c710db5-fb67-4a84-948f-6316ad0dc6eb\"},{\"content\":{\"blockPath\":[\"SwarmSystem/Record\"],\"channel\":[7,22],\"dimensions\":[9,27],\"domain\":\"SwarmSystem/Record\",\"lineColor\":\"#ff6929\",\"parentID\":5316,\"plots\":[],\"port\":7,\"sid\":[\"\"],\"signalID\":5662,\"signalName\":\"raw\"},\"type\":\"RecordBlkView.Signal\",\"uuid\":\"d5fa59a4-d499-43c8-9d77-f7804db095cb\"},{\"content\":{\"blockPath\":[\"SwarmSystem/Record\"],\"channel\":[8,22],\"dimensions\":[9,27],\"domain\":\"SwarmSystem/Record\",\"lineColor\":\"#b746ff\",\"parentID\":5316,\"plots\":[],\"port\":7,\"sid\":[\"\"],\"signalID\":5663,\"signalName\":\"raw\"},\"type\":\"RecordBlkView.Signal\",\"uuid\":\"80e167f9-23ea-4ff3-98da-978d5137ac80\"},{\"content\":{\"blockPath\":[\"SwarmSystem/Record\"],\"channel\":[9,22],\"dimensions\":[9,27],\"domain\":\"SwarmSystem/Record\",\"lineColor\":\"#64d413\",\"parentID\":5316,\"plots\":[],\"port\":7,\"sid\":[\"\"],\"signalID\":5664,\"signalName\":\"raw\"},\"type\":\"RecordBlkView.Signal\",\"uuid\":\"59d23566-24eb-47a8-9e78-e7c21509ebcd\"},{\"content\":{\"blockPath\":[\"SwarmSystem/Record\"],\"channel\":[1,23],\"dimensions\":[9,27],\"domain\":\"SwarmSystem/Record\",\"lineColor\":\"#ff13a6\",\"parentID\":5316,\"plots\":[],\"port\":7,\"sid\":[\"\"],\"signalID\":5665,\"signalName\":\"raw\"},\"type\":\"RecordBlkView.Signal\",\"uuid\":\"6d8e7601-7dd4-4452-a0e9-4cd4ddad2fec\"},{\"content\":{\"blockPath\":[\"SwarmSystem/Record\"],\"channel\":[2,23],\"dimensions\":[9,27],\"domain\":\"SwarmSystem/Record\",\"lineColor\":\"#fe330a\",\"parentID\":5316,\"plots\":[],\"port\":7,\"sid\":[\"\"],\"signalID\":5666,\"signalName\":\"raw\"},\"type\":\"RecordBlkView.Signal\",\"uuid\":\"5b941c02-6ced-4d54-b006-643b5f2159bc\"},{\"content\":{\"blockPath\":[\"SwarmSystem/Record\"],\"channel\":[3,23],\"dimensions\":[9,27],\"domain\":\"SwarmSystem/Record\",\"lineColor\":\"#22b573\",\"parentID\":5316,\"plots\":[],\"port\":7,\"sid\":[\"\"],\"signalID\":5667,\"signalName\":\"raw\"},\"type\":\"RecordBlkView.Signal\",\"uuid\":\"5eb2bc41-0adb-4818-8c49-c19476821a29\"},{\"content\":{\"blockPath\":[\"SwarmSystem/Record\"],\"channel\":[4,23],\"dimensions\":[9,27],\"domain\":\"SwarmSystem/Record\",\"lineColor\":\"#0072bd\",\"parentID\":5316,\"plots\":[],\"port\":7,\"sid\":[\"\"],\"signalID\":5668,\"signalName\":\"raw\"},\"type\":\"RecordBlkView.Signal\",\"uuid\":\"204cf1f2-47e8-471b-9a23-adcad6afbbbe\"},{\"content\":{\"blockPath\":[\"SwarmSystem/Record\"],\"channel\":[5,23],\"dimensions\":[9,27],\"domain\":\"SwarmSystem/Record\",\"lineColor\":\"#d95319\",\"parentID\":5316,\"plots\":[],\"port\":7,\"sid\":[\"\"],\"signalID\":5669,\"signalName\":\"raw\"},\"type\":\"RecordBlkView.Signal\",\"uuid\":\"c88084d6-793f-445f-b75f-d9adddbbd241\"},{\"content\":{\"blockPath\":[\"SwarmSystem/Record\"],\"channel\":[6,23],\"dimensions\":[9,27],\"domain\":\"SwarmSystem/Record\",\"lineColor\":\"#edb120\",\"parentID\":5316,\"plots\":[],\"port\":7,\"sid\":[\"\"],\"signalID\":5670,\"signalName\":\"raw\"},\"type\":\"RecordBlkView.Signal\",\"uuid\":\"00a399b4-1a16-4cb4-8155-af2767de7804\"},{\"content\":{\"blockPath\":[\"SwarmSystem/Record\"],\"channel\":[7,23],\"dimensions\":[9,27],\"domain\":\"SwarmSystem/Record\",\"lineColor\":\"#7e2f8e\",\"parentID\":5316,\"plots\":[],\"port\":7,\"sid\":[\"\"],\"signalID\":5671,\"signalName\":\"raw\"},\"type\":\"RecordBlkView.Signal\",\"uuid\":\"412f507e-ec0a-46b7-8e31-a86b903c00f3\"},{\"content\":{\"blockPath\":[\"SwarmSystem/Record\"],\"channel\":[8,23],\"dimensions\":[9,27],\"domain\":\"SwarmSystem/Record\",\"lineColor\":\"#77ac30\",\"parentID\":5316,\"plots\":[],\"port\":7,\"sid\":[\"\"],\"signalID\":5672,\"signalName\":\"raw\"},\"type\":\"RecordBlkView.Signal\",\"uuid\":\"f87a0c39-2661-42e8-90b4-9c541d085312\"},{\"content\":{\"blockPath\":[\"SwarmSystem/Record\"],\"channel\":[9,23],\"dimensions\":[9,27],\"domain\":\"SwarmSystem/Record\",\"lineColor\":\"#4dbeee\",\"parentID\":5316,\"plots\":[],\"port\":7,\"sid\":[\"\"],\"signalID\":5673,\"signalName\":\"raw\"},\"type\":\"RecordBlkView.Signal\",\"uuid\":\"e3b85b84-24c1-463e-8bde-66f0e001f733\"},{\"content\":{\"blockPath\":[\"SwarmSystem/Record\"],\"channel\":[1,24],\"dimensions\":[9,27],\"domain\":\"SwarmSystem/Record\",\"lineColor\":\"#a2142f\",\"parentID\":5316,\"plots\":[],\"port\":7,\"sid\":[\"\"],\"signalID\":5674,\"signalName\":\"raw\"},\"type\":\"RecordBlkView.Signal\",\"uuid\":\"b19a328c-a12f-4f32-aa21-04d396a167aa\"},{\"content\":{\"blockPath\":[\"SwarmSystem/Record\"],\"channel\":[2,24],\"dimensions\":[9,27],\"domain\":\"SwarmSystem/Record\",\"lineColor\":\"#139fff\",\"parentID\":5316,\"plots\":[],\"port\":7,\"sid\":[\"\"],\"signalID\":5675,\"signalName\":\"raw\"},\"type\":\"RecordBlkView.Signal\",\"uuid\":\"64ed193e-d71a-4dbd-b340-5712fc6f0a1f\"},{\"content\":{\"blockPath\":[\"SwarmSystem/Record\"],\"channel\":[3,24],\"dimensions\":[9,27],\"domain\":\"SwarmSystem/Record\",\"lineColor\":\"#ff6929\",\"parentID\":5316,\"plots\":[],\"port\":7,\"sid\":[\"\"],\"signalID\":5676,\"signalName\":\"raw\"},\"type\":\"RecordBlkView.Signal\",\"uuid\":\"69f8514a-409e-482d-be60-e3364820b8d0\"},{\"content\":{\"blockPath\":[\"SwarmSystem/Record\"],\"channel\":[4,24],\"dimensions\":[9,27],\"domain\":\"SwarmSystem/Record\",\"lineColor\":\"#b746ff\",\"parentID\":5316,\"plots\":[],\"port\":7,\"sid\":[\"\"],\"signalID\":5677,\"signalName\":\"raw\"},\"type\":\"RecordBlkView.Signal\",\"uuid\":\"1b7a330b-8f4b-470c-96d5-1f1d3deeca40\"},{\"content\":{\"blockPath\":[\"SwarmSystem/Record\"],\"channel\":[5,24],\"dimensions\":[9,27],\"domain\":\"SwarmSystem/Record\",\"lineColor\":\"#64d413\",\"parentID\":5316,\"plots\":[],\"port\":7,\"sid\":[\"\"],\"signalID\":5678,\"signalName\":\"raw\"},\"type\":\"RecordBlkView.Signal\",\"uuid\":\"6f43b1f8-8ee9-40f1-8126-a9f41acdf00d\"},{\"content\":{\"blockPath\":[\"SwarmSystem/Record\"],\"channel\":[6,24],\"dimensions\":[9,27],\"domain\":\"SwarmSystem/Record\",\"lineColor\":\"#ff13a6\",\"parentID\":5316,\"plots\":[],\"port\":7,\"sid\":[\"\"],\"signalID\":5679,\"signalName\":\"raw\"},\"type\":\"RecordBlkView.Signal\",\"uuid\":\"1d43bb8c-8754-498b-ad69-67074d983ff8\"},{\"content\":{\"blockPath\":[\"SwarmSystem/Record\"],\"channel\":[7,24],\"dimensions\":[9,27],\"domain\":\"SwarmSystem/Record\",\"lineColor\":\"#fe330a\",\"parentID\":5316,\"plots\":[],\"port\":7,\"sid\":[\"\"],\"signalID\":5680,\"signalName\":\"raw\"},\"type\":\"RecordBlkView.Signal\",\"uuid\":\"b920bdf1-2153-4328-a3e8-0919e6d487cc\"},{\"content\":{\"blockPath\":[\"SwarmSystem/Record\"],\"channel\":[8,24],\"dimensions\":[9,27],\"domain\":\"SwarmSystem/Record\",\"lineColor\":\"#22b573\",\"parentID\":5316,\"plots\":[],\"port\":7,\"sid\":[\"\"],\"signalID\":5681,\"signalName\":\"raw\"},\"type\":\"RecordBlkView.Signal\",\"uuid\":\"384358d0-2b69-4b5f-a285-7973b1cb90d9\"},{\"content\":{\"blockPath\":[\"SwarmSystem/Record\"],\"channel\":[9,24],\"dimensions\":[9,27],\"domain\":\"SwarmSystem/Record\",\"lineColor\":\"#0072bd\",\"parentID\":5316,\"plots\":[],\"port\":7,\"sid\":[\"\"],\"signalID\":5682,\"signalName\":\"raw\"},\"type\":\"RecordBlkView.Signal\",\"uuid\":\"1ae49cf3-53c5-4aff-bac8-de55f5ff5dc8\"},{\"content\":{\"blockPath\":[\"SwarmSystem/Record\"],\"channel\":[1,25],\"dimensions\":[9,27],\"domain\":\"SwarmSystem/Record\",\"lineColor\":\"#d95319\",\"parentID\":5316,\"plots\":[],\"port\":7,\"sid\":[\"\"],\"signalID\":5683,\"signalName\":\"raw\"},\"type\":\"RecordBlkView.Signal\",\"uuid\":\"46412b6e-d1af-4929-8fef-d2d825cd8338\"},{\"content\":{\"blockPath\":[\"SwarmSystem/Record\"],\"channel\":[2,25],\"dimensions\":[9,27],\"domain\":\"SwarmSystem/Record\",\"lineColor\":\"#edb120\",\"parentID\":5316,\"plots\":[],\"port\":7,\"sid\":[\"\"],\"signalID\":5684,\"signalName\":\"raw\"},\"type\":\"RecordBlkView.Signal\",\"uuid\":\"1bc81ef3-deca-4ae7-a1ae-ebbb40322130\"},{\"content\":{\"blockPath\":[\"SwarmSystem/Record\"],\"channel\":[3,25],\"dimensions\":[9,27],\"domain\":\"SwarmSystem/Record\",\"lineColor\":\"#7e2f8e\",\"parentID\":5316,\"plots\":[],\"port\":7,\"sid\":[\"\"],\"signalID\":5685,\"signalName\":\"raw\"},\"type\":\"RecordBlkView.Signal\",\"uuid\":\"51c32ef6-dcf9-40a6-990d-b7f4d9abef25\"},{\"content\":{\"blockPath\":[\"SwarmSystem/Record\"],\"channel\":[4,25],\"dimensions\":[9,27],\"domain\":\"SwarmSystem/Record\",\"lineColor\":\"#77ac30\",\"parentID\":5316,\"plots\":[],\"port\":7,\"sid\":[\"\"],\"signalID\":5686,\"signalName\":\"raw\"},\"type\":\"RecordBlkView.Signal\",\"uuid\":\"1db71703-7a1e-49c5-a645-0a181557bf69\"},{\"content\":{\"blockPath\":[\"SwarmSystem/Record\"],\"channel\":[5,25],\"dimensions\":[9,27],\"domain\":\"SwarmSystem/Record\",\"lineColor\":\"#4dbeee\",\"parentID\":5316,\"plots\":[],\"port\":7,\"sid\":[\"\"],\"signalID\":5687,\"signalName\":\"raw\"},\"type\":\"RecordBlkView.Signal\",\"uuid\":\"123d15cb-ac04-480a-81e3-bf0378da0ffd\"},{\"content\":{\"blockPath\":[\"SwarmSystem/Record\"],\"channel\":[6,25],\"dimensions\":[9,27],\"domain\":\"SwarmSystem/Record\",\"lineColor\":\"#a2142f\",\"parentID\":5316,\"plots\":[],\"port\":7,\"sid\":[\"\"],\"signalID\":5688,\"signalName\":\"raw\"},\"type\":\"RecordBlkView.Signal\",\"uuid\":\"b695e5ef-5414-4bd0-b54e-84f1adf29701\"},{\"content\":{\"blockPath\":[\"SwarmSystem/Record\"],\"channel\":[7,25],\"dimensions\":[9,27],\"domain\":\"SwarmSystem/Record\",\"lineColor\":\"#139fff\",\"parentID\":5316,\"plots\":[],\"port\":7,\"sid\":[\"\"],\"signalID\":5689,\"signalName\":\"raw\"},\"type\":\"RecordBlkView.Signal\",\"uuid\":\"00620521-0820-4502-b85f-124589c67ead\"},{\"content\":{\"blockPath\":[\"SwarmSystem/Record\"],\"channel\":[8,25],\"dimensions\":[9,27],\"domain\":\"SwarmSystem/Record\",\"lineColor\":\"#ff6929\",\"parentID\":5316,\"plots\":[],\"port\":7,\"sid\":[\"\"],\"signalID\":5690,\"signalName\":\"raw\"},\"type\":\"RecordBlkView.Signal\",\"uuid\":\"470fccc9-2ef1-49e4-a3a3-4688d1881477\"},{\"content\":{\"blockPath\":[\"SwarmSystem/Record\"],\"channel\":[9,25],\"dimensions\":[9,27],\"domain\":\"SwarmSystem/Record\",\"lineColor\":\"#b746ff\",\"parentID\":5316,\"plots\":[],\"port\":7,\"sid\":[\"\"],\"signalID\":5691,\"signalName\":\"raw\"},\"type\":\"RecordBlkView.Signal\",\"uuid\":\"c7f737af-a1a1-46ef-b6ec-c6e878180b25\"},{\"content\":{\"blockPath\":[\"SwarmSystem/Record\"],\"channel\":[1,26],\"dimensions\":[9,27],\"domain\":\"SwarmSystem/Record\",\"lineColor\":\"#64d413\",\"parentID\":5316,\"plots\":[],\"port\":7,\"sid\":[\"\"],\"signalID\":5692,\"signalName\":\"raw\"},\"type\":\"RecordBlkView.Signal\",\"uuid\":\"2e599a8a-0597-4197-a257-7597a830b618\"},{\"content\":{\"blockPath\":[\"SwarmSystem/Record\"],\"channel\":[2,26],\"dimensions\":[9,27],\"domain\":\"SwarmSystem/Record\",\"lineColor\":\"#ff13a6\",\"parentID\":5316,\"plots\":[],\"port\":7,\"sid\":[\"\"],\"signalID\":5693,\"signalName\":\"raw\"},\"type\":\"RecordBlkView.Signal\",\"uuid\":\"f0979043-8ff7-48d8-a087-f3c6a61efa09\"},{\"content\":{\"blockPath\":[\"SwarmSystem/Record\"],\"channel\":[3,26],\"dimensions\":[9,27],\"domain\":\"SwarmSystem/Record\",\"lineColor\":\"#fe330a\",\"parentID\":5316,\"plots\":[],\"port\":7,\"sid\":[\"\"],\"signalID\":5694,\"signalName\":\"raw\"},\"type\":\"RecordBlkView.Signal\",\"uuid\":\"8eb05389-a68b-4e58-8ec6-2c1f4c6a9f71\"},{\"content\":{\"blockPath\":[\"SwarmSystem/Record\"],\"channel\":[4,26],\"dimensions\":[9,27],\"domain\":\"SwarmSystem/Record\",\"lineColor\":\"#22b573\",\"parentID\":5316,\"plots\":[],\"port\":7,\"sid\":[\"\"],\"signalID\":5695,\"signalName\":\"raw\"},\"type\":\"RecordBlkView.Signal\",\"uuid\":\"f4c8abf3-d7af-438f-8eea-1ae43cb58301\"},{\"content\":{\"blockPath\":[\"SwarmSystem/Record\"],\"channel\":[5,26],\"dimensions\":[9,27],\"domain\":\"SwarmSystem/Record\",\"lineColor\":\"#0072bd\",\"parentID\":5316,\"plots\":[],\"port\":7,\"sid\":[\"\"],\"signalID\":5696,\"signalName\":\"raw\"},\"type\":\"RecordBlkView.Signal\",\"uuid\":\"72dc4de4-1b6e-4e73-961e-aa415c633a2a\"},{\"content\":{\"blockPath\":[\"SwarmSystem/Record\"],\"channel\":[6,26],\"dimensions\":[9,27],\"domain\":\"SwarmSystem/Record\",\"lineColor\":\"#d95319\",\"parentID\":5316,\"plots\":[],\"port\":7,\"sid\":[\"\"],\"signalID\":5697,\"signalName\":\"raw\"},\"type\":\"RecordBlkView.Signal\",\"uuid\":\"742c1e62-fe24-47ee-99b7-9f890b0c37c6\"},{\"content\":{\"blockPath\":[\"SwarmSystem/Record\"],\"channel\":[7,26],\"dimensions\":[9,27],\"domain\":\"SwarmSystem/Record\",\"lineColor\":\"#edb120\",\"parentID\":5316,\"plots\":[],\"port\":7,\"sid\":[\"\"],\"signalID\":5698,\"signalName\":\"raw\"},\"type\":\"RecordBlkView.Signal\",\"uuid\":\"3f5256b9-1c2f-4037-a952-cb13e47b07f4\"},{\"content\":{\"blockPath\":[\"SwarmSystem/Record\"],\"channel\":[8,26],\"dimensions\":[9,27],\"domain\":\"SwarmSystem/Record\",\"lineColor\":\"#7e2f8e\",\"parentID\":5316,\"plots\":[],\"port\":7,\"sid\":[\"\"],\"signalID\":5699,\"signalName\":\"raw\"},\"type\":\"RecordBlkView.Signal\",\"uuid\":\"4c21eabc-52b9-47ec-a3a7-67ce7149df44\"},{\"content\":{\"blockPath\":[\"SwarmSystem/Record\"],\"channel\":[9,26],\"dimensions\":[9,27],\"domain\":\"SwarmSystem/Record\",\"lineColor\":\"#77ac30\",\"parentID\":5316,\"plots\":[],\"port\":7,\"sid\":[\"\"],\"signalID\":5700,\"signalName\":\"raw\"},\"type\":\"RecordBlkView.Signal\",\"uuid\":\"8f8578fa-73d0-402e-a4dc-a74e681c607c\"},{\"content\":{\"blockPath\":[\"SwarmSystem/Record\"],\"channel\":[1,27],\"dimensions\":[9,27],\"domain\":\"SwarmSystem/Record\",\"lineColor\":\"#4dbeee\",\"parentID\":5316,\"plots\":[],\"port\":7,\"sid\":[\"\"],\"signalID\":5701,\"signalName\":\"raw\"},\"type\":\"RecordBlkView.Signal\",\"uuid\":\"899dfa49-0d39-47a0-ab31-bb14f939887f\"},{\"content\":{\"blockPath\":[\"SwarmSystem/Record\"],\"channel\":[2,27],\"dimensions\":[9,27],\"domain\":\"SwarmSystem/Record\",\"lineColor\":\"#a2142f\",\"parentID\":5316,\"plots\":[],\"port\":7,\"sid\":[\"\"],\"signalID\":5702,\"signalName\":\"raw\"},\"type\":\"RecordBlkView.Signal\",\"uuid\":\"b5971ffb-07d1-4201-9f66-9f308eef82c8\"},{\"content\":{\"blockPath\":[\"SwarmSystem/Record\"],\"channel\":[3,27],\"dimensions\":[9,27],\"domain\":\"SwarmSystem/Record\",\"lineColor\":\"#139fff\",\"parentID\":5316,\"plots\":[],\"port\":7,\"sid\":[\"\"],\"signalID\":5703,\"signalName\":\"raw\"},\"type\":\"RecordBlkView.Signal\",\"uuid\":\"321c96a8-efb8-4dd1-83ac-071062917a2e\"},{\"content\":{\"blockPath\":[\"SwarmSystem/Record\"],\"channel\":[4,27],\"dimensions\":[9,27],\"domain\":\"SwarmSystem/Record\",\"lineColor\":\"#ff6929\",\"parentID\":5316,\"plots\":[],\"port\":7,\"sid\":[\"\"],\"signalID\":5704,\"signalName\":\"raw\"},\"type\":\"RecordBlkView.Signal\",\"uuid\":\"8d785c2f-a176-4ab7-a6ab-8908202c87e9\"},{\"content\":{\"blockPath\":[\"SwarmSystem/Record\"],\"channel\":[5,27],\"dimensions\":[9,27],\"domain\":\"SwarmSystem/Record\",\"lineColor\":\"#b746ff\",\"parentID\":5316,\"plots\":[],\"port\":7,\"sid\":[\"\"],\"signalID\":5705,\"signalName\":\"raw\"},\"type\":\"RecordBlkView.Signal\",\"uuid\":\"0bbf1c1e-c907-456e-834d-aec6d941e099\"},{\"content\":{\"blockPath\":[\"SwarmSystem/Record\"],\"channel\":[6,27],\"dimensions\":[9,27],\"domain\":\"SwarmSystem/Record\",\"lineColor\":\"#64d413\",\"parentID\":5316,\"plots\":[],\"port\":7,\"sid\":[\"\"],\"signalID\":5706,\"signalName\":\"raw\"},\"type\":\"RecordBlkView.Signal\",\"uuid\":\"039da4b7-dd2b-42e0-be3f-660163e370a0\"},{\"content\":{\"blockPath\":[\"SwarmSystem/Record\"],\"channel\":[7,27],\"dimensions\":[9,27],\"domain\":\"SwarmSystem/Record\",\"lineColor\":\"#ff13a6\",\"parentID\":5316,\"plots\":[],\"port\":7,\"sid\":[\"\"],\"signalID\":5707,\"signalName\":\"raw\"},\"type\":\"RecordBlkView.Signal\",\"uuid\":\"2309f179-9f5f-4ac2-b5d3-86edc8efd489\"},{\"content\":{\"blockPath\":[\"SwarmSystem/Record\"],\"channel\":[8,27],\"dimensions\":[9,27],\"domain\":\"SwarmSystem/Record\",\"lineColor\":\"#fe330a\",\"parentID\":5316,\"plots\":[],\"port\":7,\"sid\":[\"\"],\"signalID\":5708,\"signalName\":\"raw\"},\"type\":\"RecordBlkView.Signal\",\"uuid\":\"327ea98b-90d6-4685-a14f-64fe5c654c6f\"},{\"content\":{\"blockPath\":[\"SwarmSystem/Record\"],\"channel\":[9,27],\"dimensions\":[9,27],\"domain\":\"SwarmSystem/Record\",\"lineColor\":\"#22b573\",\"parentID\":5316,\"plots\":[],\"port\":7,\"sid\":[\"\"],\"signalID\":5709,\"signalName\":\"raw\"},\"type\":\"RecordBlkView.Signal\",\"uuid\":\"c4f93c6a-36dc-454b-b8ce-24a506613e2e\"},{\"content\":{\"blockPath\":[\"SwarmSystem/Record\"],\"channel\":[2,1],\"dimensions\":[9,1],\"domain\":\"SwarmSystem/Record\",\"lineColor\":\"#0072bd\",\"parentID\":5321,\"plots\":[1],\"port\":8,\"sid\":[\"\"],\"signalID\":5710,\"signalName\":\"sat_order\"},\"type\":\"RecordBlkView.Signal\",\"uuid\":\"4e728d8e-6d49-4b84-9e05-c51608123bb8\"},{\"content\":{\"blockPath\":[\"SwarmSystem/Record\"],\"channel\":[3,1],\"dimensions\":[9,1],\"domain\":\"SwarmSystem/Record\",\"lineColor\":\"#d95319\",\"parentID\":5321,\"plots\":[1],\"port\":8,\"sid\":[\"\"],\"signalID\":5711,\"signalName\":\"sat_order\"},\"type\":\"RecordBlkView.Signal\",\"uuid\":\"2185c6c2-d48c-4e0f-a6b0-e985beee0342\"},{\"content\":{\"blockPath\":[\"SwarmSystem/Record\"],\"channel\":[4,1],\"dimensions\":[9,1],\"domain\":\"SwarmSystem/Record\",\"lineColor\":\"#edb120\",\"parentID\":5321,\"plots\":[1],\"port\":8,\"sid\":[\"\"],\"signalID\":5712,\"signalName\":\"sat_order\"},\"type\":\"RecordBlkView.Signal\",\"uuid\":\"de1f9839-eed0-436f-b072-14ea89dcd074\"},{\"content\":{\"blockPath\":[\"SwarmSystem/Record\"],\"channel\":[5,1],\"dimensions\":[9,1],\"domain\":\"SwarmSystem/Record\",\"lineColor\":\"#7e2f8e\",\"parentID\":5321,\"plots\":[],\"port\":8,\"sid\":[\"\"],\"signalID\":5713,\"signalName\":\"sat_order\"},\"type\":\"RecordBlkView.Signal\",\"uuid\":\"e6e1bbd1-c142-4148-a23f-fc91cb1712d0\"},{\"content\":{\"blockPath\":[\"SwarmSystem/Record\"],\"channel\":[6,1],\"dimensions\":[9,1],\"domain\":\"SwarmSystem/Record\",\"lineColor\":\"#77ac30\",\"parentID\":5321,\"plots\":[],\"port\":8,\"sid\":[\"\"],\"signalID\":5714,\"signalName\":\"sat_order\"},\"type\":\"RecordBlkView.Signal\",\"uuid\":\"6dee4bc3-eaac-4fb2-98ed-0695bf324555\"},{\"content\":{\"blockPath\":[\"SwarmSystem/Record\"],\"channel\":[7,1],\"dimensions\":[9,1],\"domain\":\"SwarmSystem/Record\",\"lineColor\":\"#4dbeee\",\"parentID\":5321,\"plots\":[],\"port\":8,\"sid\":[\"\"],\"signalID\":5715,\"signalName\":\"sat_order\"},\"type\":\"RecordBlkView.Signal\",\"uuid\":\"2520993f-c6b6-4a25-97e4-ba7de0378554\"},{\"content\":{\"blockPath\":[\"SwarmSystem/Record\"],\"channel\":[8,1],\"dimensions\":[9,1],\"domain\":\"SwarmSystem/Record\",\"lineColor\":\"#a2142f\",\"parentID\":5321,\"plots\":[],\"port\":8,\"sid\":[\"\"],\"signalID\":5716,\"signalName\":\"sat_order\"},\"type\":\"RecordBlkView.Signal\",\"uuid\":\"4b82d802-9dd5-4e0f-a3c4-9958c8ffbf28\"},{\"content\":{\"blockPath\":[\"SwarmSystem/Record\"],\"channel\":[9,1],\"dimensions\":[9,1],\"domain\":\"SwarmSystem/Record\",\"lineColor\":\"#139fff\",\"parentID\":5321,\"plots\":[],\"port\":8,\"sid\":[\"\"],\"signalID\":5717,\"signalName\":\"sat_order\"},\"type\":\"RecordBlkView.Signal\",\"uuid\":\"fd2709ae-c94e-47b1-821c-ffe629123c7e\"},{\"content\":{\"blockPath\":[\"SwarmSystem/Record\"],\"channel\":[2,1,1],\"dimensions\":[9,9,3],\"domain\":\"SwarmSystem/Record\",\"lineColor\":\"#ff6929\",\"parentID\":5326,\"plots\":[1],\"port\":9,\"sid\":[\"\"],\"signalID\":5718,\"signalName\":\"packed_tw\"},\"type\":\"RecordBlkView.Signal\",\"uuid\":\"84dd5838-bad2-49cf-8b11-285d16926702\"},{\"content\":{\"blockPath\":[\"SwarmSystem/Record\"],\"channel\":[3,1,1],\"dimensions\":[9,9,3],\"domain\":\"SwarmSystem/Record\",\"lineColor\":\"#b746ff\",\"parentID\":5326,\"plots\":[1],\"port\":9,\"sid\":[\"\"],\"signalID\":5719,\"signalName\":\"packed_tw\"},\"type\":\"RecordBlkView.Signal\",\"uuid\":\"0be3ae89-8ec6-4f03-b354-c746fd9898b6\"},{\"content\":{\"blockPath\":[\"SwarmSystem/Record\"],\"channel\":[4,1,1],\"dimensions\":[9,9,3],\"domain\":\"SwarmSystem/Record\",\"lineColor\":\"#64d413\",\"parentID\":5326,\"plots\":[1],\"port\":9,\"sid\":[\"\"],\"signalID\":5720,\"signalName\":\"packed_tw\"},\"type\":\"RecordBlkView.Signal\",\"uuid\":\"060705e1-b136-4b69-8691-d2d688d35651\"},{\"content\":{\"blockPath\":[\"SwarmSystem/Record\"],\"channel\":[5,1,1],\"dimensions\":[9,9,3],\"domain\":\"SwarmSystem/Record\",\"lineColor\":\"#ff13a6\",\"parentID\":5326,\"plots\":[],\"port\":9,\"sid\":[\"\"],\"signalID\":5721,\"signalName\":\"packed_tw\"},\"type\":\"RecordBlkView.Signal\",\"uuid\":\"8a847e39-f30b-48a4-8145-dd490a3b8208\"},{\"content\":{\"blockPath\":[\"SwarmSystem/Record\"],\"channel\":[6,1,1],\"dimensions\":[9,9,3],\"domain\":\"SwarmSystem/Record\",\"lineColor\":\"#fe330a\",\"parentID\":5326,\"plots\":[],\"port\":9,\"sid\":[\"\"],\"signalID\":5722,\"signalName\":\"packed_tw\"},\"type\":\"RecordBlkView.Signal\",\"uuid\":\"f8887852-47e6-49e7-8050-74002521b1d4\"},{\"content\":{\"blockPath\":[\"SwarmSystem/Record\"],\"channel\":[7,1,1],\"dimensions\":[9,9,3],\"domain\":\"SwarmSystem/Record\",\"lineColor\":\"#22b573\",\"parentID\":5326,\"plots\":[],\"port\":9,\"sid\":[\"\"],\"signalID\":5723,\"signalName\":\"packed_tw\"},\"type\":\"RecordBlkView.Signal\",\"uuid\":\"75585964-bbae-4d25-825d-844dae42e6d1\"},{\"content\":{\"blockPath\":[\"SwarmSystem/Record\"],\"channel\":[8,1,1],\"dimensions\":[9,9,3],\"domain\":\"SwarmSystem/Record\",\"lineColor\":\"#0072bd\",\"parentID\":5326,\"plots\":[],\"port\":9,\"sid\":[\"\"],\"signalID\":5724,\"signalName\":\"packed_tw\"},\"type\":\"RecordBlkView.Signal\",\"uuid\":\"0663be1f-7ac4-4102-b62f-c728ee34c14a\"},{\"content\":{\"blockPath\":[\"SwarmSystem/Record\"],\"channel\":[9,1,1],\"dimensions\":[9,9,3],\"domain\":\"SwarmSystem/Record\",\"lineColor\":\"#d95319\",\"parentID\":5326,\"plots\":[],\"port\":9,\"sid\":[\"\"],\"signalID\":5725,\"signalName\":\"packed_tw\"},\"type\":\"RecordBlkView.Signal\",\"uuid\":\"8b388d7b-8424-4e52-af25-72e0dd7e7bb1\"},{\"content\":{\"blockPath\":[\"SwarmSystem/Record\"],\"channel\":[1,2,1],\"dimensions\":[9,9,3],\"domain\":\"SwarmSystem/Record\",\"lineColor\":\"#edb120\",\"parentID\":5326,\"plots\":[],\"port\":9,\"sid\":[\"\"],\"signalID\":5726,\"signalName\":\"packed_tw\"},\"type\":\"RecordBlkView.Signal\",\"uuid\":\"97be5f36-0cfa-4b15-8f48-9fba958975b5\"},{\"content\":{\"blockPath\":[\"SwarmSystem/Record\"],\"channel\":[2,2,1],\"dimensions\":[9,9,3],\"domain\":\"SwarmSystem/Record\",\"lineColor\":\"#7e2f8e\",\"parentID\":5326,\"plots\":[],\"port\":9,\"sid\":[\"\"],\"signalID\":5727,\"signalName\":\"packed_tw\"},\"type\":\"RecordBlkView.Signal\",\"uuid\":\"558e15f4-ad70-43ce-b763-e953b55fcb6a\"},{\"content\":{\"blockPath\":[\"SwarmSystem/Record\"],\"channel\":[3,2,1],\"dimensions\":[9,9,3],\"domain\":\"SwarmSystem/Record\",\"lineColor\":\"#77ac30\",\"parentID\":5326,\"plots\":[],\"port\":9,\"sid\":[\"\"],\"signalID\":5728,\"signalName\":\"packed_tw\"},\"type\":\"RecordBlkView.Signal\",\"uuid\":\"50677295-ae58-465c-b3c0-7bdc2badd28a\"},{\"content\":{\"blockPath\":[\"SwarmSystem/Record\"],\"channel\":[4,2,1],\"dimensions\":[9,9,3],\"domain\":\"SwarmSystem/Record\",\"lineColor\":\"#4dbeee\",\"parentID\":5326,\"plots\":[],\"port\":9,\"sid\":[\"\"],\"signalID\":5729,\"signalName\":\"packed_tw\"},\"type\":\"RecordBlkView.Signal\",\"uuid\":\"d692952d-b1d3-454c-92e9-4adb65ba1832\"},{\"content\":{\"blockPath\":[\"SwarmSystem/Record\"],\"channel\":[5,2,1],\"dimensions\":[9,9,3],\"domain\":\"SwarmSystem/Record\",\"lineColor\":\"#a2142f\",\"parentID\":5326,\"plots\":[],\"port\":9,\"sid\":[\"\"],\"signalID\":5730,\"signalName\":\"packed_tw\"},\"type\":\"RecordBlkView.Signal\",\"uuid\":\"4172c00f-176d-4de0-a72c-e8b6c91ce7b6\"},{\"content\":{\"blockPath\":[\"SwarmSystem/Record\"],\"channel\":[6,2,1],\"dimensions\":[9,9,3],\"domain\":\"SwarmSystem/Record\",\"lineColor\":\"#139fff\",\"parentID\":5326,\"plots\":[],\"port\":9,\"sid\":[\"\"],\"signalID\":5731,\"signalName\":\"packed_tw\"},\"type\":\"RecordBlkView.Signal\",